simulink model "SimulinkAnalysisofCheetahTail"  (R2022a)
(part 5 of 21)

C = ft_9({B_cg_H,ITail,Mb,Mm,Mt,T_cg_H,dphi1,dphi2,dpsi1,dth1,dth2,dx,dy,dz,t10,t1003,t1005,t1006,t1007,t1008,t1009,t1013,t1014,t1015,t1016,t1017,t1018,t1019,t1020,t1023,t1029,t103,t1031,t1037,t1042,t1044,t1047,t105,t1050,t1051,t1052,t1053,t1054,t1059,t1060,t1064,t1065,t1067,t1068,t1071,t1072,t1073,t1074,t1075,t1076,t1077,t1078,t1079,t1082,t1084,t1086,t1088,t1097,t1099,t11,t1102,t1108,t1113,t1115,t1116,t1117,t1118,t1119,t1120,t1121,t1122,t1123,t1124,t1129,t1132,t1133,t1134,t1135,t1136,t1137,t1138,t1139,t1140,t1141,t1142,t1143,t1144,t1146,t1147,t1149,t1153,t1155,t1156,t1157,t1159,t1160,t1161,t1162,t1163,t1164,t1166,t1167,t1168,t1169,t1170,t1171,t1173,t1174,t1176,t1178,t1179,t1181,t1182,t1183,t1184,t1185,t1186,t1187,t1188,t1189,t1190,t1191,t1192,t1193,t1194,t1195,t1196,t1197,t120,t1200,t1201,t1202,t1203,t1205,t1206,t1211,t1212,t1213,t1214,t1215,t1220,t1221,t1223,t1224,t1225,t1228,t1229,t1230,t1234,t1236,t1237,t1240,t1242,t1243,t1244,t1245,t1246,t1247,t1248,t1250,t1251,t1252,t1253,t1255,t1256,t1260,t1261,t1262,t1263,t1264,t1265,t1268,t1271,t1275,t1280,t1283,t1285,t1291,t1296,t1299,t130,t1301,t1302,t1303,t1304,t1305,t1306,t1307,t1309,t1311,t1312,t1313,t1319,t1322,t1328,t1329,t1331,t1332,t1334,t1337,t1338,t1339,t134,t1341,t1343,t1344,t1345,t1348,t1349,t1352,t1354,t1355,t1356,t1357,t1358,t1360,t1361,t1362,t1365,t1366,t1368,t1370,t1371,t1373,t1374,t1378,t1379,t1380,t1381,t1382,t1383,t1384,t1386,t1388,t1389,t1391,t1393,t1394,t1395,t1396,t1397,t1399,t1402,t1403,t1405,t1406,t1407,t1410,t1412,t1413,t1414,t1415,t1416,t1418,t1421,t1422,t1423,t1426,t1427,t1430,t1431,t1433,t1435,t1438,t144,t1440,t1441,t1443,t1444,t1446,t1448,t1450,t1453,t1455,t1456,t1457,t1458,t1459,t1460,t1463,t1465,t1466,t1467,t1468,t1469,t1470,t1473,t1476,t1477,t1478,t1479,t1480,t1481,t1483,t1484,t1486,t1487,t1488,t1489,t1491,t1495,t1496,t1497,t1498,t15,t1500,t1505,t1506,t1508,t1509,t1510,t1512,t1513,t1516,t1517,t1518,t1521,t1523,t1525,t1526,t1528,t1529,t1531,t1535,t1540,t1543,t1544,t1546,t1548,t1549,t1550,t1551,t1552,t1553,t1555,t1558,t1562,t1563,t1565,t1566,t1567,t1568,t1574,t1575,t1578,t1579,t1581,t1582,t1585,t1586,t1587,t1589,t1590,t1591,t1593,t1594,t1595,t1596,t1597,t1598,t1599,t1601,t1602,t1605,t1606,t1609,t161,t1610,t1611,t1612,t1614,t1615,t1617,t1618,t1619,t162,t1620,t1621,t1622,t1623,t1624,t1627,t1628,t1630,t1631,t1632,t1633,t1634,t1635,t1636,t1637,t1639,t1640,t1641,t1642,t1643,t1644,t1645,t1646,t1649,t1651,t1652,t1653,t1654,t1655,t1656,t1657,t1658,t1659,t1660,t1661,t1663,t1664,t1665,t1667,t1668,t1669,t1671,t1672,t1674,t1675,t1676,t1677,t1678,t1679,t1680,t1681,t1682,t1683,t1684,t1685,t1686,t1687,t1688,t1689,t1690,t1691,t1692,t1693,t1694,t1695,t1696,t1698,t1699,t1700,t1701,t1702,t1703,t1705,t1706,t1711,t1716,t1718,t1719,t1720,t1721,t1722,t1723,t1725,t1726,t1727,t1729,t1730,t1731,t1734,t1735,t1736,t1737,t1739,t1740,t1741,t1742,t1743,t1744,t1745,t1746,t1747,t1748,t1749,t1750,t1751,t1752,t1753,t1755,t1756,t1758,t1759,t1761,t1762,t1763,t1764,t1765,t1770,t1771,t1774,t1777,t1778,t1779,t1780,t1781,t1782,t1783,t1784,t1785,t1786,t1787,t1788,t1789,t1790,t1791,t1792,t1798,t1799,t1800,t1801,t1802,t1806,t1809,t1810,t1813,t1814,t1815,t1817,t1820,t1821,t1822,t1823,t1824,t1826,t1828,t1829,t1830,t1831,t1832,t1836,t1839,t1840,t1841,t1843,t1844,t1845,t1846,t1847,t1849,t1851,t1852,t1853,t1855,t1857,t1858,t1859,t1860,t1862,t1863,t1864,t1865,t1866,t1867,t1869,t1870,t1871,t1872,t1874,t1875,t1878,t1880,t1881,t1882,t1883,t1884,t1885,t1887,t1888,t1890,t1891,t1893,t1894,t1895,t1896,t1898,t1899,t1900,t1902,t1904,t1905,t1906,t1907,t1908,t1909,t1910,t1911,t1912,t1914,t1915,t1916,t1917,t1918,t1921,t1922,t1924,t1928,t1929,t1930,t1931,t1932,t1937,t1938,t1939,t1940,t1941,t1942,t1943,t1945,t1946,t1947,t1948,t1949,t195,t1950,t1951,t1952,t1955,t1956,t1957,t1959,t1960,t1961,t1962,t1963,t1964,t1965,t1966,t1967,t1968,t1969,t197,t1970,t1971,t1973,t1974,t1975,t1976,t1977,t1978,t1979,t1980,t1981,t1982,t1983,t1985,t1986,t1989,t1990,t1991,t1993,t1995,t1997,t1998,t1999,t2,t2000,t2001,t2002,t2003,t2004,t2005,t2006,t2007,t2008,t2009,t2010,t2011,t2012,t2013,t2015,t2016,t2017,t2018,t2019,t2020,t2023,t2024,t2025,t2026,t2032,t2033,t2035,t2037,t2038,t2039,t2040,t2041,t2042,t2043,t2045,t2046,t2047,t2048,t2049,t2050,t2053,t2057,t2058,t2059,t2061,t2062,t2064,t2065,t2066,t2067,t2068,t2069,t2070,t2072,t2073,t2074,t2075,t2076,t2078,t2079,t2080,t2081,t2082,t2083,t2084,t2085,t2087,t2088,t2090,t2091,t2093,t2094,t2095,t2096,t2097,t2101,t2102,t2103,t2104,t2106,t2107,t2108,t2109,t2110,t2111,t2112,t2113,t2115,t2117,t2118,t2119,t2120,t2122,t2123,t2124,t2125,t2127,t2128,t2129,t2130,t2131,t2132,t2134,t2135,t2137,t2138,t2139,t214,t2141,t2143,t2144,t2147,t2148,t2150,t2151,t2152,t2153,t2154,t2155,t2156,t2157,t2158,t2160,t2161,t2162,t2165,t2169,t2170,t2171,t2172,t2173,t2174,t2175,t2176,t2177,t2178,t2179,t2181,t2182,t2183,t2186,t2188,t2189,t2190,t2191,t2192,t2193,t2194,t2195,t2196,t2197,t2198,t2199,t2200,t2201,t2202,t2203,t2205,t2206,t2208,t2209,t2210,t2211,t2212,t2213,t2214,t2215,t2216,t2217,t2218,t2219,t2220,t2221,t2222,t2223,t2224,t2225,t2227,t2229,t2230,t2232,t2233,t2234,t2235,t2236,t2237,t2238,t2240,t2241,t2242,t2243,t2244,t2245,t2246,t2247,t2248,t2249,t2250,t2251,t2252,t2253,t2254,t2255,t2257,t2258,t2259,t2260,t2262,t2263,t2268,t2269,t2270,t2271,t2274,t2276,t2277,t2279,t2281,t2282,t2284,t2285,t2286,t2287,t2288,t2289,t2290,t2293,t2294,t2296,t2298,t2299,t2303,t2304,t2305,t2307,t2308,t2312,t2313,t2316,t2317,t2318,t2319,t2320,t2321,t2322,t2323,t2324,t2325,t2329,t2330,t2332,t2333,t2334,t2335,t2336,t2338,t2339,t2340,t2341,t2342,t2343,t2345,t2346,t2347,t2348,t2349,t2350,t2351,t2352,t2354,t2355,t2356,t2358,t2360,t2361,t2362,t2363,t2364,t2368,t2369,t2370,t2371,t2376,t2380,t2381,t2382,t2385,t2386,t2387,t2388,t2389,t2390,t2391,t2392,t2397,t2399,t24,t2400,t2401,t2403,t2404,t2406,t2407,t2408,t2409,t2410,t2411,t2412,t2413,t2416,t2417,t2419,t2420,t2422,t2423,t2425,t2426,t2427,t2428,t2429,t2430,t2431,t2433,t2434,t2435,t2436,t2437,t2438,t2439,t2445,t2447,t2448,t2449,t2450,t2451,t2453,t2454,t2455,t2457,t2458,t2459,t2460,t2461,t2462,t2463,t2464,t2465,t2467,t2468,t2469,t2470,t2471,t2472,t2474,t2476,t2479,t2480,t2483,t2484,t2485,t2486,t2487,t2488,t2489,t2492,t2495,t2496,t2498,t25,t2501,t2502,t2503,t2504,t2505,t2506,t2511,t2512,t2513,t2514,t2515,t2516,t2518,t2519,t2521,t2522,t2523,t2524,t2525,t2526,t2527,t2528,t2529,t2530,t2531,t2532,t2533,t2534,t2535,t2536,t2537,t2538,t2539,t2541,t2542,t2543,t2544,t2545,t2546,t2547,t2548,t2549,t2550,t2551,t2552,t2554,t2555,t2558,t2559,t2560,t2561,t2562,t2563,t2564,t2565,t2566,t2567,t2568,t2569,t2570,t2571,t2573,t2574,t2575,t2576,t2577,t2578,t2579,t2581,t2582,t2583,t2584,t2585,t2587,t2588,t2589,t259,t2590,t2591,t2595,t2597,t2598,t2599,t26,t260,t2600,t2601,t2602,t2605,t2606,t2607,t2609,t2610,t2611,t2613,t2615,t2616,t2617,t2619,t2620,t2621,t2623,t2624,t2627,t2629,t2630,t2632,t2634,t2635,t2636,t2637,t2638,t2639,t2640,t2641,t2644,t2645,t2646,t2647,t2648,t2649,t2650,t2651,t2652,t2654,t2656,t2657,t2658,t2660,t2661,t2662,t2663,t2665,t2666,t2667,t2668,t2669,t2671,t2672,t2673,t2674,t2675,t2676,t2677,t2678,t2679,t2682,t2684,t2685,t2688,t2689,t2691,t2692,t2696,t2698,t2699,t27,t2700,t2705,t2706,t2707,t2708,t2710,t2712,t2714,t2715,t2717,t2718,t2722,t2723,t2725,t2726,t2727,t2728,t2730,t2731,t2732,t2733,t2734,t2735,t2736,t2737,t2738,t2740,t2741,t2742,t2743,t2744,t2746,t2748,t2749,t2750,t2751,t2752,t2754,t2755,t2756,t2758,t2759,t276,t2760,t2761,t2763,t2764,t2765,t2766,t2767,t2768,t2769,t277,t2771,t2772,t2774,t2775,t2776,t2778,t2779,t2780,t2781,t2782,t2783,t2785,t2786,t2787,t2788,t2790,t2791,t2792,t2793,t2794,t2796,t2797,t2798,t2799,t2800,t2802,t2803,t2804,t2805,t2806,t2807,t2811,t2813,t2814,t2816,t2817,t2818,t2819,t2821,t2823,t2824,t2825,t2828,t2829,t283,t2830,t2831,t2832,t2833,t2834,t2835,t2836,t2837,t2838,t2839,t284,t2841,t2842,t2843,t2844,t2845,t2846,t2847,t2848,t2849,t285,t2852,t2853,t2857,t2858,t2859,t286,t2860,t2861,t2864,t2865,t2866,t2867,t2868,t287,t2870,t2871,t2872,t2874,t2875,t2876,t2877,t2878,t2879,t288,t2880,t2882,t2883,t2884,t2886,t2887,t2889,t289,t2890,t2892,t2893,t2895,t2896,t2897,t2898,t2899,t290,t2901,t2902,t2903,t2904,t2905,t2906,t2907,t2909,t291,t2912,t2913,t2914,t2915,t2916,t2917,t2918,t2919,t292,t2920,t2921,t2922,t2924,t2926,t2927,t2928,t2929,t293,t2930,t2932,t2934,t2935,t2936,t2937,t2938,t2939,t294,t2940,t2941,t2942,t2943,t2944,t2945,t2946,t2949,t2950,t2952,t2954,t2955,t2956,t2957,t2959,t2960,t2961,t2962,t2963,t2964,t2965,t2966,t2967,t2969,t2970,t2971,t2972,t2975,t2976,t2977,t2978,t2979,t2981,t2982,t2985,t2986,t2987,t2988,t2989,t2992,t2994,t2995,t2996,t2997,t2998,t2999,t3,t30,t3000,t3003,t3004,t3006,t3007,t3008,t3009,t3010,t3011,t3012,t3016,t3017,t3019,t3022,t3027,t3030,t3031,t3032,t3033,t3034,t3035,t3037,t3038,t3039,t304,t3041,t3042,t3043,t3047,t3049,t3050,t3051,t3054,t3059,t3060,t3061,t3062,t3063,t3064,t3065,t3066,t3069,t3070,t3072,t3074,t3075,t3076,t3077,t3078,t3080,t3082,t3083,t3084,t3085,t3086,t3087,t3089,t3090,t3091,t3092,t3093,t3094,t3096,t3097,t3098,t3099,t3100,t3102,t3103,t3104,t3105,t3106,t3107,t3108,t3109,t3110,t3112,t3113,t3114,t3115,t3117,t3119,t3121,t3122,t3123,t3124,t3127,t3128,t3130,t3131,t3132,t3133,t3134,t3135,t3136,t3138,t3139,t3145,t3146,t3147,t3149,t3151,t3153,t3155,t3156,t3157,t3158,t3160,t3161,t3162,t3163,t3164,t3165,t3166,t3167,t3168,t3169,t3170,t3171,t3173,t3174,t3175,t3176,t3177,t3178,t3179,t3180,t3181,t3183,t3184,t3185,t3186,t3187,t3189,t3192,t3195,t3196,t3197,t3198,t3199,t3200,t3203,t3204,t3206,t3207,t3210,t3212,t3213,t3214,t3215,t3216,t3217,t3218,t3219,t3220,t3221,t3222,t3223,t3224,t3226,t3227,t3230,t3231,t3232,t3233,t3234,t3235,t3236,t3238,t3239,t3240,t3241,t3243,t3244,t3245,t3247,t3248,t3250,t3251,t3252,t3254,t3256,t3258,t3260,t3261,t3262,t3263,t3265,t3266,t3267,t3270,t3271,t3272,t3273,t3276,t3277,t3278,t3279,t3280,t3281,t3282,t3284,t3285,t3286,t3287,t3288,t3289,t3290,t3291,t3292,t3293,t3296,t3299,t33,t3300,t3301,t3302,t3303,t3304,t3305,t3306,t3307,t3308,t3311,t3312,t3313,t3314,t3315,t3316,t3317,t3319,t3320,t3321,t3322,t3323,t3324,t3325,t3326,t3327,t3330,t3331,t3332,t3333,t3334,t3337,t3338,t3339,t3340,t3341,t3342,t3343,t3347,t3348,t3349,t3351,t3352,t3353,t3354,t3355,t3356,t3357,t3359,t3360,t3361,t3365,t3366,t3367,t3368,t3370,t3372,t3373,t3375,t3376,t3377,t3378,t3379,t3380,t3381,t3382,t3384,t3385,t3386,t3387,t3388,t3390,t3391,t3392,t3393,t3396,t3397,t3398,t3399,t34,t3400,t3401,t3403,t3404,t3405,t3406,t3407,t3408,t3409,t3410,t3412,t3413,t3414,t3415,t3416,t3419,t3420,t3421,t3423,t3424,t3425,t3426,t3427,t3429,t3430,t3431,t3432,t3433,t3434,t3437,t3438,t3439,t3440,t3441,t3442,t3443,t3444,t3445,t3446,t3447,t3448,t3449,t3450,t3452,t3453,t3454,t3455,t3456,t3457,t3458,t3459,t3460,t3462,t3463,t3464,t3465,t3466,t3467,t3468,t3469,t3470,t3471,t3472,t3474,t3475,t3476,t3477,t3478,t3479,t3480,t3481,t3483,t3484,t3485,t3486,t3487,t3488,t3489,t3490,t3491,t3492,t3494,t3495,t3496,t3497,t3499,t3500,t3501,t3502,t3504,t3506,t3508,t3509,t3510,t3511,t3512,t3513,t3515,t3516,t3517,t3518,t3521,t3522,t3523,t3524,t3526,t3528,t3529,t3530,t3531,t3532,t3533,t3534,t3535,t3536,t3537,t3538,t3539,t3541,t3542,t3543,t3544,t3545,t3547,t3548,t3550,t3551,t3552,t3553,t3554,t3556,t3557,t3558,t3559,t3562,t3563,t3564,t3565,t3569,t3570,t3571,t3575,t3576,t3578,t3579,t3581,t3582,t3583,t3584,t3587,t3588,t3591,t3593,t3594,t3595,t3596,t3597,t3598,t3599,t3600,t3601,t3602,t3603,t3604,t3605,t3606,t3607,t3608,t3609,t3610,t3611,t3613,t3614,t3615,t3616,t3617,t3618,t3619,t3620,t3621,t3622,t3623,t3624,t3625,t3626,t3627,t3629,t3630,t3631,t3632,t3634,t3635,t3636,t3637,t3638,t3639,t3640,t3641,t3643,t3644,t3645,t3646,t3647,t3648,t3649,t3651,t3652,t3653,t3654,t3655,t3656,t3657,t3658,t3659,t3660,t3661,t3664,t3665,t3666,t3667,t3668,t3669,t3671,t3672,t3673,t3674,t3675,t3676,t3677,t3678,t3679,t3680,t3681,t3682,t3683,t3684,t3685,t3686,t3687,t3688,t3689,t3691,t3692,t3693,t3695,t3697,t3698,t3699,t3700,t3701,t3702,t3704,t3708,t3709,t3710,t3711,t3712,t3713,t3716,t3717,t3719,t3720,t3721,t3722,t3723,t3724,t3725,t3726,t3729,t3730,t3732,t3733,t3735,t3736,t3737,t3739,t3741,t3742,t3744,t3745,t3746,t3747,t3749,t3750,t3751,t3752,t3753,t3754,t3756,t3757,t3759,t376,t3760,t3761,t3762,t3763,t3764,t3765,t3767,t3768,t3769,t377,t3770,t3771,t3772,t3773,t3774,t3775,t3776,t3777,t3778,t3779,t3780,t3783,t3784,t3785,t3786,t3787,t3789,t3790,t3791,t3792,t3793,t3794,t3795,t3796,t3799,t38,t3802,t3803,t3804,t3805,t3806,t3807,t3808,t3809,t381,t3810,t3811,t3812,t3813,t3814,t3815,t3817,t3818,t3819,t382,t3820,t3823,t3826,t3828,t3829,t383,t3831,t3832,t3833,t3834,t3836,t3837,t3838,t3840,t3841,t3842,t3843,t3844,t3845,t3846,t3847,t3848,t3849,t3850,t3851,t3854,t3855,t3856,t3857,t3858,t3859,t3862,t3864,t3865,t3866,t3867,t3868,t3870,t3871,t3872,t3873,t3879,t3880,t3882,t3883,t3884,t3886,t3887,t3888,t3889,t3890,t3894,t3896,t3897,t3898,t3899,t390,t3900,t3901,t3902,t3903,t3906,t3907,t3908,t3909,t3910,t3911,t3913,t3914,t3915,t3916,t3918,t3919,t3921,t3922,t3923,t3926,t3928,t3929,t3930,t3931,t3932,t3933,t3934,t3935,t3936,t3937,t3938,t3939,t394,t3940,t3941,t3942,t3944,t3946,t3947,t3948,t3949,t3950,t3951,t3952,t3953,t3954,t3955,t3956,t3957,t3958,t3959,t3960,t3961,t3962,t3964,t3965,t3966,t3967,t3969,t3970,t3971,t3974,t3975,t3976,t3978,t3979,t3980,t3981,t3982,t3983,t3984,t3985,t3986,t3987,t3991,t3992,t3993,t3994,t3995,t3996,t3997,t3998,t4,t4000,t4001,t4003,t4005,t4007,t4008,t4009,t4010,t4011,t4012,t4013,t4014,t4015,t4019,t4020,t4021,t4022,t4023,t4024,t4025,t4026,t4027,t4028,t4029,t4030,t4031,t4032,t4033,t4034,t4035,t4036,t4038,t4040,t4041,t4042,t4043,t4046,t4047,t4048,t4050,t4051,t4052,t4053,t4054,t4056,t4058,t4059,t4061,t4063,t4064,t4065,t4066,t4068,t4070,t4071,t4072,t4073,t4074,t4077,t4078,t4081,t4083,t4084,t4085,t4086,t4087,t4089,t4090,t4092,t4093,t4094,t4095,t4096,t4097,t4098,t4099,t41,t410,t4100,t4101,t4104,t4105,t4108,t4109,t411,t4111,t4112,t4115,t4116,t4117,t4119,t412,t4120,t4121,t4122,t4123,t4126,t4128,t4129,t413,t4130,t4131,t4132,t4133,t4135,t4137,t4138,t4139,t414,t4140,t4141,t4143,t4144,t4145,t4146,t4147,t415,t4151,t4152,t4153,t4155,t4156,t4157,t4158,t4159,t4160,t4162,t4164,t4165,t4166,t4168,t4169,t4171,t4173,t4174,t4176,t4177,t4178,t4179,t4182,t4184,t4187,t4188,t4189,t4190,t4191,t4192,t4193,t4194,t4196,t4197,t4199,t420,t4201,t4203,t4204,t4206,t421,t4210,t4211,t4212,t4213,t4214,t4215,t4216,t4217,t4218,t4220,t4221,t4222,t4223,t4224,t4225,t4226,t4227,t4228,t4229,t4230,t4231,t4232,t4233,t4234,t4236,t4237,t4239,t4240,t4241,t4244,t4245,t4246,t4247,t4248,t4249,t425,t4250,t4252,t4253,t4255,t4256,t4258,t4259,t4261,t4262,t4263,t4264,t4267,t4268,t4269,t4272,t4273,t4274,t4276,t4277,t4278,t4280,t4281,t4282,t4286,t4290,t4295,t4298,t4299,t430,t4300,t4301,t4304,t4305,t4306,t4307,t4308,t431,t4311,t4312,t4316,t4320,t4323,t4324,t4326,t433,t4330,t4332,t4333,t4334,t4339,t4342,t4344,t4345,t4346,t4348,t4349,t4351,t4354,t4355,t4356,t4358,t436,t4360,t4361,t4364,t4365,t4367,t4368,t4371,t4372,t4375,t4382,t4393,t4395,t4399,t44,t4402,t4406,t4408,t4414,t4416,t4418,t4420,t4421,t4422,t4423,t4424,t4425,t4427,t4428,t4432,t4436,t4437,t4438,t4440,t4441,t4449,t445,t4453,t4454,t4457,t4458,t4461,t4467,t4468,t4469,t4472,t4475,t4476,t4477,t4478,t4479,t4481,t4486,t4487,t4488,t4490,t4492,t4494,t4495,t4496,t4497,t4506,t451,t4512,t4514,t4516,t4525,t4529,t4538,t4545,t4549,t4551,t4552,t4558,t4561,t4569,t4571,t4575,t4581,t4583,t459,t4597,t4598,t4602,t4603,t4611,t4616,t4628,t4641,t4646,t4649,t465,t4655,t4659,t4665,t4686,t4695,t4707,t4709,t4711,t4713,t4722,t4723,t4724,t4732,t4733,t4735,t4736,t4740,t4745,t4746,t4752,t4762,t4772,t4776,t4784,t4789,t4796,t48,t4802,t4809,t4821,t4823,t483,t4848,t4849,t485,t4866,t487,t4873,t4878,t488,t4889,t4895,t49,t4909,t491,t4913,t4922,t4923,t4925,t4931,t4932,t4933,t4936,t4938,t4942,t4944,t4945,t4946,t4953,t4954,t496,t4964,t4966,t4967,t4975,t4976,t4986,t4987,t4988,t4993,t4995,t5,t50,t501,t502,t5021,t5032,t5036,t504,t5042,t5046,t5051,t5053,t5054,t5058,t5059,t5066,t5067,t5072,t5078,t5080,t5083,t5092,t51,t5103,t5109,t5153,t5179,t519,t5198,t5202,t5206,t5208,t5227,t523,t524,t5265,t527,t5275,t530,t5300,t5317,t534,t5351,t5358,t5363,t537,t539,t5399,t54,t541,t542,t5420,t5424,t5427,t5431,t5433,t5438,t544,t5448,t5453,t546,t5476,t5488,t5498,t55,t550,t553,t5530,t5539,t5547,t5565,t557,t5576,t558,t5582,t5598,t56,t5674,t5690,t5705,t5706,t5716,t573,t574,t575,t5788,t5791,t5800,t5869,t587,t59,t595,t603,t61,t614,t628,t629,t634,t641,t65,t650,t651,t655,t6554,t6556,t657,t6599,t6627,t6629,t664,t665,t666,t667,t668,t669,t675,t68,t693,t7,t71,t721,t724,t73,t731,t732,t736,t741,t744,t753,t754,t755,t756,t757,t759,t760,t761,t762,t764,t765,t769,t772,t774,t776,t778,t792,t795,t797,t799,t8,t802,t803,t806,t817,t818,t820,t824,t828,t831,t834,t837,t838,t841,t842,t843,t844,t846,t847,t848,t850,t851,t852,t853,t855,t865,t867,t868,t870,t871,t872,t874,t875,t876,t877,t885,t886,t888,t890,t891,t892,t896,t898,t9,t901,t902,t903,t904,t906,t907,t909,t914,t915,t916,t924,t925,t926,t928,t947,t949,t950,t952,t954,t955,t957,t964,t965,t972,t977,t979,t983,t987,t991,t992,t993,t994,t995});
end
function C = ft_9(ct)
B_cg_H = ct{1};
ITail = ct{2};
Mb = ct{3};
Mm = ct{4};
Mt = ct{5};
T_cg_H = ct{6};
dphi1 = ct{7};
dphi2 = ct{8};
dpsi1 = ct{9};
dth1 = ct{10};
dth2 = ct{11};
dx = ct{12};
dy = ct{13};
dz = ct{14};
t10 = ct{15};
t1003 = ct{16};
t1005 = ct{17};
t1006 = ct{18};
t1007 = ct{19};
t1008 = ct{20};
t1009 = ct{21};
t1013 = ct{22};
t1014 = ct{23};
t1015 = ct{24};
t1016 = ct{25};
t1017 = ct{26};
t1018 = ct{27};
t1019 = ct{28};
t1020 = ct{29};
t1023 = ct{30};
t1029 = ct{31};
t103 = ct{32};
t1031 = ct{33};
t1037 = ct{34};
t1042 = ct{35};
t1044 = ct{36};
t1047 = ct{37};
t105 = ct{38};
t1050 = ct{39};
t1051 = ct{40};
t1052 = ct{41};
t1053 = ct{42};
t1054 = ct{43};
t1059 = ct{44};
t1060 = ct{45};
t1064 = ct{46};
t1065 = ct{47};
t1067 = ct{48};
t1068 = ct{49};
t1071 = ct{50};
t1072 = ct{51};
t1073 = ct{52};
t1074 = ct{53};
t1075 = ct{54};
t1076 = ct{55};
t1077 = ct{56};
t1078 = ct{57};
t1079 = ct{58};
t1082 = ct{59};
t1084 = ct{60};
t1086 = ct{61};
t1088 = ct{62};
t1097 = ct{63};
t1099 = ct{64};
t11 = ct{65};
t1102 = ct{66};
t1108 = ct{67};
t1113 = ct{68};
t1115 = ct{69};
t1116 = ct{70};
t1117 = ct{71};
t1118 = ct{72};
t1119 = ct{73};
t1120 = ct{74};
t1121 = ct{75};
t1122 = ct{76};
t1123 = ct{77};
t1124 = ct{78};
t1129 = ct{79};
t1132 = ct{80};
t1133 = ct{81};
t1134 = ct{82};
t1135 = ct{83};
t1136 = ct{84};
t1137 = ct{85};
t1138 = ct{86};
t1139 = ct{87};
t1140 = ct{88};
t1141 = ct{89};
t1142 = ct{90};
t1143 = ct{91};
t1144 = ct{92};
t1146 = ct{93};
t1147 = ct{94};
t1149 = ct{95};
t1153 = ct{96};
t1155 = ct{97};
t1156 = ct{98};
t1157 = ct{99};
t1159 = ct{100};
t1160 = ct{101};
t1161 = ct{102};
t1162 = ct{103};
t1163 = ct{104};
t1164 = ct{105};
t1166 = ct{106};
t1167 = ct{107};
t1168 = ct{108};
t1169 = ct{109};
t1170 = ct{110};
t1171 = ct{111};
t1173 = ct{112};
t1174 = ct{113};
t1176 = ct{114};
t1178 = ct{115};
t1179 = ct{116};
t1181 = ct{117};
t1182 = ct{118};
t1183 = ct{119};
t1184 = ct{120};
t1185 = ct{121};
t1186 = ct{122};
t1187 = ct{123};
t1188 = ct{124};
t1189 = ct{125};
t1190 = ct{126};
t1191 = ct{127};
t1192 = ct{128};
t1193 = ct{129};
t1194 = ct{130};
t1195 = ct{131};
t1196 = ct{132};
t1197 = ct{133};
t120 = ct{134};
t1200 = ct{135};
t1201 = ct{136};
t1202 = ct{137};
t1203 = ct{138};
t1205 = ct{139};
t1206 = ct{140};
t1211 = ct{141};
t1212 = ct{142};
t1213 = ct{143};
t1214 = ct{144};
t1215 = ct{145};
t1220 = ct{146};
t1221 = ct{147};
t1223 = ct{148};
t1224 = ct{149};
t1225 = ct{150};
t1228 = ct{151};
t1229 = ct{152};
t1230 = ct{153};
t1234 = ct{154};
t1236 = ct{155};
t1237 = ct{156};
t1240 = ct{157};
t1242 = ct{158};
t1243 = ct{159};
t1244 = ct{160};
t1245 = ct{161};
t1246 = ct{162};
t1247 = ct{163};
t1248 = ct{164};
t1250 = ct{165};
t1251 = ct{166};
t1252 = ct{167};
t1253 = ct{168};
t1255 = ct{169};
t1256 = ct{170};
t1260 = ct{171};
t1261 = ct{172};
t1262 = ct{173};
t1263 = ct{174};
t1264 = ct{175};
t1265 = ct{176};
t1268 = ct{177};
t1271 = ct{178};
t1275 = ct{179};
t1280 = ct{180};
t1283 = ct{181};
t1285 = ct{182};
t1291 = ct{183};
t1296 = ct{184};
t1299 = ct{185};
t130 = ct{186};
t1301 = ct{187};
t1302 = ct{188};
t1303 = ct{189};
t1304 = ct{190};
t1305 = ct{191};
t1306 = ct{192};
t1307 = ct{193};
t1309 = ct{194};
t1311 = ct{195};
t1312 = ct{196};
t1313 = ct{197};
t1319 = ct{198};
t1322 = ct{199};
t1328 = ct{200};
t1329 = ct{201};
t1331 = ct{202};
t1332 = ct{203};
t1334 = ct{204};
t1337 = ct{205};
t1338 = ct{206};
t1339 = ct{207};
t134 = ct{208};
t1341 = ct{209};
t1343 = ct{210};
t1344 = ct{211};
t1345 = ct{212};
t1348 = ct{213};
t1349 = ct{214};
t1352 = ct{215};
t1354 = ct{216};
t1355 = ct{217};
t1356 = ct{218};
t1357 = ct{219};
t1358 = ct{220};
t1360 = ct{221};
t1361 = ct{222};
t1362 = ct{223};
t1365 = ct{224};
t1366 = ct{225};
t1368 = ct{226};
t1370 = ct{227};
t1371 = ct{228};
t1373 = ct{229};
t1374 = ct{230};
t1378 = ct{231};
t1379 = ct{232};
t1380 = ct{233};
t1381 = ct{234};
t1382 = ct{235};
t1383 = ct{236};
t1384 = ct{237};
t1386 = ct{238};
t1388 = ct{239};
t1389 = ct{240};
t1391 = ct{241};
t1393 = ct{242};
t1394 = ct{243};
t1395 = ct{244};
t1396 = ct{245};
t1397 = ct{246};
t1399 = ct{247};
t1402 = ct{248};
t1403 = ct{249};
t1405 = ct{250};
t1406 = ct{251};
t1407 = ct{252};
t1410 = ct{253};
t1412 = ct{254};
t1413 = ct{255};
t1414 = ct{256};
t1415 = ct{257};
t1416 = ct{258};
t1418 = ct{259};
t1421 = ct{260};
t1422 = ct{261};
t1423 = ct{262};
t1426 = ct{263};
t1427 = ct{264};
t1430 = ct{265};
t1431 = ct{266};
t1433 = ct{267};
t1435 = ct{268};
t1438 = ct{269};
t144 = ct{270};
t1440 = ct{271};
t1441 = ct{272};
t1443 = ct{273};
t1444 = ct{274};
t1446 = ct{275};
t1448 = ct{276};
t1450 = ct{277};
t1453 = ct{278};
t1455 = ct{279};
t1456 = ct{280};
t1457 = ct{281};
t1458 = ct{282};
t1459 = ct{283};
t1460 = ct{284};
t1463 = ct{285};
t1465 = ct{286};
t1466 = ct{287};
t1467 = ct{288};
t1468 = ct{289};
t1469 = ct{290};
t1470 = ct{291};
t1473 = ct{292};
t1476 = ct{293};
t1477 = ct{294};
t1478 = ct{295};
t1479 = ct{296};
t1480 = ct{297};
t1481 = ct{298};
t1483 = ct{299};
t1484 = ct{300};
t1486 = ct{301};
t1487 = ct{302};
t1488 = ct{303};
t1489 = ct{304};
t1491 = ct{305};
t1495 = ct{306};
t1496 = ct{307};
t1497 = ct{308};
t1498 = ct{309};
t15 = ct{310};
t1500 = ct{311};
t1505 = ct{312};
t1506 = ct{313};
t1508 = ct{314};
t1509 = ct{315};
t1510 = ct{316};
t1512 = ct{317};
t1513 = ct{318};
t1516 = ct{319};
t1517 = ct{320};
t1518 = ct{321};
t1521 = ct{322};
t1523 = ct{323};
t1525 = ct{324};
t1526 = ct{325};
t1528 = ct{326};
t1529 = ct{327};
t1531 = ct{328};
t1535 = ct{329};
t1540 = ct{330};
t1543 = ct{331};
t1544 = ct{332};
t1546 = ct{333};
t1548 = ct{334};
t1549 = ct{335};
t1550 = ct{336};
t1551 = ct{337};
t1552 = ct{338};
t1553 = ct{339};
t1555 = ct{340};
t1558 = ct{341};
t1562 = ct{342};
t1563 = ct{343};
t1565 = ct{344};
t1566 = ct{345};
t1567 = ct{346};
t1568 = ct{347};
t1574 = ct{348};
t1575 = ct{349};
t1578 = ct{350};
t1579 = ct{351};
t1581 = ct{352};
t1582 = ct{353};
t1585 = ct{354};
t1586 = ct{355};
t1587 = ct{356};
t1589 = ct{357};
t1590 = ct{358};
t1591 = ct{359};
t1593 = ct{360};
t1594 = ct{361};
t1595 = ct{362};
t1596 = ct{363};
t1597 = ct{364};
t1598 = ct{365};
t1599 = ct{366};
t1601 = ct{367};
t1602 = ct{368};
t1605 = ct{369};
t1606 = ct{370};
t1609 = ct{371};
t161 = ct{372};
t1610 = ct{373};
t1611 = ct{374};
t1612 = ct{375};
t1614 = ct{376};
t1615 = ct{377};
t1617 = ct{378};
t1618 = ct{379};
t1619 = ct{380};
t162 = ct{381};
t1620 = ct{382};
t1621 = ct{383};
t1622 = ct{384};
t1623 = ct{385};
t1624 = ct{386};
t1627 = ct{387};
t1628 = ct{388};
t1630 = ct{389};
t1631 = ct{390};
t1632 = ct{391};
t1633 = ct{392};
t1634 = ct{393};
t1635 = ct{394};
t1636 = ct{395};
t1637 = ct{396};
t1639 = ct{397};
t1640 = ct{398};
t1641 = ct{399};
t1642 = ct{400};
t1643 = ct{401};
t1644 = ct{402};
t1645 = ct{403};
t1646 = ct{404};
t1649 = ct{405};
t1651 = ct{406};
t1652 = ct{407};
t1653 = ct{408};
t1654 = ct{409};
t1655 = ct{410};
t1656 = ct{411};
t1657 = ct{412};
t1658 = ct{413};
t1659 = ct{414};
t1660 = ct{415};
t1661 = ct{416};
t1663 = ct{417};
t1664 = ct{418};
t1665 = ct{419};
t1667 = ct{420};
t1668 = ct{421};
t1669 = ct{422};
t1671 = ct{423};
t1672 = ct{424};
t1674 = ct{425};
t1675 = ct{426};
t1676 = ct{427};
t1677 = ct{428};
t1678 = ct{429};
t1679 = ct{430};
t1680 = ct{431};
t1681 = ct{432};
t1682 = ct{433};
t1683 = ct{434};
t1684 = ct{435};
t1685 = ct{436};
t1686 = ct{437};
t1687 = ct{438};
t1688 = ct{439};
t1689 = ct{440};
t1690 = ct{441};
t1691 = ct{442};
t1692 = ct{443};
t1693 = ct{444};
t1694 = ct{445};
t1695 = ct{446};
t1696 = ct{447};
t1698 = ct{448};
t1699 = ct{449};
t1700 = ct{450};
t1701 = ct{451};
t1702 = ct{452};
t1703 = ct{453};
t1705 = ct{454};
t1706 = ct{455};
t1711 = ct{456};
t1716 = ct{457};
t1718 = ct{458};
t1719 = ct{459};
t1720 = ct{460};
t1721 = ct{461};
t1722 = ct{462};
t1723 = ct{463};
t1725 = ct{464};
t1726 = ct{465};
t1727 = ct{466};
t1729 = ct{467};
t1730 = ct{468};
t1731 = ct{469};
t1734 = ct{470};
t1735 = ct{471};
t1736 = ct{472};
t1737 = ct{473};
t1739 = ct{474};
t1740 = ct{475};
t1741 = ct{476};
t1742 = ct{477};
t1743 = ct{478};
t1744 = ct{479};
t1745 = ct{480};
t1746 = ct{481};
t1747 = ct{482};
t1748 = ct{483};
t1749 = ct{484};
t1750 = ct{485};
t1751 = ct{486};
t1752 = ct{487};
t1753 = ct{488};
t1755 = ct{489};
t1756 = ct{490};
t1758 = ct{491};
t1759 = ct{492};
t1761 = ct{493};
t1762 = ct{494};
t1763 = ct{495};
t1764 = ct{496};
t1765 = ct{497};
t1770 = ct{498};
t1771 = ct{499};
t1774 = ct{500};
t1777 = ct{501};
t1778 = ct{502};
t1779 = ct{503};
t1780 = ct{504};
t1781 = ct{505};
t1782 = ct{506};
t1783 = ct{507};
t1784 = ct{508};
t1785 = ct{509};
t1786 = ct{510};
t1787 = ct{511};
t1788 = ct{512};
t1789 = ct{513};
t1790 = ct{514};
t1791 = ct{515};
t1792 = ct{516};
t1798 = ct{517};
t1799 = ct{518};
t1800 = ct{519};
t1801 = ct{520};
t1802 = ct{521};
t1806 = ct{522};
t1809 = ct{523};
t1810 = ct{524};
t1813 = ct{525};
t1814 = ct{526};
t1815 = ct{527};
t1817 = ct{528};
t1820 = ct{529};
t1821 = ct{530};
t1822 = ct{531};
t1823 = ct{532};
t1824 = ct{533};
t1826 = ct{534};
t1828 = ct{535};
t1829 = ct{536};
t1830 = ct{537};
t1831 = ct{538};
t1832 = ct{539};
t1836 = ct{540};
t1839 = ct{541};
t1840 = ct{542};
t1841 = ct{543};
t1843 = ct{544};
t1844 = ct{545};
t1845 = ct{546};
t1846 = ct{547};
t1847 = ct{548};
t1849 = ct{549};
t1851 = ct{550};
t1852 = ct{551};
t1853 = ct{552};
t1855 = ct{553};
t1857 = ct{554};
t1858 = ct{555};
t1859 = ct{556};
t1860 = ct{557};
t1862 = ct{558};
t1863 = ct{559};
t1864 = ct{560};
t1865 = ct{561};
t1866 = ct{562};
t1867 = ct{563};
t1869 = ct{564};
t1870 = ct{565};
t1871 = ct{566};
t1872 = ct{567};
t1874 = ct{568};
t1875 = ct{569};
t1878 = ct{570};
t1880 = ct{571};
t1881 = ct{572};
t1882 = ct{573};
t1883 = ct{574};
t1884 = ct{575};
t1885 = ct{576};
t1887 = ct{577};
t1888 = ct{578};
t1890 = ct{579};
t1891 = ct{580};
t1893 = ct{581};
t1894 = ct{582};
t1895 = ct{583};
t1896 = ct{584};
t1898 = ct{585};
t1899 = ct{586};
t1900 = ct{587};
t1902 = ct{588};
t1904 = ct{589};
t1905 = ct{590};
t1906 = ct{591};
t1907 = ct{592};
t1908 = ct{593};
t1909 = ct{594};
t1910 = ct{595};
t1911 = ct{596};
t1912 = ct{597};
t1914 = ct{598};
t1915 = ct{599};
t1916 = ct{600};
t1917 = ct{601};
t1918 = ct{602};
t1921 = ct{603};
t1922 = ct{604};
t1924 = ct{605};
t1928 = ct{606};
t1929 = ct{607};
t1930 = ct{608};
t1931 = ct{609};
t1932 = ct{610};
t1937 = ct{611};
t1938 = ct{612};
t1939 = ct{613};
t1940 = ct{614};
t1941 = ct{615};
t1942 = ct{616};
t1943 = ct{617};
t1945 = ct{618};
t1946 = ct{619};
t1947 = ct{620};
t1948 = ct{621};
t1949 = ct{622};
t195 = ct{623};
t1950 = ct{624};
t1951 = ct{625};
t1952 = ct{626};
t1955 = ct{627};
t1956 = ct{628};
t1957 = ct{629};
t1959 = ct{630};
t1960 = ct{631};
t1961 = ct{632};
t1962 = ct{633};
t1963 = ct{634};
t1964 = ct{635};
t1965 = ct{636};
t1966 = ct{637};
t1967 = ct{638};
t1968 = ct{639};
t1969 = ct{640};
t197 = ct{641};
t1970 = ct{642};
t1971 = ct{643};
t1973 = ct{644};
t1974 = ct{645};
t1975 = ct{646};
t1976 = ct{647};
t1977 = ct{648};
t1978 = ct{649};
t1979 = ct{650};
t1980 = ct{651};
t1981 = ct{652};
t1982 = ct{653};
t1983 = ct{654};
t1985 = ct{655};
t1986 = ct{656};
t1989 = ct{657};
t1990 = ct{658};
t1991 = ct{659};
t1993 = ct{660};
t1995 = ct{661};
t1997 = ct{662};
t1998 = ct{663};
t1999 = ct{664};
t2 = ct{665};
t2000 = ct{666};
t2001 = ct{667};
t2002 = ct{668};
t2003 = ct{669};
t2004 = ct{670};
t2005 = ct{671};
t2006 = ct{672};
t2007 = ct{673};
t2008 = ct{674};
t2009 = ct{675};
t2010 = ct{676};
t2011 = ct{677};
t2012 = ct{678};
t2013 = ct{679};
t2015 = ct{680};
t2016 = ct{681};
t2017 = ct{682};
t2018 = ct{683};
t2019 = ct{684};
t2020 = ct{685};
t2023 = ct{686};
t2024 = ct{687};
t2025 = ct{688};
t2026 = ct{689};
t2032 = ct{690};
t2033 = ct{691};
t2035 = ct{692};
t2037 = ct{693};
t2038 = ct{694};
t2039 = ct{695};
t2040 = ct{696};
t2041 = ct{697};
t2042 = ct{698};
t2043 = ct{699};
t2045 = ct{700};
t2046 = ct{701};
t2047 = ct{702};
t2048 = ct{703};
t2049 = ct{704};
t2050 = ct{705};
t2053 = ct{706};
t2057 = ct{707};
t2058 = ct{708};
t2059 = ct{709};
t2061 = ct{710};
t2062 = ct{711};
t2064 = ct{712};
t2065 = ct{713};
t2066 = ct{714};
t2067 = ct{715};
t2068 = ct{716};
t2069 = ct{717};
t2070 = ct{718};
t2072 = ct{719};
t2073 = ct{720};
t2074 = ct{721};
t2075 = ct{722};
t2076 = ct{723};
t2078 = ct{724};
t2079 = ct{725};
t2080 = ct{726};
t2081 = ct{727};
t2082 = ct{728};
t2083 = ct{729};
t2084 = ct{730};
t2085 = ct{731};
t2087 = ct{732};
t2088 = ct{733};
t2090 = ct{734};
t2091 = ct{735};
t2093 = ct{736};
t2094 = ct{737};
t2095 = ct{738};
t2096 = ct{739};
t2097 = ct{740};
t2101 = ct{741};
t2102 = ct{742};
t2103 = ct{743};
t2104 = ct{744};
t2106 = ct{745};
t2107 = ct{746};
t2108 = ct{747};
t2109 = ct{748};
t2110 = ct{749};
t2111 = ct{750};
t2112 = ct{751};
t2113 = ct{752};
t2115 = ct{753};
t2117 = ct{754};
t2118 = ct{755};
t2119 = ct{756};
t2120 = ct{757};
t2122 = ct{758};
t2123 = ct{759};
t2124 = ct{760};
t2125 = ct{761};
t2127 = ct{762};
t2128 = ct{763};
t2129 = ct{764};
t2130 = ct{765};
t2131 = ct{766};
t2132 = ct{767};
t2134 = ct{768};
t2135 = ct{769};
t2137 = ct{770};
t2138 = ct{771};
t2139 = ct{772};
t214 = ct{773};
t2141 = ct{774};
t2143 = ct{775};
t2144 = ct{776};
t2147 = ct{777};
t2148 = ct{778};
t2150 = ct{779};
t2151 = ct{780};
t2152 = ct{781};
t2153 = ct{782};
t2154 = ct{783};
t2155 = ct{784};
t2156 = ct{785};
t2157 = ct{786};
t2158 = ct{787};
t2160 = ct{788};
t2161 = ct{789};
t2162 = ct{790};
t2165 = ct{791};
t2169 = ct{792};
t2170 = ct{793};
t2171 = ct{794};
t2172 = ct{795};
t2173 = ct{796};
t2174 = ct{797};
t2175 = ct{798};
t2176 = ct{799};
t2177 = ct{800};
t2178 = ct{801};
t2179 = ct{802};
t2181 = ct{803};
t2182 = ct{804};
t2183 = ct{805};
t2186 = ct{806};
t2188 = ct{807};
t2189 = ct{808};
t2190 = ct{809};
t2191 = ct{810};
t2192 = ct{811};
t2193 = ct{812};
t2194 = ct{813};
t2195 = ct{814};
t2196 = ct{815};
t2197 = ct{816};
t2198 = ct{817};
t2199 = ct{818};
t2200 = ct{819};
t2201 = ct{820};
t2202 = ct{821};
t2203 = ct{822};
t2205 = ct{823};
t2206 = ct{824};
t2208 = ct{825};
t2209 = ct{826};
t2210 = ct{827};
t2211 = ct{828};
t2212 = ct{829};
t2213 = ct{830};
t2214 = ct{831};
t2215 = ct{832};
t2216 = ct{833};
t2217 = ct{834};
t2218 = ct{835};
t2219 = ct{836};
t2220 = ct{837};
t2221 = ct{838};
t2222 = ct{839};
t2223 = ct{840};
t2224 = ct{841};
t2225 = ct{842};
t2227 = ct{843};
t2229 = ct{844};
t2230 = ct{845};
t2232 = ct{846};
t2233 = ct{847};
t2234 = ct{848};
t2235 = ct{849};
t2236 = ct{850};
t2237 = ct{851};
t2238 = ct{852};
t2240 = ct{853};
t2241 = ct{854};
t2242 = ct{855};
t2243 = ct{856};
t2244 = ct{857};
t2245 = ct{858};
t2246 = ct{859};
t2247 = ct{860};
t2248 = ct{861};
t2249 = ct{862};
t2250 = ct{863};
t2251 = ct{864};
t2252 = ct{865};
t2253 = ct{866};
t2254 = ct{867};
t2255 = ct{868};
t2257 = ct{869};
t2258 = ct{870};
t2259 = ct{871};
t2260 = ct{872};
t2262 = ct{873};
t2263 = ct{874};
t2268 = ct{875};
t2269 = ct{876};
t2270 = ct{877};
t2271 = ct{878};
t2274 = ct{879};
t2276 = ct{880};
t2277 = ct{881};
t2279 = ct{882};
t2281 = ct{883};
t2282 = ct{884};
t2284 = ct{885};
t2285 = ct{886};
t2286 = ct{887};
t2287 = ct{888};
t2288 = ct{889};
t2289 = ct{890};
t2290 = ct{891};
t2293 = ct{892};
t2294 = ct{893};
t2296 = ct{894};
t2298 = ct{895};
t2299 = ct{896};
t2303 = ct{897};
t2304 = ct{898};
t2305 = ct{899};
t2307 = ct{900};
t2308 = ct{901};
t2312 = ct{902};
t2313 = ct{903};
t2316 = ct{904};
t2317 = ct{905};
t2318 = ct{906};
t2319 = ct{907};
t2320 = ct{908};
t2321 = ct{909};
t2322 = ct{910};
t2323 = ct{911};
t2324 = ct{912};
t2325 = ct{913};
t2329 = ct{914};
t2330 = ct{915};
t2332 = ct{916};
t2333 = ct{917};
t2334 = ct{918};
t2335 = ct{919};
t2336 = ct{920};
t2338 = ct{921};
t2339 = ct{922};
t2340 = ct{923};
t2341 = ct{924};
t2342 = ct{925};
t2343 = ct{926};
t2345 = ct{927};
t2346 = ct{928};
t2347 = ct{929};
t2348 = ct{930};
t2349 = ct{931};
t2350 = ct{932};
t2351 = ct{933};
t2352 = ct{934};
t2354 = ct{935};
t2355 = ct{936};
t2356 = ct{937};
t2358 = ct{938};
t2360 = ct{939};
t2361 = ct{940};
t2362 = ct{941};
t2363 = ct{942};
t2364 = ct{943};
t2368 = ct{944};
t2369 = ct{945};
t2370 = ct{946};
t2371 = ct{947};
t2376 = ct{948};
t2380 = ct{949};
t2381 = ct{950};
t2382 = ct{951};
t2385 = ct{952};
t2386 = ct{953};
t2387 = ct{954};
t2388 = ct{955};
t2389 = ct{956};
t2390 = ct{957};
t2391 = ct{958};
t2392 = ct{959};
t2397 = ct{960};
t2399 = ct{961};
t24 = ct{962};
t2400 = ct{963};
t2401 = ct{964};
t2403 = ct{965};
t2404 = ct{966};
t2406 = ct{967};
t2407 = ct{968};
t2408 = ct{969};
t2409 = ct{970};
t2410 = ct{971};
t2411 = ct{972};
t2412 = ct{973};
t2413 = ct{974};
t2416 = ct{975};
t2417 = ct{976};
t2419 = ct{977};
t2420 = ct{978};
t2422 = ct{979};
t2423 = ct{980};
t2425 = ct{981};
t2426 = ct{982};
t2427 = ct{983};
t2428 = ct{984};
t2429 = ct{985};
t2430 = ct{986};
t2431 = ct{987};
t2433 = ct{988};
t2434 = ct{989};
t2435 = ct{990};
t2436 = ct{991};
t2437 = ct{992};
t2438 = ct{993};
t2439 = ct{994};
t2445 = ct{995};
t2447 = ct{996};
t2448 = ct{997};
t2449 = ct{998};
t2450 = ct{999};
t2451 = ct{1000};
t2453 = ct{1001};
t2454 = ct{1002};
t2455 = ct{1003};
t2457 = ct{1004};
t2458 = ct{1005};
t2459 = ct{1006};
t2460 = ct{1007};
t2461 = ct{1008};
t2462 = ct{1009};
t2463 = ct{1010};
t2464 = ct{1011};
t2465 = ct{1012};
t2467 = ct{1013};
t2468 = ct{1014};
t2469 = ct{1015};
t2470 = ct{1016};
t2471 = ct{1017};
t2472 = ct{1018};
t2474 = ct{1019};
t2476 = ct{1020};
t2479 = ct{1021};
t2480 = ct{1022};
t2483 = ct{1023};
t2484 = ct{1024};
t2485 = ct{1025};
t2486 = ct{1026};
t2487 = ct{1027};
t2488 = ct{1028};
t2489 = ct{1029};
t2492 = ct{1030};
t2495 = ct{1031};
t2496 = ct{1032};
t2498 = ct{1033};
t25 = ct{1034};
t2501 = ct{1035};
t2502 = ct{1036};
t2503 = ct{1037};
t2504 = ct{1038};
t2505 = ct{1039};
t2506 = ct{1040};
t2511 = ct{1041};
t2512 = ct{1042};
t2513 = ct{1043};
t2514 = ct{1044};
t2515 = ct{1045};
t2516 = ct{1046};
t2518 = ct{1047};
t2519 = ct{1048};
t2521 = ct{1049};
t2522 = ct{1050};
t2523 = ct{1051};
t2524 = ct{1052};
t2525 = ct{1053};
t2526 = ct{1054};
t2527 = ct{1055};
t2528 = ct{1056};
t2529 = ct{1057};
t2530 = ct{1058};
t2531 = ct{1059};
t2532 = ct{1060};
t2533 = ct{1061};
t2534 = ct{1062};
t2535 = ct{1063};
t2536 = ct{1064};
t2537 = ct{1065};
t2538 = ct{1066};
t2539 = ct{1067};
t2541 = ct{1068};
t2542 = ct{1069};
t2543 = ct{1070};
t2544 = ct{1071};
t2545 = ct{1072};
t2546 = ct{1073};
t2547 = ct{1074};
t2548 = ct{1075};
t2549 = ct{1076};
t2550 = ct{1077};
t2551 = ct{1078};
t2552 = ct{1079};
t2554 = ct{1080};
t2555 = ct{1081};
t2558 = ct{1082};
t2559 = ct{1083};
t2560 = ct{1084};
t2561 = ct{1085};
t2562 = ct{1086};
t2563 = ct{1087};
t2564 = ct{1088};
t2565 = ct{1089};
t2566 = ct{1090};
t2567 = ct{1091};
t2568 = ct{1092};
t2569 = ct{1093};
t2570 = ct{1094};
t2571 = ct{1095};
t2573 = ct{1096};
t2574 = ct{1097};
t2575 = ct{1098};
t2576 = ct{1099};
t2577 = ct{1100};
t2578 = ct{1101};
t2579 = ct{1102};
t2581 = ct{1103};
t2582 = ct{1104};
t2583 = ct{1105};
t2584 = ct{1106};
t2585 = ct{1107};
t2587 = ct{1108};
t2588 = ct{1109};
t2589 = ct{1110};
t259 = ct{1111};
t2590 = ct{1112};
t2591 = ct{1113};
t2595 = ct{1114};
t2597 = ct{1115};
t2598 = ct{1116};
t2599 = ct{1117};
t26 = ct{1118};
t260 = ct{1119};
t2600 = ct{1120};
t2601 = ct{1121};
t2602 = ct{1122};
t2605 = ct{1123};
t2606 = ct{1124};
t2607 = ct{1125};
t2609 = ct{1126};
t2610 = ct{1127};
t2611 = ct{1128};
t2613 = ct{1129};
t2615 = ct{1130};
t2616 = ct{1131};
t2617 = ct{1132};
t2619 = ct{1133};
t2620 = ct{1134};
t2621 = ct{1135};
t2623 = ct{1136};
t2624 = ct{1137};
t2627 = ct{1138};
t2629 = ct{1139};
t2630 = ct{1140};
t2632 = ct{1141};
t2634 = ct{1142};
t2635 = ct{1143};
t2636 = ct{1144};
t2637 = ct{1145};
t2638 = ct{1146};
t2639 = ct{1147};
t2640 = ct{1148};
t2641 = ct{1149};
t2644 = ct{1150};
t2645 = ct{1151};
t2646 = ct{1152};
t2647 = ct{1153};
t2648 = ct{1154};
t2649 = ct{1155};
t2650 = ct{1156};
t2651 = ct{1157};
t2652 = ct{1158};
t2654 = ct{1159};
t2656 = ct{1160};
t2657 = ct{1161};
t2658 = ct{1162};
t2660 = ct{1163};
t2661 = ct{1164};
t2662 = ct{1165};
t2663 = ct{1166};
t2665 = ct{1167};
t2666 = ct{1168};
t2667 = ct{1169};
t2668 = ct{1170};
t2669 = ct{1171};
t2671 = ct{1172};
t2672 = ct{1173};
t2673 = ct{1174};
t2674 = ct{1175};
t2675 = ct{1176};
t2676 = ct{1177};
t2677 = ct{1178};
t2678 = ct{1179};
t2679 = ct{1180};
t2682 = ct{1181};
t2684 = ct{1182};
t2685 = ct{1183};
t2688 = ct{1184};
t2689 = ct{1185};
t2691 = ct{1186};
t2692 = ct{1187};
t2696 = ct{1188};
t2698 = ct{1189};
t2699 = ct{1190};
t27 = ct{1191};
t2700 = ct{1192};
t2705 = ct{1193};
t2706 = ct{1194};
t2707 = ct{1195};
t2708 = ct{1196};
t2710 = ct{1197};
t2712 = ct{1198};
t2714 = ct{1199};
t2715 = ct{1200};
t2717 = ct{1201};
t2718 = ct{1202};
t2722 = ct{1203};
t2723 = ct{1204};
t2725 = ct{1205};
t2726 = ct{1206};
t2727 = ct{1207};
t2728 = ct{1208};
t2730 = ct{1209};
t2731 = ct{1210};
t2732 = ct{1211};
t2733 = ct{1212};
t2734 = ct{1213};
t2735 = ct{1214};
t2736 = ct{1215};
t2737 = ct{1216};
t2738 = ct{1217};
t2740 = ct{1218};
t2741 = ct{1219};
t2742 = ct{1220};
t2743 = ct{1221};
t2744 = ct{1222};
t2746 = ct{1223};
t2748 = ct{1224};
t2749 = ct{1225};
t2750 = ct{1226};
t2751 = ct{1227};
t2752 = ct{1228};
t2754 = ct{1229};
t2755 = ct{1230};
t2756 = ct{1231};
t2758 = ct{1232};
t2759 = ct{1233};
t276 = ct{1234};
t2760 = ct{1235};
t2761 = ct{1236};
t2763 = ct{1237};
t2764 = ct{1238};
t2765 = ct{1239};
t2766 = ct{1240};
t2767 = ct{1241};
t2768 = ct{1242};
t2769 = ct{1243};
t277 = ct{1244};
t2771 = ct{1245};
t2772 = ct{1246};
t2774 = ct{1247};
t2775 = ct{1248};
t2776 = ct{1249};
t2778 = ct{1250};
t2779 = ct{1251};
t2780 = ct{1252};
t2781 = ct{1253};
t2782 = ct{1254};
t2783 = ct{1255};
t2785 = ct{1256};
t2786 = ct{1257};
t2787 = ct{1258};
t2788 = ct{1259};
t2790 = ct{1260};
t2791 = ct{1261};
t2792 = ct{1262};
t2793 = ct{1263};
t2794 = ct{1264};
t2796 = ct{1265};
t2797 = ct{1266};
t2798 = ct{1267};
t2799 = ct{1268};
t2800 = ct{1269};
t2802 = ct{1270};
t2803 = ct{1271};
t2804 = ct{1272};
t2805 = ct{1273};
t2806 = ct{1274};
t2807 = ct{1275};
t2811 = ct{1276};
t2813 = ct{1277};
t2814 = ct{1278};
t2816 = ct{1279};
t2817 = ct{1280};
t2818 = ct{1281};
t2819 = ct{1282};
t2821 = ct{1283};
t2823 = ct{1284};
t2824 = ct{1285};
t2825 = ct{1286};
t2828 = ct{1287};
t2829 = ct{1288};
t283 = ct{1289};
t2830 = ct{1290};
t2831 = ct{1291};
t2832 = ct{1292};
t2833 = ct{1293};
t2834 = ct{1294};
t2835 = ct{1295};
t2836 = ct{1296};
t2837 = ct{1297};
t2838 = ct{1298};
t2839 = ct{1299};
t284 = ct{1300};
t2841 = ct{1301};
t2842 = ct{1302};
t2843 = ct{1303};
t2844 = ct{1304};
t2845 = ct{1305};
t2846 = ct{1306};
t2847 = ct{1307};
t2848 = ct{1308};
t2849 = ct{1309};
t285 = ct{1310};
t2852 = ct{1311};
t2853 = ct{1312};
t2857 = ct{1313};
t2858 = ct{1314};
t2859 = ct{1315};
t286 = ct{1316};
t2860 = ct{1317};
t2861 = ct{1318};
t2864 = ct{1319};
t2865 = ct{1320};
t2866 = ct{1321};
t2867 = ct{1322};
t2868 = ct{1323};
t287 = ct{1324};
t2870 = ct{1325};
t2871 = ct{1326};
t2872 = ct{1327};
t2874 = ct{1328};
t2875 = ct{1329};
t2876 = ct{1330};
t2877 = ct{1331};
t2878 = ct{1332};
t2879 = ct{1333};
t288 = ct{1334};
t2880 = ct{1335};
t2882 = ct{1336};
t2883 = ct{1337};
t2884 = ct{1338};
t2886 = ct{1339};
t2887 = ct{1340};
t2889 = ct{1341};
t289 = ct{1342};
t2890 = ct{1343};
t2892 = ct{1344};
t2893 = ct{1345};
t2895 = ct{1346};
t2896 = ct{1347};
t2897 = ct{1348};
t2898 = ct{1349};
t2899 = ct{1350};
t290 = ct{1351};
t2901 = ct{1352};
t2902 = ct{1353};
t2903 = ct{1354};
t2904 = ct{1355};
t2905 = ct{1356};
t2906 = ct{1357};
t2907 = ct{1358};
t2909 = ct{1359};
t291 = ct{1360};
t2912 = ct{1361};
t2913 = ct{1362};
t2914 = ct{1363};
t2915 = ct{1364};
t2916 = ct{1365};
t2917 = ct{1366};
t2918 = ct{1367};
t2919 = ct{1368};
t292 = ct{1369};
t2920 = ct{1370};
t2921 = ct{1371};
t2922 = ct{1372};
t2924 = ct{1373};
t2926 = ct{1374};
t2927 = ct{1375};
t2928 = ct{1376};
t2929 = ct{1377};
t293 = ct{1378};
t2930 = ct{1379};
t2932 = ct{1380};
t2934 = ct{1381};
t2935 = ct{1382};
t2936 = ct{1383};
t2937 = ct{1384};
t2938 = ct{1385};
t2939 = ct{1386};
t294 = ct{1387};
t2940 = ct{1388};
t2941 = ct{1389};
t2942 = ct{1390};
t2943 = ct{1391};
t2944 = ct{1392};
t2945 = ct{1393};
t2946 = ct{1394};
t2949 = ct{1395};
t2950 = ct{1396};
t2952 = ct{1397};
t2954 = ct{1398};
t2955 = ct{1399};
t2956 = ct{1400};
t2957 = ct{1401};
t2959 = ct{1402};
t2960 = ct{1403};
t2961 = ct{1404};
t2962 = ct{1405};
t2963 = ct{1406};
t2964 = ct{1407};
t2965 = ct{1408};
t2966 = ct{1409};
t2967 = ct{1410};
t2969 = ct{1411};
t2970 = ct{1412};
t2971 = ct{1413};
t2972 = ct{1414};
t2975 = ct{1415};
t2976 = ct{1416};
t2977 = ct{1417};
t2978 = ct{1418};
t2979 = ct{1419};
t2981 = ct{1420};
t2982 = ct{1421};
t2985 = ct{1422};
t2986 = ct{1423};
t2987 = ct{1424};
t2988 = ct{1425};
t2989 = ct{1426};
t2992 = ct{1427};
t2994 = ct{1428};
t2995 = ct{1429};
t2996 = ct{1430};
t2997 = ct{1431};
t2998 = ct{1432};
t2999 = ct{1433};
t3 = ct{1434};
t30 = ct{1435};
t3000 = ct{1436};
t3003 = ct{1437};
t3004 = ct{1438};
t3006 = ct{1439};
t3007 = ct{1440};
t3008 = ct{1441};
t3009 = ct{1442};
t3010 = ct{1443};
t3011 = ct{1444};
t3012 = ct{1445};
t3016 = ct{1446};
t3017 = ct{1447};
t3019 = ct{1448};
t3022 = ct{1449};
t3027 = ct{1450};
t3030 = ct{1451};
t3031 = ct{1452};
t3032 = ct{1453};
t3033 = ct{1454};
t3034 = ct{1455};
t3035 = ct{1456};
t3037 = ct{1457};
t3038 = ct{1458};
t3039 = ct{1459};
t304 = ct{1460};
t3041 = ct{1461};
t3042 = ct{1462};
t3043 = ct{1463};
t3047 = ct{1464};
t3049 = ct{1465};
t3050 = ct{1466};
t3051 = ct{1467};
t3054 = ct{1468};
t3059 = ct{1469};
t3060 = ct{1470};
t3061 = ct{1471};
t3062 = ct{1472};
t3063 = ct{1473};
t3064 = ct{1474};
t3065 = ct{1475};
t3066 = ct{1476};
t3069 = ct{1477};
t3070 = ct{1478};
t3072 = ct{1479};
t3074 = ct{1480};
t3075 = ct{1481};
t3076 = ct{1482};
t3077 = ct{1483};
t3078 = ct{1484};
t3080 = ct{1485};
t3082 = ct{1486};
t3083 = ct{1487};
t3084 = ct{1488};
t3085 = ct{1489};
t3086 = ct{1490};
t3087 = ct{1491};
t3089 = ct{1492};
t3090 = ct{1493};
t3091 = ct{1494};
t3092 = ct{1495};
t3093 = ct{1496};
t3094 = ct{1497};
t3096 = ct{1498};
t3097 = ct{1499};
t3098 = ct{1500};
t3099 = ct{1501};
t3100 = ct{1502};
t3102 = ct{1503};
t3103 = ct{1504};
t3104 = ct{1505};
t3105 = ct{1506};
t3106 = ct{1507};
t3107 = ct{1508};
t3108 = ct{1509};
t3109 = ct{1510};
t3110 = ct{1511};
t3112 = ct{1512};
t3113 = ct{1513};
t3114 = ct{1514};
t3115 = ct{1515};
t3117 = ct{1516};
t3119 = ct{1517};
t3121 = ct{1518};
t3122 = ct{1519};
t3123 = ct{1520};
t3124 = ct{1521};
t3127 = ct{1522};
t3128 = ct{1523};
t3130 = ct{1524};
t3131 = ct{1525};
t3132 = ct{1526};
t3133 = ct{1527};
t3134 = ct{1528};
t3135 = ct{1529};
t3136 = ct{1530};
t3138 = ct{1531};
t3139 = ct{1532};
t3145 = ct{1533};
t3146 = ct{1534};
t3147 = ct{1535};
t3149 = ct{1536};
t3151 = ct{1537};
t3153 = ct{1538};
t3155 = ct{1539};
t3156 = ct{1540};
t3157 = ct{1541};
t3158 = ct{1542};
t3160 = ct{1543};
t3161 = ct{1544};
t3162 = ct{1545};
t3163 = ct{1546};
t3164 = ct{1547};
t3165 = ct{1548};
t3166 = ct{1549};
t3167 = ct{1550};
t3168 = ct{1551};
t3169 = ct{1552};
t3170 = ct{1553};
t3171 = ct{1554};
t3173 = ct{1555};
t3174 = ct{1556};
t3175 = ct{1557};
t3176 = ct{1558};
t3177 = ct{1559};
t3178 = ct{1560};
t3179 = ct{1561};
t3180 = ct{1562};
t3181 = ct{1563};
t3183 = ct{1564};
t3184 = ct{1565};
t3185 = ct{1566};
t3186 = ct{1567};
t3187 = ct{1568};
t3189 = ct{1569};
t3192 = ct{1570};
t3195 = ct{1571};
t3196 = ct{1572};
t3197 = ct{1573};
t3198 = ct{1574};
t3199 = ct{1575};
t3200 = ct{1576};
t3203 = ct{1577};
t3204 = ct{1578};
t3206 = ct{1579};
t3207 = ct{1580};
t3210 = ct{1581};
t3212 = ct{1582};
t3213 = ct{1583};
t3214 = ct{1584};
t3215 = ct{1585};
t3216 = ct{1586};
t3217 = ct{1587};
t3218 = ct{1588};
t3219 = ct{1589};
t3220 = ct{1590};
t3221 = ct{1591};
t3222 = ct{1592};
t3223 = ct{1593};
t3224 = ct{1594};
t3226 = ct{1595};
t3227 = ct{1596};
t3230 = ct{1597};
t3231 = ct{1598};
t3232 = ct{1599};
t3233 = ct{1600};
t3234 = ct{1601};
t3235 = ct{1602};
t3236 = ct{1603};
t3238 = ct{1604};
t3239 = ct{1605};
t3240 = ct{1606};
t3241 = ct{1607};
t3243 = ct{1608};
t3244 = ct{1609};
t3245 = ct{1610};
t3247 = ct{1611};
t3248 = ct{1612};
t3250 = ct{1613};
t3251 = ct{1614};
t3252 = ct{1615};
t3254 = ct{1616};
t3256 = ct{1617};
t3258 = ct{1618};
t3260 = ct{1619};
t3261 = ct{1620};
t3262 = ct{1621};
t3263 = ct{1622};
t3265 = ct{1623};
t3266 = ct{1624};
t3267 = ct{1625};
t3270 = ct{1626};
t3271 = ct{1627};
t3272 = ct{1628};
t3273 = ct{1629};
t3276 = ct{1630};
t3277 = ct{1631};
t3278 = ct{1632};
t3279 = ct{1633};
t3280 = ct{1634};
t3281 = ct{1635};
t3282 = ct{1636};
t3284 = ct{1637};
t3285 = ct{1638};
t3286 = ct{1639};
t3287 = ct{1640};
t3288 = ct{1641};
t3289 = ct{1642};
t3290 = ct{1643};
t3291 = ct{1644};
t3292 = ct{1645};
t3293 = ct{1646};
t3296 = ct{1647};
t3299 = ct{1648};
t33 = ct{1649};
t3300 = ct{1650};
t3301 = ct{1651};
t3302 = ct{1652};
t3303 = ct{1653};
t3304 = ct{1654};
t3305 = ct{1655};
t3306 = ct{1656};
t3307 = ct{1657};
t3308 = ct{1658};
t3311 = ct{1659};
t3312 = ct{1660};
t3313 = ct{1661};
t3314 = ct{1662};
t3315 = ct{1663};
t3316 = ct{1664};
t3317 = ct{1665};
t3319 = ct{1666};
t3320 = ct{1667};
t3321 = ct{1668};
t3322 = ct{1669};
t3323 = ct{1670};
t3324 = ct{1671};
t3325 = ct{1672};
t3326 = ct{1673};
t3327 = ct{1674};
t3330 = ct{1675};
t3331 = ct{1676};
t3332 = ct{1677};
t3333 = ct{1678};
t3334 = ct{1679};
t3337 = ct{1680};
t3338 = ct{1681};
t3339 = ct{1682};
t3340 = ct{1683};
t3341 = ct{1684};
t3342 = ct{1685};
t3343 = ct{1686};
t3347 = ct{1687};
t3348 = ct{1688};
t3349 = ct{1689};
t3351 = ct{1690};
t3352 = ct{1691};
t3353 = ct{1692};
t3354 = ct{1693};
t3355 = ct{1694};
t3356 = ct{1695};
t3357 = ct{1696};
t3359 = ct{1697};
t3360 = ct{1698};
t3361 = ct{1699};
t3365 = ct{1700};
t3366 = ct{1701};
t3367 = ct{1702};
t3368 = ct{1703};
t3370 = ct{1704};
t3372 = ct{1705};
t3373 = ct{1706};
t3375 = ct{1707};
t3376 = ct{1708};
t3377 = ct{1709};
t3378 = ct{1710};
t3379 = ct{1711};
t3380 = ct{1712};
t3381 = ct{1713};
t3382 = ct{1714};
t3384 = ct{1715};
t3385 = ct{1716};
t3386 = ct{1717};
t3387 = ct{1718};
t3388 = ct{1719};
t3390 = ct{1720};
t3391 = ct{1721};
t3392 = ct{1722};
t3393 = ct{1723};
t3396 = ct{1724};
t3397 = ct{1725};
t3398 = ct{1726};
t3399 = ct{1727};
t34 = ct{1728};
t3400 = ct{1729};
t3401 = ct{1730};
t3403 = ct{1731};
t3404 = ct{1732};
t3405 = ct{1733};
t3406 = ct{1734};
t3407 = ct{1735};
t3408 = ct{1736};
t3409 = ct{1737};
t3410 = ct{1738};
t3412 = ct{1739};
t3413 = ct{1740};
t3414 = ct{1741};
t3415 = ct{1742};
t3416 = ct{1743};
t3419 = ct{1744};
t3420 = ct{1745};
t3421 = ct{1746};
t3423 = ct{1747};
t3424 = ct{1748};
t3425 = ct{1749};
t3426 = ct{1750};
t3427 = ct{1751};
t3429 = ct{1752};
t3430 = ct{1753};
t3431 = ct{1754};
t3432 = ct{1755};
t3433 = ct{1756};
t3434 = ct{1757};
t3437 = ct{1758};
t3438 = ct{1759};
t3439 = ct{1760};
t3440 = ct{1761};
t3441 = ct{1762};
t3442 = ct{1763};
t3443 = ct{1764};
t3444 = ct{1765};
t3445 = ct{1766};
t3446 = ct{1767};
t3447 = ct{1768};
t3448 = ct{1769};
t3449 = ct{1770};
t3450 = ct{1771};
t3452 = ct{1772};
t3453 = ct{1773};
t3454 = ct{1774};
t3455 = ct{1775};
t3456 = ct{1776};
t3457 = ct{1777};
t3458 = ct{1778};
t3459 = ct{1779};
t3460 = ct{1780};
t3462 = ct{1781};
t3463 = ct{1782};
t3464 = ct{1783};
t3465 = ct{1784};
t3466 = ct{1785};
t3467 = ct{1786};
t3468 = ct{1787};
t3469 = ct{1788};
t3470 = ct{1789};
t3471 = ct{1790};
t3472 = ct{1791};
t3474 = ct{1792};
t3475 = ct{1793};
t3476 = ct{1794};
t3477 = ct{1795};
t3478 = ct{1796};
t3479 = ct{1797};
t3480 = ct{1798};
t3481 = ct{1799};
t3483 = ct{1800};
t3484 = ct{1801};
t3485 = ct{1802};
t3486 = ct{1803};
t3487 = ct{1804};
t3488 = ct{1805};
t3489 = ct{1806};
t3490 = ct{1807};
t3491 = ct{1808};
t3492 = ct{1809};
t3494 = ct{1810};
t3495 = ct{1811};
t3496 = ct{1812};
t3497 = ct{1813};
t3499 = ct{1814};
t3500 = ct{1815};
t3501 = ct{1816};
t3502 = ct{1817};
t3504 = ct{1818};
t3506 = ct{1819};
t3508 = ct{1820};
t3509 = ct{1821};
t3510 = ct{1822};
t3511 = ct{1823};
t3512 = ct{1824};
t3513 = ct{1825};
t3515 = ct{1826};
t3516 = ct{1827};
t3517 = ct{1828};
t3518 = ct{1829};
t3521 = ct{1830};
t3522 = ct{1831};
t3523 = ct{1832};
t3524 = ct{1833};
t3526 = ct{1834};
t3528 = ct{1835};
t3529 = ct{1836};
t3530 = ct{1837};
t3531 = ct{1838};
t3532 = ct{1839};
t3533 = ct{1840};
t3534 = ct{1841};
t3535 = ct{1842};
t3536 = ct{1843};
t3537 = ct{1844};
t3538 = ct{1845};
t3539 = ct{1846};
t3541 = ct{1847};
t3542 = ct{1848};
t3543 = ct{1849};
t3544 = ct{1850};
t3545 = ct{1851};
t3547 = ct{1852};
t3548 = ct{1853};
t3550 = ct{1854};
t3551 = ct{1855};
t3552 = ct{1856};
t3553 = ct{1857};
t3554 = ct{1858};
t3556 = ct{1859};
t3557 = ct{1860};
t3558 = ct{1861};
t3559 = ct{1862};
t3562 = ct{1863};
t3563 = ct{1864};
t3564 = ct{1865};
t3565 = ct{1866};
t3569 = ct{1867};
t3570 = ct{1868};
t3571 = ct{1869};
t3575 = ct{1870};
t3576 = ct{1871};
t3578 = ct{1872};
t3579 = ct{1873};
t3581 = ct{1874};
t3582 = ct{1875};
t3583 = ct{1876};
t3584 = ct{1877};
t3587 = ct{1878};
t3588 = ct{1879};
t3591 = ct{1880};
t3593 = ct{1881};
t3594 = ct{1882};
t3595 = ct{1883};
t3596 = ct{1884};
t3597 = ct{1885};
t3598 = ct{1886};
t3599 = ct{1887};
t3600 = ct{1888};
t3601 = ct{1889};
t3602 = ct{1890};
t3603 = ct{1891};
t3604 = ct{1892};
t3605 = ct{1893};
t3606 = ct{1894};
t3607 = ct{1895};
t3608 = ct{1896};
t3609 = ct{1897};
t3610 = ct{1898};
t3611 = ct{1899};
t3613 = ct{1900};
t3614 = ct{1901};
t3615 = ct{1902};
t3616 = ct{1903};
t3617 = ct{1904};
t3618 = ct{1905};
t3619 = ct{1906};
t3620 = ct{1907};
t3621 = ct{1908};
t3622 = ct{1909};
t3623 = ct{1910};
t3624 = ct{1911};
t3625 = ct{1912};
t3626 = ct{1913};
t3627 = ct{1914};
t3629 = ct{1915};
t3630 = ct{1916};
t3631 = ct{1917};
t3632 = ct{1918};
t3634 = ct{1919};
t3635 = ct{1920};
t3636 = ct{1921};
t3637 = ct{1922};
t3638 = ct{1923};
t3639 = ct{1924};
t3640 = ct{1925};
t3641 = ct{1926};
t3643 = ct{1927};
t3644 = ct{1928};
t3645 = ct{1929};
t3646 = ct{1930};
t3647 = ct{1931};
t3648 = ct{1932};
t3649 = ct{1933};
t3651 = ct{1934};
t3652 = ct{1935};
t3653 = ct{1936};
t3654 = ct{1937};
t3655 = ct{1938};
t3656 = ct{1939};
t3657 = ct{1940};
t3658 = ct{1941};
t3659 = ct{1942};
t3660 = ct{1943};
t3661 = ct{1944};
t3664 = ct{1945};
t3665 = ct{1946};
t3666 = ct{1947};
t3667 = ct{1948};
t3668 = ct{1949};
t3669 = ct{1950};
t3671 = ct{1951};
t3672 = ct{1952};
t3673 = ct{1953};
t3674 = ct{1954};
t3675 = ct{1955};
t3676 = ct{1956};
t3677 = ct{1957};
t3678 = ct{1958};
t3679 = ct{1959};
t3680 = ct{1960};
t3681 = ct{1961};
t3682 = ct{1962};
t3683 = ct{1963};
t3684 = ct{1964};
t3685 = ct{1965};
t3686 = ct{1966};
t3687 = ct{1967};
t3688 = ct{1968};
t3689 = ct{1969};
t3691 = ct{1970};
t3692 = ct{1971};
t3693 = ct{1972};
t3695 = ct{1973};
t3697 = ct{1974};
t3698 = ct{1975};
t3699 = ct{1976};
t3700 = ct{1977};
t3701 = ct{1978};
t3702 = ct{1979};
t3704 = ct{1980};
t3708 = ct{1981};
t3709 = ct{1982};
t3710 = ct{1983};
t3711 = ct{1984};
t3712 = ct{1985};
t3713 = ct{1986};
t3716 = ct{1987};
t3717 = ct{1988};
t3719 = ct{1989};
t3720 = ct{1990};
t3721 = ct{1991};
t3722 = ct{1992};
t3723 = ct{1993};
t3724 = ct{1994};
t3725 = ct{1995};
t3726 = ct{1996};
t3729 = ct{1997};
t3730 = ct{1998};
t3732 = ct{1999};
t3733 = ct{2000};
t3735 = ct{2001};
t3736 = ct{2002};
t3737 = ct{2003};
t3739 = ct{2004};
t3741 = ct{2005};
t3742 = ct{2006};
t3744 = ct{2007};
t3745 = ct{2008};
t3746 = ct{2009};
t3747 = ct{2010};
t3749 = ct{2011};
t3750 = ct{2012};
t3751 = ct{2013};
t3752 = ct{2014};
t3753 = ct{2015};
t3754 = ct{2016};
t3756 = ct{2017};
t3757 = ct{2018};
t3759 = ct{2019};
t376 = ct{2020};
t3760 = ct{2021};
t3761 = ct{2022};
t3762 = ct{2023};
t3763 = ct{2024};
t3764 = ct{2025};
t3765 = ct{2026};
t3767 = ct{2027};
t3768 = ct{2028};
t3769 = ct{2029};
t377 = ct{2030};
t3770 = ct{2031};
t3771 = ct{2032};
t3772 = ct{2033};
t3773 = ct{2034};
t3774 = ct{2035};
t3775 = ct{2036};
t3776 = ct{2037};
t3777 = ct{2038};
t3778 = ct{2039};
t3779 = ct{2040};
t3780 = ct{2041};
t3783 = ct{2042};
t3784 = ct{2043};
t3785 = ct{2044};
t3786 = ct{2045};
t3787 = ct{2046};
t3789 = ct{2047};
t3790 = ct{2048};
t3791 = ct{2049};
t3792 = ct{2050};
t3793 = ct{2051};
t3794 = ct{2052};
t3795 = ct{2053};
t3796 = ct{2054};
t3799 = ct{2055};
t38 = ct{2056};
t3802 = ct{2057};
t3803 = ct{2058};
t3804 = ct{2059};
t3805 = ct{2060};
t3806 = ct{2061};
t3807 = ct{2062};
t3808 = ct{2063};
t3809 = ct{2064};
t381 = ct{2065};
t3810 = ct{2066};
t3811 = ct{2067};
t3812 = ct{2068};
t3813 = ct{2069};
t3814 = ct{2070};
t3815 = ct{2071};
t3817 = ct{2072};
t3818 = ct{2073};
t3819 = ct{2074};
t382 = ct{2075};
t3820 = ct{2076};
t3823 = ct{2077};
t3826 = ct{2078};
t3828 = ct{2079};
t3829 = ct{2080};
t383 = ct{2081};
t3831 = ct{2082};
t3832 = ct{2083};
t3833 = ct{2084};
t3834 = ct{2085};
t3836 = ct{2086};
t3837 = ct{2087};
t3838 = ct{2088};
t3840 = ct{2089};
t3841 = ct{2090};
t3842 = ct{2091};
t3843 = ct{2092};
t3844 = ct{2093};
t3845 = ct{2094};
t3846 = ct{2095};
t3847 = ct{2096};
t3848 = ct{2097};
t3849 = ct{2098};
t3850 = ct{2099};
t3851 = ct{2100};
t3854 = ct{2101};
t3855 = ct{2102};
t3856 = ct{2103};
t3857 = ct{2104};
t3858 = ct{2105};
t3859 = ct{2106};
t3862 = ct{2107};
t3864 = ct{2108};
t3865 = ct{2109};
t3866 = ct{2110};
t3867 = ct{2111};
t3868 = ct{2112};
t3870 = ct{2113};
t3871 = ct{2114};
t3872 = ct{2115};
t3873 = ct{2116};
t3879 = ct{2117};
t3880 = ct{2118};
t3882 = ct{2119};
t3883 = ct{2120};
t3884 = ct{2121};
t3886 = ct{2122};
t3887 = ct{2123};
t3888 = ct{2124};
t3889 = ct{2125};
t3890 = ct{2126};
t3894 = ct{2127};
t3896 = ct{2128};
t3897 = ct{2129};
t3898 = ct{2130};
t3899 = ct{2131};
t390 = ct{2132};
t3900 = ct{2133};
t3901 = ct{2134};
t3902 = ct{2135};
t3903 = ct{2136};
t3906 = ct{2137};
t3907 = ct{2138};
t3908 = ct{2139};
t3909 = ct{2140};
t3910 = ct{2141};
t3911 = ct{2142};
t3913 = ct{2143};
t3914 = ct{2144};
t3915 = ct{2145};
t3916 = ct{2146};
t3918 = ct{2147};
t3919 = ct{2148};
t3921 = ct{2149};
t3922 = ct{2150};
t3923 = ct{2151};
t3926 = ct{2152};
t3928 = ct{2153};
t3929 = ct{2154};
t3930 = ct{2155};
t3931 = ct{2156};
t3932 = ct{2157};
t3933 = ct{2158};
t3934 = ct{2159};
t3935 = ct{2160};
t3936 = ct{2161};
t3937 = ct{2162};
t3938 = ct{2163};
t3939 = ct{2164};
t394 = ct{2165};
t3940 = ct{2166};
t3941 = ct{2167};
t3942 = ct{2168};
t3944 = ct{2169};
t3946 = ct{2170};
t3947 = ct{2171};
t3948 = ct{2172};
t3949 = ct{2173};
t3950 = ct{2174};
t3951 = ct{2175};
t3952 = ct{2176};
t3953 = ct{2177};
t3954 = ct{2178};
t3955 = ct{2179};
t3956 = ct{2180};
t3957 = ct{2181};
t3958 = ct{2182};
t3959 = ct{2183};
t3960 = ct{2184};
t3961 = ct{2185};
t3962 = ct{2186};
t3964 = ct{2187};
t3965 = ct{2188};
t3966 = ct{2189};
t3967 = ct{2190};
t3969 = ct{2191};
t3970 = ct{2192};
t3971 = ct{2193};
t3974 = ct{2194};
t3975 = ct{2195};
t3976 = ct{2196};
t3978 = ct{2197};
t3979 = ct{2198};
t3980 = ct{2199};
t3981 = ct{2200};
t3982 = ct{2201};
t3983 = ct{2202};
t3984 = ct{2203};
t3985 = ct{2204};
t3986 = ct{2205};
t3987 = ct{2206};
t3991 = ct{2207};
t3992 = ct{2208};
t3993 = ct{2209};
t3994 = ct{2210};
t3995 = ct{2211};
t3996 = ct{2212};
t3997 = ct{2213};
t3998 = ct{2214};
t4 = ct{2215};
t4000 = ct{2216};
t4001 = ct{2217};
t4003 = ct{2218};
t4005 = ct{2219};
t4007 = ct{2220};
t4008 = ct{2221};
t4009 = ct{2222};
t4010 = ct{2223};
t4011 = ct{2224};
t4012 = ct{2225};
t4013 = ct{2226};
t4014 = ct{2227};
t4015 = ct{2228};
t4019 = ct{2229};
t4020 = ct{2230};
t4021 = ct{2231};
t4022 = ct{2232};
t4023 = ct{2233};
t4024 = ct{2234};
t4025 = ct{2235};
t4026 = ct{2236};
t4027 = ct{2237};
t4028 = ct{2238};
t4029 = ct{2239};
t4030 = ct{2240};
t4031 = ct{2241};
t4032 = ct{2242};
t4033 = ct{2243};
t4034 = ct{2244};
t4035 = ct{2245};
t4036 = ct{2246};
t4038 = ct{2247};
t4040 = ct{2248};
t4041 = ct{2249};
t4042 = ct{2250};
t4043 = ct{2251};
t4046 = ct{2252};
t4047 = ct{2253};
t4048 = ct{2254};
t4050 = ct{2255};
t4051 = ct{2256};
t4052 = ct{2257};
t4053 = ct{2258};
t4054 = ct{2259};
t4056 = ct{2260};
t4058 = ct{2261};
t4059 = ct{2262};
t4061 = ct{2263};
t4063 = ct{2264};
t4064 = ct{2265};
t4065 = ct{2266};
t4066 = ct{2267};
t4068 = ct{2268};
t4070 = ct{2269};
t4071 = ct{2270};
t4072 = ct{2271};
t4073 = ct{2272};
t4074 = ct{2273};
t4077 = ct{2274};
t4078 = ct{2275};
t4081 = ct{2276};
t4083 = ct{2277};
t4084 = ct{2278};
t4085 = ct{2279};
t4086 = ct{2280};
t4087 = ct{2281};
t4089 = ct{2282};
t4090 = ct{2283};
t4092 = ct{2284};
t4093 = ct{2285};
t4094 = ct{2286};
t4095 = ct{2287};
t4096 = ct{2288};
t4097 = ct{2289};
t4098 = ct{2290};
t4099 = ct{2291};
t41 = ct{2292};
t410 = ct{2293};
t4100 = ct{2294};
t4101 = ct{2295};
t4104 = ct{2296};
t4105 = ct{2297};
t4108 = ct{2298};
t4109 = ct{2299};
t411 = ct{2300};
t4111 = ct{2301};
t4112 = ct{2302};
t4115 = ct{2303};
t4116 = ct{2304};
t4117 = ct{2305};
t4119 = ct{2306};
t412 = ct{2307};
t4120 = ct{2308};
t4121 = ct{2309};
t4122 = ct{2310};
t4123 = ct{2311};
t4126 = ct{2312};
t4128 = ct{2313};
t4129 = ct{2314};
t413 = ct{2315};
t4130 = ct{2316};
t4131 = ct{2317};
t4132 = ct{2318};
t4133 = ct{2319};
t4135 = ct{2320};
t4137 = ct{2321};
t4138 = ct{2322};
t4139 = ct{2323};
t414 = ct{2324};
t4140 = ct{2325};
t4141 = ct{2326};
t4143 = ct{2327};
t4144 = ct{2328};
t4145 = ct{2329};
t4146 = ct{2330};
t4147 = ct{2331};
t415 = ct{2332};
t4151 = ct{2333};
t4152 = ct{2334};
t4153 = ct{2335};
t4155 = ct{2336};
t4156 = ct{2337};
t4157 = ct{2338};
t4158 = ct{2339};
t4159 = ct{2340};
t4160 = ct{2341};
t4162 = ct{2342};
t4164 = ct{2343};
t4165 = ct{2344};
t4166 = ct{2345};
t4168 = ct{2346};
t4169 = ct{2347};
t4171 = ct{2348};
t4173 = ct{2349};
t4174 = ct{2350};
t4176 = ct{2351};
t4177 = ct{2352};
t4178 = ct{2353};
t4179 = ct{2354};
t4182 = ct{2355};
t4184 = ct{2356};
t4187 = ct{2357};
t4188 = ct{2358};
t4189 = ct{2359};
t4190 = ct{2360};
t4191 = ct{2361};
t4192 = ct{2362};
t4193 = ct{2363};
t4194 = ct{2364};
t4196 = ct{2365};
t4197 = ct{2366};
t4199 = ct{2367};
t420 = ct{2368};
t4201 = ct{2369};
t4203 = ct{2370};
t4204 = ct{2371};
t4206 = ct{2372};
t421 = ct{2373};
t4210 = ct{2374};
t4211 = ct{2375};
t4212 = ct{2376};
t4213 = ct{2377};
t4214 = ct{2378};
t4215 = ct{2379};
t4216 = ct{2380};
t4217 = ct{2381};
t4218 = ct{2382};
t4220 = ct{2383};
t4221 = ct{2384};
t4222 = ct{2385};
t4223 = ct{2386};
t4224 = ct{2387};
t4225 = ct{2388};
t4226 = ct{2389};
t4227 = ct{2390};
t4228 = ct{2391};
t4229 = ct{2392};
t4230 = ct{2393};
t4231 = ct{2394};
t4232 = ct{2395};
t4233 = ct{2396};
t4234 = ct{2397};
t4236 = ct{2398};
t4237 = ct{2399};
t4239 = ct{2400};
t4240 = ct{2401};
t4241 = ct{2402};
t4244 = ct{2403};
t4245 = ct{2404};
t4246 = ct{2405};
t4247 = ct{2406};
t4248 = ct{2407};
t4249 = ct{2408};
t425 = ct{2409};
t4250 = ct{2410};
t4252 = ct{2411};
t4253 = ct{2412};
t4255 = ct{2413};
t4256 = ct{2414};
t4258 = ct{2415};
t4259 = ct{2416};
t4261 = ct{2417};
t4262 = ct{2418};
t4263 = ct{2419};
t4264 = ct{2420};
t4267 = ct{2421};
t4268 = ct{2422};
t4269 = ct{2423};
t4272 = ct{2424};
t4273 = ct{2425};
t4274 = ct{2426};
t4276 = ct{2427};
t4277 = ct{2428};
t4278 = ct{2429};
t4280 = ct{2430};
t4281 = ct{2431};
t4282 = ct{2432};
t4286 = ct{2433};
t4290 = ct{2434};
t4295 = ct{2435};
t4298 = ct{2436};
t4299 = ct{2437};
t430 = ct{2438};
t4300 = ct{2439};
t4301 = ct{2440};
t4304 = ct{2441};
t4305 = ct{2442};
t4306 = ct{2443};
t4307 = ct{2444};
t4308 = ct{2445};
t431 = ct{2446};
t4311 = ct{2447};
t4312 = ct{2448};
t4316 = ct{2449};
t4320 = ct{2450};
t4323 = ct{2451};
t4324 = ct{2452};
t4326 = ct{2453};
t433 = ct{2454};
t4330 = ct{2455};
t4332 = ct{2456};
t4333 = ct{2457};
t4334 = ct{2458};
t4339 = ct{2459};
t4342 = ct{2460};
t4344 = ct{2461};
t4345 = ct{2462};
t4346 = ct{2463};
t4348 = ct{2464};
t4349 = ct{2465};
t4351 = ct{2466};
t4354 = ct{2467};
t4355 = ct{2468};
t4356 = ct{2469};
t4358 = ct{2470};
t436 = ct{2471};
t4360 = ct{2472};
t4361 = ct{2473};
t4364 = ct{2474};
t4365 = ct{2475};
t4367 = ct{2476};
t4368 = ct{2477};
t4371 = ct{2478};
t4372 = ct{2479};
t4375 = ct{2480};
t4382 = ct{2481};
t4393 = ct{2482};
t4395 = ct{2483};
t4399 = ct{2484};
t44 = ct{2485};
t4402 = ct{2486};
t4406 = ct{2487};
t4408 = ct{2488};
t4414 = ct{2489};
t4416 = ct{2490};
t4418 = ct{2491};
t4420 = ct{2492};
t4421 = ct{2493};
t4422 = ct{2494};
t4423 = ct{2495};
t4424 = ct{2496};
t4425 = ct{2497};
t4427 = ct{2498};
t4428 = ct{2499};
t4432 = ct{2500};
t4436 = ct{2501};
t4437 = ct{2502};
t4438 = ct{2503};
t4440 = ct{2504};
t4441 = ct{2505};
t4449 = ct{2506};
t445 = ct{2507};
t4453 = ct{2508};
t4454 = ct{2509};
t4457 = ct{2510};
t4458 = ct{2511};
t4461 = ct{2512};
t4467 = ct{2513};
t4468 = ct{2514};
t4469 = ct{2515};
t4472 = ct{2516};
t4475 = ct{2517};
t4476 = ct{2518};
t4477 = ct{2519};
t4478 = ct{2520};
t4479 = ct{2521};
t4481 = ct{2522};
t4486 = ct{2523};
t4487 = ct{2524};
t4488 = ct{2525};
t4490 = ct{2526};
t4492 = ct{2527};
t4494 = ct{2528};
t4495 = ct{2529};
t4496 = ct{2530};
t4497 = ct{2531};
t4506 = ct{2532};
t451 = ct{2533};
t4512 = ct{2534};
t4514 = ct{2535};
t4516 = ct{2536};
t4525 = ct{2537};
t4529 = ct{2538};
t4538 = ct{2539};
t4545 = ct{2540};
t4549 = ct{2541};
t4551 = ct{2542};
t4552 = ct{2543};
t4558 = ct{2544};
t4561 = ct{2545};
t4569 = ct{2546};
t4571 = ct{2547};
t4575 = ct{2548};
t4581 = ct{2549};
t4583 = ct{2550};
t459 = ct{2551};
t4597 = ct{2552};
t4598 = ct{2553};
t4602 = ct{2554};
t4603 = ct{2555};
t4611 = ct{2556};
t4616 = ct{2557};
t4628 = ct{2558};
t4641 = ct{2559};
t4646 = ct{2560};
t4649 = ct{2561};
t465 = ct{2562};
t4655 = ct{2563};
t4659 = ct{2564};
t4665 = ct{2565};
t4686 = ct{2566};
t4695 = ct{2567};
t4707 = ct{2568};
t4709 = ct{2569};
t4711 = ct{2570};
t4713 = ct{2571};
t4722 = ct{2572};
t4723 = ct{2573};
t4724 = ct{2574};
t4732 = ct{2575};
t4733 = ct{2576};
t4735 = ct{2577};
t4736 = ct{2578};
t4740 = ct{2579};
t4745 = ct{2580};
t4746 = ct{2581};
t4752 = ct{2582};
t4762 = ct{2583};
t4772 = ct{2584};
t4776 = ct{2585};
t4784 = ct{2586};
t4789 = ct{2587};
t4796 = ct{2588};
t48 = ct{2589};
t4802 = ct{2590};
t4809 = ct{2591};
t4821 = ct{2592};
t4823 = ct{2593};
t483 = ct{2594};
t4848 = ct{2595};
t4849 = ct{2596};
t485 = ct{2597};
t4866 = ct{2598};
t487 = ct{2599};
t4873 = ct{2600};
t4878 = ct{2601};
t488 = ct{2602};
t4889 = ct{2603};
t4895 = ct{2604};
t49 = ct{2605};
t4909 = ct{2606};
t491 = ct{2607};
t4913 = ct{2608};
t4922 = ct{2609};
t4923 = ct{2610};
t4925 = ct{2611};
t4931 = ct{2612};
t4932 = ct{2613};
t4933 = ct{2614};
t4936 = ct{2615};
t4938 = ct{2616};
t4942 = ct{2617};
t4944 = ct{2618};
t4945 = ct{2619};
t4946 = ct{2620};
t4953 = ct{2621};
t4954 = ct{2622};
t496 = ct{2623};
t4964 = ct{2624};
t4966 = ct{2625};
t4967 = ct{2626};
t4975 = ct{2627};
t4976 = ct{2628};
t4986 = ct{2629};
t4987 = ct{2630};
t4988 = ct{2631};
t4993 = ct{2632};
t4995 = ct{2633};
t5 = ct{2634};
t50 = ct{2635};
t501 = ct{2636};
t502 = ct{2637};
t5021 = ct{2638};
t5032 = ct{2639};
t5036 = ct{2640};
t504 = ct{2641};
t5042 = ct{2642};
t5046 = ct{2643};
t5051 = ct{2644};
t5053 = ct{2645};
t5054 = ct{2646};
t5058 = ct{2647};
t5059 = ct{2648};
t5066 = ct{2649};
t5067 = ct{2650};
t5072 = ct{2651};
t5078 = ct{2652};
t5080 = ct{2653};
t5083 = ct{2654};
t5092 = ct{2655};
t51 = ct{2656};
t5103 = ct{2657};
t5109 = ct{2658};
t5153 = ct{2659};
t5179 = ct{2660};
t519 = ct{2661};
t5198 = ct{2662};
t5202 = ct{2663};
t5206 = ct{2664};
t5208 = ct{2665};
t5227 = ct{2666};
t523 = ct{2667};
t524 = ct{2668};
t5265 = ct{2669};
t527 = ct{2670};
t5275 = ct{2671};
t530 = ct{2672};
t5300 = ct{2673};
t5317 = ct{2674};
t534 = ct{2675};
t5351 = ct{2676};
t5358 = ct{2677};
t5363 = ct{2678};
t537 = ct{2679};
t539 = ct{2680};
t5399 = ct{2681};
t54 = ct{2682};
t541 = ct{2683};
t542 = ct{2684};
t5420 = ct{2685};
t5424 = ct{2686};
t5427 = ct{2687};
t5431 = ct{2688};
t5433 = ct{2689};
t5438 = ct{2690};
t544 = ct{2691};
t5448 = ct{2692};
t5453 = ct{2693};
t546 = ct{2694};
t5476 = ct{2695};
t5488 = ct{2696};
t5498 = ct{2697};
t55 = ct{2698};
t550 = ct{2699};
t553 = ct{2700};
t5530 = ct{2701};
t5539 = ct{2702};
t5547 = ct{2703};
t5565 = ct{2704};
t557 = ct{2705};
t5576 = ct{2706};
t558 = ct{2707};
t5582 = ct{2708};
t5598 = ct{2709};
t56 = ct{2710};
t5674 = ct{2711};
t5690 = ct{2712};
t5705 = ct{2713};
t5706 = ct{2714};
t5716 = ct{2715};
t573 = ct{2716};
t574 = ct{2717};
t575 = ct{2718};
t5788 = ct{2719};
t5791 = ct{2720};
t5800 = ct{2721};
t5869 = ct{2722};
t587 = ct{2723};
t59 = ct{2724};
t595 = ct{2725};
t603 = ct{2726};
t61 = ct{2727};
t614 = ct{2728};
t628 = ct{2729};
t629 = ct{2730};
t634 = ct{2731};
t641 = ct{2732};
t65 = ct{2733};
t650 = ct{2734};
t651 = ct{2735};
t655 = ct{2736};
t6554 = ct{2737};
t6556 = ct{2738};
t657 = ct{2739};
t6599 = ct{2740};
t6627 = ct{2741};
t6629 = ct{2742};
t664 = ct{2743};
t665 = ct{2744};
t666 = ct{2745};
t667 = ct{2746};
t668 = ct{2747};
t669 = ct{2748};
t675 = ct{2749};
t68 = ct{2750};
t693 = ct{2751};
t7 = ct{2752};
t71 = ct{2753};
t721 = ct{2754};
t724 = ct{2755};
t73 = ct{2756};
t731 = ct{2757};
t732 = ct{2758};
t736 = ct{2759};
t741 = ct{2760};
t744 = ct{2761};
t753 = ct{2762};
t754 = ct{2763};
t755 = ct{2764};
t756 = ct{2765};
t757 = ct{2766};
t759 = ct{2767};
t760 = ct{2768};
t761 = ct{2769};
t762 = ct{2770};
t764 = ct{2771};
t765 = ct{2772};
t769 = ct{2773};
t772 = ct{2774};
t774 = ct{2775};
t776 = ct{2776};
t778 = ct{2777};
t792 = ct{2778};
t795 = ct{2779};
t797 = ct{2780};
t799 = ct{2781};
t8 = ct{2782};
t802 = ct{2783};
t803 = ct{2784};
t806 = ct{2785};
t817 = ct{2786};
t818 = ct{2787};
t820 = ct{2788};
t824 = ct{2789};
t828 = ct{2790};
t831 = ct{2791};
t834 = ct{2792};
t837 = ct{2793};
t838 = ct{2794};
t841 = ct{2795};
t842 = ct{2796};
t843 = ct{2797};
t844 = ct{2798};
t846 = ct{2799};
t847 = ct{2800};
t848 = ct{2801};
t850 = ct{2802};
t851 = ct{2803};
t852 = ct{2804};
t853 = ct{2805};
t855 = ct{2806};
t865 = ct{2807};
t867 = ct{2808};
t868 = ct{2809};
t870 = ct{2810};
t871 = ct{2811};
t872 = ct{2812};
t874 = ct{2813};
t875 = ct{2814};
t876 = ct{2815};
t877 = ct{2816};
t885 = ct{2817};
t886 = ct{2818};
t888 = ct{2819};
t890 = ct{2820};
t891 = ct{2821};
t892 = ct{2822};
t896 = ct{2823};
t898 = ct{2824};
t9 = ct{2825};
t901 = ct{2826};
t902 = ct{2827};
t903 = ct{2828};
t904 = ct{2829};
t906 = ct{2830};
t907 = ct{2831};
t909 = ct{2832};
t914 = ct{2833};
t915 = ct{2834};
t916 = ct{2835};
t924 = ct{2836};
t925 = ct{2837};
t926 = ct{2838};
t928 = ct{2839};
t947 = ct{2840};
t949 = ct{2841};
t950 = ct{2842};
t952 = ct{2843};
t954 = ct{2844};
t955 = ct{2845};
t957 = ct{2846};
t964 = ct{2847};
t965 = ct{2848};
t972 = ct{2849};
t977 = ct{2850};
t979 = ct{2851};
t983 = ct{2852};
t987 = ct{2853};
t991 = ct{2854};
t992 = ct{2855};
t993 = ct{2856};
t994 = ct{2857};
t995 = ct{2858};
t4289 = t724+t778+t1296+t1299+t1339;
t4296 = t1144+t2039+t2041;
t4302 = Mb.*t1622.*t3836;
t4309 = t4096.*3.36554e-3;
t4313 = t1329+t1995+t2019;
t4315 = -t4305;
t4317 = -t4307;
t4318 = t4105.*3.36554e-3;
t4319 = Mb.*t2527.*t3139;
t4322 = t4111.*3.36554e-3;
t4327 = Mb.*t2527.*t3206;
t4329 = -t4320;
t4336 = Mb.*t2627.*t3206;
t4337 = t4111.*3.367829185e-3;
t4341 = t4111.*8.56645e-6;
t4343 = t1407+t2080+t2160;
t4352 = t1430.*t4063;
t4353 = dpsi1.*t4344;
t4357 = t41+t431+t483+t792+t909+t1394+t1623;
t4366 = Mt.*t4.*t10.*t4344;
t4373 = Mt.*t2319.*t3770;
t4374 = t903.*t4264;
t4376 = Mt.*t5.*t30.*t4344;
t4378 = Mt.*t5.*t34.*t4344;
t4392 = t3123+t3195;
t4396 = t1331+t2381+t2448;
t4401 = Mt.*t1528.*t4132;
t4403 = t4272.*3.36554e-3;
t4405 = Mt.*t381.*t4344;
t4410 = t1383+t2417+t2496;
t4413 = Mt.*t421.*t4344;
t4415 = t979+t1051+t1224+t1497+t1575;
t4426 = t1412+t2459+t2606;
t4431 = Mt.*t1734.*t4132;
t4433 = dphi1.*t4423;
t4434 = dth2.*t4423;
t4435 = t965+t1042+t1341+t1498+t1574;
t4442 = -t4428;
t4444 = -t4436;
t4445 = t1440+t2484+t2573;
t4447 = t1615+t2371+t2548;
t4450 = -t4441;
t4452 = t1523+t2511+t2602;
t4455 = -t4449;
t4465 = Mb.*t3139.*t3836;
t4470 = Mt.*t2174.*t4132;
t4471 = t1687+t2644+t2675;
t4480 = t1430.*t4299;
t4482 = dth2.*t4468;
t4483 = t496.*t4422;
t4485 = t11.*t420.*t4422;
t4489 = -Mt.*t4132.*(t451-t831+T_cg_H.*(t214-t541));
t4493 = Mt.*t2319.*t4115;
t4500 = t3564+t3669;
t4501 = Mt.*t2319.*t4132;
t4502 = -t4488;
t4503 = Mt.*t4132.*(t451-t831+T_cg_H.*(t214-t541));
t4505 = t3640+t3641;
t4508 = t1438+t2868+t2935;
t4513 = t4399.*(-3.36554e-3);
t4515 = t4399.*3.36554e-3;
t4517 = t3656+t3754;
t4518 = t3725+t3726;
t4519 = t817.*t4422;
t4521 = -t4516;
t4522 = t1594+t2866+t2934;
t4523 = -t4422.*(t105-t465);
t4526 = Mt.*t1381.*t4344;
t4528 = t903.*t4437;
t4532 = Mt.*t2730.*t4132;
t4533 = t4422.*(t105-t465).*(-1.0./2.0);
t4539 = t1166+t1168+t2532+t2575;
t4542 = t964.*t4437;
t4546 = Mt.*t2914.*t4132;
t4550 = t1031.*t4437;
t4553 = Mt.*t4132.*(-t130+t436+t523-t657+t769);
t4555 = t1985+t2793+t2852;
t4557 = Mt.*t1727.*t4344;
t4563 = -t4437.*(t534-t546);
t4564 = Mt.*t3770.*t3940;
t4566 = -t4561;
t4573 = t1654+t3192+t3197;
t4574 = dth2.*t4569;
t4576 = t1430.*t4422;
t4589 = t1505.*t4437;
t4591 = t1510.*t4437;
t4592 = t1815+t1824+t1991+t2124;
t4604 = Mt.*t2325.*t4344;
t4610 = Mt.*t3679.*t4132;
t4613 = Mt.*t3770.*t4112;
t4615 = t4422.*(t105-t465).*(-3.36554e-3);
t4617 = t1881+t1887+t2070+t2169;
t4618 = t1937+t1955+t1990+t2001;
t4621 = -t4611;
t4622 = -Mt.*t4344.*(t431+t909+T_cg_H.*(t195-t634));
t4625 = -t4616;
t4630 = Mt.*t4344.*(t431+t909+T_cg_H.*(t195-t634));
t4636 = t4422.*(t105-t465).*(-3.372786875e-3);
t4637 = t4422.*(t105-t465).*(-9.53094055e-4);
t4638 = t1891+t1989+t2085+t2122;
t4643 = t1750+t1817+t2369+t2370;
t4645 = t1756+t1826+t2313+t2455;
t4651 = Mt.*t2763.*t4344;
t4660 = Mt.*t2915.*t4344;
t4661 = -t4655;
t4662 = Mt.*t3940.*t4115;
t4663 = Mt.*t3940.*t4132;
t4664 = Mt.*t4344.*(-t120+t425+t519-t651+t765);
t4668 = t2209+t3348+t3353;
t4669 = t4437.*(t534-t546).*(-3.36554e-3);
t4671 = Mt.*t3969.*t4132;
t4672 = t950+t1054+t1488+t1582+t1749+t1822;
t4676 = t1414+t1565+t2922+t3039;
t4677 = t1483+t1491+t2969+t2986;
t4692 = t1065+t1123+t1506+t1641+t1763+t1774;
t4699 = t874+t1060+t1435+t1517+t1932+t2088;
t4701 = t2611+t3421+t3452;
t4708 = ITail.*t4072.*t4173;
t4715 = t875+t1118+t1466+t1550+t2032+t2247;
t4718 = t2423+t3569+t3667;
t4721 = t1123+t1182+t1694+t1755+t1763+t1774;
t4725 = Mt.*t3770.*t4344;
t4734 = t915+t1120+t1646+t1705+t2002+t2006;
t4737 = t2658+t3636+t3733;
t4738 = t1052+t1261+t1509+t1579+t2083+t2111;
t4741 = t2621+t3688+t3786;
t4744 = t2649+t3713+t3773;
t4747 = -t4745;
t4748 = t744+t1171+t1236+t1642+t2583+t2654;
t4751 = ITail.*t4173.*t4227;
t4756 = -dx.*(-t754+t1167-t1635+t2574+Mt.*t9.*t10.*(t433-t828+T_cg_H.*(t197-t537))+B_cg_H.*Mb.*t9.*t10.*(t197-t537));
t4758 = Mt.*t3971.*t4344;
t4760 = t892+t1119+t1791+t1855+t2035+t2076;
t4763 = t2536+t2537+t2541+t2542;
t4766 = dth2.*t4762;
t4770 = t1311+t1332+t1567+t1591+t2084+t2112;
t4771 = ITail.*t4173.*t4286;
t4775 = t2955+t3796+t3803;
t4778 = t837+t1197+t1275+t1671+t2672+t2731;
t4782 = t842+t1202+t1285+t1677+t2674+t2732;
t4787 = t2748+t3843+t3864;
t4794 = t2647+t3868+t3899;
t4795 = t2645+t2684+t2685+t2691;
t4800 = -ITail.*t3961.*(t1352-t2496+(t1430.*(t105-t465))./2.0);
t4801 = Mt.*t4115.*t4344;
t4805 = ITail.*t3961.*(t1352-t2496+(t1430.*(t105-t465))./2.0);
t4807 = -ITail.*t4072.*(t1332+t2368+t1512.*(t105-t465));
t4818 = t1261+t1312+t1830+t1862+t2083+t2111;
t4828 = t1129+t1184+t2078+t2082+t2193+t2199;
t4830 = t2771+t2901+t2904+t2906;
t4834 = t1379+t1450+t1871+t1921+t2101+t2115;
t4837 = t841+t1422+t1496+t1684+t2907+t2999;
t4839 = -ITail.*t4173.*(t1352-t2496+(t1430.*(t105-t465))./2.0);
t4842 = t834+t1418+t1484+t1668+t2895+t2987;
t4846 = ITail.*t4173.*(t1352-t2496+(t1430.*(t105-t465))./2.0);
t4847 = ITail.*(t1352-t2496+(t1430.*(t105-t465))./2.0).*(-t1262+t1701+t9.*t868.*(t105-t465));
t4854 = -ITail.*t4227.*(t1332+t2368+t1512.*(t105-t465));
t4859 = t891+t1413+t1489+t1729+t2921+t2967;
t4860 = t898+t1421+t1500+t1743+t2937+t2975;
t4862 = -ITail.*t4173.*(-t1412+t2419+(t1510.*(t103-t544))./2.0);
t4864 = ITail.*t4227.*(t1332+t2368+t1512.*(t105-t465));
t4870 = -dz.*(t838-t1413+t1672-t2921+Mt.*t420.*(t433-t828+T_cg_H.*(t197-t537))+B_cg_H.*Mb.*t420.*(t197-t537));
t4871 = -dphi2.*(t843-t1421+t1685-t2937+Mt.*t420.*(t451-t831+T_cg_H.*(t214-t541))+B_cg_H.*Mb.*t420.*(t214-t541));
t4872 = -dth2.*(t843-t1421+t1685-t2937+Mt.*t420.*(t451-t831+T_cg_H.*(t214-t541))+B_cg_H.*Mb.*t420.*(t214-t541));
t4874 = t1195+t1256+t2125+t2129+t2232+t2233;
t4877 = dth2.*t4866;
t4880 = dth2.*(t843-t1421+t1685-t2937+Mt.*t420.*(t451-t831+T_cg_H.*(t214-t541))+B_cg_H.*Mb.*t420.*(t214-t541));
t4882 = t1402+t1555+t1880+t1911+t2194+t2236;
t4883 = t2271+t4096+t4123;
t4890 = ITail.*(t1352-t2496+(t1430.*(t105-t465))./2.0).*(-t947+t1240.*(t105-t465)+t903.*(t534-t546));
t4892 = -ITail.*t4286.*(t1332+t2368+t1512.*(t105-t465));
t4897 = t1319+t1448+t2103+t2120+t2170+t2270;
t4898 = -ITail.*t4255.*(-t1412+t2419+(t1510.*(t103-t544))./2.0);
t4904 = ITail.*t4255.*(-t1412+t2419+(t1510.*(t103-t544))./2.0);
t4908 = t1190+t1602+t1885+t1894+t2454+t2595;
t4912 = ITail.*t4173.*t4490;
t4921 = -ITail.*t4311.*(-t1412+t2419+(t1510.*(t103-t544))./2.0);
t4927 = ITail.*t4311.*(-t1412+t2419+(t1510.*(t103-t544))./2.0);
t4930 = -ITail.*t4173.*(-t993+t1535+t1540-t1552+(t3.*t496.*(t105-t465))./2.0);
t4934 = ITail.*t4173.*(-t993+t1535+t1540-t1552+(t3.*t496.*(t105-t465))./2.0);
t4939 = ITail.*t4071.*t4575;
t4941 = t4173.*t4549;
t4949 = t3124+t3133+t3281+t3365;
t4950 = -t4945;
t4960 = t1548+t1601+t2304+t2330+t2333+t2355;
t4961 = t1690+t1745+t1968+t1980+t2457+t2498;
t4968 = t885+t1658+t1726+t1758+t3398+t3468;
t4969 = -t4964;
t4978 = -ITail.*t4408.*(t1368-t2524+t1430.*(t197-t537));
t4979 = t928+t1657+t1725+t1831+t3397+t3467;
t4990 = -ITail.*t3961.*(t1846+t2413+(t964.*(t105-t465))./2.0+(t1430.*(t103-t544))./2.0);
t4991 = dphi2.*t4986;
t4992 = dphi2.*t4987;
t4997 = ITail.*t3961.*(t1846+t2413+(t964.*(t105-t465))./2.0+(t1430.*(t103-t544))./2.0);
t4998 = t4173.*t4602;
t5004 = -ITail.*t4575.*(-t1355+t1789+(t9.*t868.*(t105-t465))./2.0);
t5015 = t1237+t1366+t2538+t2539+t2830+t2899;
t5017 = -ITail.*t4490.*(t1332+t2368+t1512.*(t105-t465));
t5020 = ITail.*t4408.*t4461;
t5024 = -ITail.*t4173.*(t994-t1742+t1790+(t3.*t818.*(t105-t465))./2.0+(t3.*t872.*(t103-t544))./2.0);
t5029 = ITail.*t4173.*t4646;
t5030 = t4173.*t4649;
t5031 = ITail.*t4173.*(t994-t1742+t1790+(t3.*t818.*(t105-t465))./2.0+(t3.*t872.*(t103-t544))./2.0);
t5033 = ITail.*t4071.*t4686;
t5038 = -ITail.*t4408.*(t1365-t2831+t1505.*(t534-t546));
t5041 = -ITail.*t4575.*(-t1017+(t1240.*(t105-t465))./2.0+(t903.*(t534-t546))./2.0);
t5048 = -ITail.*t4476.*(t1368-t2524+t1430.*(t197-t537));
t5055 = ITail.*(t1332+t2368+t1512.*(t105-t465)).*(-t993+t1535+t1540-t1552+(t3.*t496.*(t105-t465))./2.0);
t5061 = -ITail.*t3961.*(t853+t1084-t1466-t2032-t2247+(t11.*t542.*(t105-t465))./2.0);
t5063 = -t3961.*(t2387-t3667+t1430.*(t105-t465).*9.53094055e-4);
t5065 = t3509+t3537+t3544+t3545;
t5074 = t3961.*(t2387-t3667+t1430.*(t105-t465).*9.53094055e-4);
t5076 = ITail.*t3961.*t4722;
t5082 = -t4549.*(t1332+t2368+t1512.*(t105-t465));
t5088 = ITail.*(-t1262+t1701+t9.*t868.*(t105-t465)).*(t1846+t2413+(t964.*(t105-t465))./2.0+(t1430.*(t103-t544))./2.0);
t5096 = t3509+t3537+t3631+t3632;
t5097 = t3544+t3545+t3607+t3645;
t5098 = ITail.*t3961.*t4735;
t5099 = ITail.*t4461.*t4476;
t5114 = ITail.*(-t947+t1240.*(t105-t465)+t903.*(t534-t546)).*(t1846+t2413+(t964.*(t105-t465))./2.0+(t1430.*(t103-t544))./2.0);
t5119 = -ITail.*t4476.*(t1365-t2831+t1505.*(t534-t546));
t5126 = -ITail.*t4686.*(-t1355+t1789+(t9.*t868.*(t105-t465))./2.0);
t5128 = ITail.*t4476.*(t1365-t2831+t1505.*(t534-t546));
t5131 = -ITail.*t3961.*(t865+t1086-t1855-t2076+(t1181.*(t105-t465))./2.0+(t11.*t381.*(t534-t546))./2.0);
t5143 = -ITail.*t4173.*(t853+t1084-t1466-t2032-t2247+(t11.*t542.*(t105-t465))./2.0);
t5147 = -t4173.*(t2387-t3667+t1430.*(t105-t465).*9.53094055e-4);
t5150 = ITail.*(-t1262+t1701+t9.*t868.*(t105-t465)).*(t853+t1084-t1466-t2032-t2247+(t11.*t542.*(t105-t465))./2.0);
t5152 = (t2387-t3667+t1430.*(t105-t465).*9.53094055e-4).*(-t1262+t1701+t9.*t868.*(t105-t465));
t5156 = ITail.*t4173.*t4722;
t5159 = -t4602.*(t1332+t2368+t1512.*(t105-t465));
t5161 = t4173.*(t2387-t3667+t1430.*(t105-t465).*9.53094055e-4);
t5165 = t4602.*(t1332+t2368+t1512.*(t105-t465));
t5177 = -ITail.*t3938.*(t2582-t2684+(t1510.*(t197-t537))./2.0+(t1505.*(t214-t541))./2.0);
t5184 = ITail.*t4173.*t4735;
t5189 = t3753+t3777+t3778+t3783;
t5191 = -t4173.*(-t2621+t3659+t1510.*(t103-t544).*8.56645e-6);
t5194 = ITail.*(t1332+t2368+t1512.*(t105-t465)).*(t994-t1742+t1790+(t3.*t818.*(t105-t465))./2.0+(t3.*t872.*(t103-t544))./2.0);
t5197 = (-t947+t1240.*(t105-t465)+t903.*(t534-t546)).*(t2387-t3667+t1430.*(t105-t465).*9.53094055e-4);
t5201 = -ITail.*t4646.*(t1332+t2368+t1512.*(t105-t465));
t5203 = -t4649.*(t1332+t2368+t1512.*(t105-t465));
t5205 = -ITail.*t4722.*(-t947+t1240.*(t105-t465)+t903.*(t534-t546));
t5207 = ITail.*t4646.*(t1332+t2368+t1512.*(t105-t465));
t5214 = -ITail.*t4173.*(t865+t1086-t1855-t2076+(t1181.*(t105-t465))./2.0+(t11.*t381.*(t534-t546))./2.0);
t5219 = -ITail.*t4735.*(-t947+t1240.*(t105-t465)+t903.*(t534-t546));
t5223 = ITail.*(-t1262+t1701+t9.*t868.*(t105-t465)).*(t865+t1086-t1855-t2076+(t1181.*(t105-t465))./2.0+(t11.*t381.*(t534-t546))./2.0);
t5230 = -t4255.*(-t2621+t3659+t1510.*(t103-t544).*8.56645e-6);
t5232 = ITail.*t4735.*(-t947+t1240.*(t105-t465)+t903.*(t534-t546));
t5240 = ITail.*(t1332+t2368+t1512.*(t105-t465)).*(t1846+t2413+(t964.*(t105-t465))./2.0+(t1430.*(t103-t544))./2.0);
t5241 = t4255.*(-t2621+t3659+t1510.*(t103-t544).*8.56645e-6);
t5283 = -t4311.*(-t2621+t3659+t1510.*(t103-t544).*8.56645e-6);
t5287 = t4311.*(-t2621+t3659+t1510.*(t103-t544).*8.56645e-6);
t5291 = t4551.*t4575;
t5293 = ITail.*(-t1412+t2419+(t1510.*(t103-t544))./2.0).*(t995+t1064-t1506+t1598-t1763-t1774);
t5308 = ITail.*(t1332+t2368+t1512.*(t105-t465)).*(t853+t1084-t1466-t2032-t2247+(t11.*t542.*(t105-t465))./2.0);
t5310 = -t5300;
t5319 = -ITail.*t3938.*(-t1189+t1195-t2210+t2241+t2248+(t8.*t872.*(t534-t546))./2.0);
t5323 = t1839+t2096+t2605+t2717+t3289+t3438;
t5324 = -ITail.*t4722.*(t1332+t2368+t1512.*(t105-t465));
t5328 = ITail.*t4722.*(t1332+t2368+t1512.*(t105-t465));
t5344 = -ITail.*t4735.*(t1332+t2368+t1512.*(t105-t465));
t5354 = ITail.*(-t1412+t2419+(t1510.*(t103-t544))./2.0).*(t1064+t1137-t1694+t1698-t1763-t1774);
t5372 = ITail.*(-t1412+t2419+(t1510.*(t103-t544))./2.0).*(t867+t1059-t1646-t1705+t1938-t2002);
t5374 = ITail.*(t1332+t2368+t1512.*(t105-t465)).*(t865+t1086-t1855-t2076+(t1181.*(t105-t465))./2.0+(t11.*t381.*(t534-t546))./2.0);
t5379 = -t4408.*(t2591-t3773+t1430.*(t197-t537).*1.90524867e-3);
t5380 = -t4575.*(-t2388+t3008+t9.*t868.*(t105-t465).*9.53094055e-4);
t5390 = t1814+t2097+t3010+t3080+t3287+t3291;
t5412 = t4551.*t4686;
t5417 = -t4575.*(-t1974+t1240.*(t105-t465).*9.53094055e-4+t903.*(t534-t546).*9.53094055e-4);
t5445 = -t5433;
t5452 = -t4408.*(t2587-t3868+t1505.*(t534-t546).*1.90524867e-3);
t5456 = -ITail.*t4408.*(t2582-t2684+(t1510.*(t197-t537))./2.0+(t1505.*(t214-t541))./2.0);
t5460 = -t4476.*(t2591-t3773+t1430.*(t197-t537).*1.90524867e-3);
t5490 = -t3961.*(t3070+t3563+t964.*(t105-t465).*9.53094055e-4+t1430.*(t103-t544).*9.53094055e-4);
t5492 = t4173.*t4936;
t5493 = -t4686.*(-t2388+t3008+t9.*t868.*(t105-t465).*9.53094055e-4);
t5494 = t3961.*(t3070+t3563+t964.*(t105-t465).*9.53094055e-4+t1430.*(t103-t544).*9.53094055e-4);
t5518 = -t4476.*(t2587-t3868+t1505.*(t534-t546).*1.90524867e-3);
t5523 = -ITail.*t4476.*(t2582-t2684+(t1510.*(t197-t537))./2.0+(t1505.*(t214-t541))./2.0);
t5524 = t4476.*(t2587-t3868+t1505.*(t534-t546).*1.90524867e-3);
t5529 = -t4173.*(-t2058+t2688+t2700-t2718+t3.*t496.*(t105-t465).*9.53094055e-4);
t5538 = t4173.*(-t2058+t2688+t2700-t2718+t3.*t496.*(t105-t465).*9.53094055e-4);
t5548 = t2053+t2469+t3072+t3077+t3606+t3695;
t5552 = -t3938.*(t2449.*3.36554e-3+t3490+t3556+t3557);
t5556 = t2215+t2303+t3356+t3366+t3450+t3453;
t5566 = t2505+t2714+t3114+t3165+t3400+t3462;
t5569 = -ITail.*t3938.*(t1255-t1465+t2578+t2579-t2997+(t1430.*(t539+t641))./2.0);
t5588 = (-t1262+t1701+t9.*t868.*(t105-t465)).*(t3070+t3563+t964.*(t105-t465).*9.53094055e-4+t1430.*(t103-t544).*9.53094055e-4);
t5607 = t2238+t2755+t3119+t3130+t3599+t3729;
t5620 = (-t947+t1240.*(t105-t465)+t903.*(t534-t546)).*(t3070+t3563+t964.*(t105-t465).*9.53094055e-4+t1430.*(t103-t544).*9.53094055e-4);
t5652 = -dth1.*(-t754+t1167-t1635+t2574+t4628+Mt.*t9.*t10.*(t433-t828+T_cg_H.*(t197-t537))+B_cg_H.*Mb.*t9.*t10.*(t197-t537));
t5657 = -t4936.*(t1332+t2368+t1512.*(t105-t465));
t5660 = dphi1.*(t834+t1484+t1668+t2987-t4468-Mt.*t382.*(t433-t828+T_cg_H.*(t197-t537))-B_cg_H.*Mb.*t382.*(t197-t537));
t5662 = dth1.*(-t754+t1167-t1635+t2574+t4628+Mt.*t9.*t10.*(t433-t828+T_cg_H.*(t197-t537))+B_cg_H.*Mb.*t9.*t10.*(t197-t537));
t5664 = -t4173.*(t2059-t2952+t3009+t3.*t818.*(t105-t465).*9.53094055e-4+t3.*t872.*(t103-t544).*9.53094055e-4);
t5668 = -ITail.*t4476.*(-t1189+t1195-t2210+t2241+t2248+(t8.*t872.*(t534-t546))./2.0);
t5672 = t4173.*(t2059-t2952+t3009+t3.*t818.*(t105-t465).*9.53094055e-4+t3.*t872.*(t103-t544).*9.53094055e-4);
t5685 = -t3938.*(t3716-t3777+t1510.*(t197-t537).*9.52624335e-4+t1505.*(t214-t541).*9.52624335e-4);
t5696 = (-t2621+t3659+t1510.*(t103-t544).*8.56645e-6).*(t995+t1064-t1506+t1598-t1763-t1774);
t5697 = (t1332+t2368+t1512.*(t105-t465)).*(-t2058+t2688+t2700-t2718+t3.*t496.*(t105-t465).*9.53094055e-4);
t5702 = t2883+t2956+t3220+t3238+t3602+t3661;
t5703 = t2706+t2754+t3512+t3528+t3534+t3552;
t5713 = -t5705;
t5724 = -t5716;
t5730 = (t1332+t2368+t1512.*(t105-t465)).*(t3070+t3563+t964.*(t105-t465).*9.53094055e-4+t1430.*(t103-t544).*9.53094055e-4);
t5738 = (-t2621+t3659+t1510.*(t103-t544).*8.56645e-6).*(t1064+t1137-t1694+t1698-t1763-t1774);
t5749 = (-t2621+t3659+t1510.*(t103-t544).*8.56645e-6).*(t867+t1059-t1646-t1705+t1938-t2002);
t5757 = t4173.*t5208;
t5779 = t3961.*(-t1806+t2096+t2605+t2717+t3289+t3438);
t5785 = (t1332+t2368+t1512.*(t105-t465)).*(t2059-t2952+t3009+t3.*t818.*(t105-t465).*9.53094055e-4+t3.*t872.*(t103-t544).*9.53094055e-4);
t5790 = -t4408.*(t2449.*3.36554e-3+t3490+t3556+t3557);
t5795 = t4408.*(t2449.*3.36554e-3+t3490+t3556+t3557);
t5798 = (t1332+t2368+t1512.*(t105-t465)).*(t2449.*3.36554e-3+t3490-t3632+t1510.*(t105-t465).*3.372786875e-3);
t5806 = (-t1331+t2317+t1510.*(t103-t544)).*(t2449.*3.367829185e-3+t3556+t3557+t3576);
t5808 = -ITail.*t4408.*(t1255-t1465+t2578+t2579-t2997+(t1430.*(t539+t641))./2.0);
t5809 = t3961.*t5351;
t5815 = ITail.*t4408.*(t1255-t1465+t2578+t2579-t2997+(t1430.*(t539+t641))./2.0);
t5832 = -t3961.*(t1784+t2057-t3080-t3287+t1181.*(t105-t465).*9.53094055e-4+t11.*t381.*(t534-t546).*9.53094055e-4);
t5837 = t4173.*(-t1806+t2096+t2605+t2717+t3289+t3438);
t5840 = -(-t1262+t1701+t9.*t868.*(t105-t465)).*(-t1806+t2096+t2605+t2717+t3289+t3438);
t5842 = -t4476.*(t2449.*3.36554e-3+t3490+t3556+t3557);
t5843 = t4173.*(t2135-t2468+t2699+t2738+t2950+t3105);
t5846 = t4476.*(t2449.*3.36554e-3+t3490+t3556+t3557);
t5857 = t4173.*t5351;
t5866 = -t5208.*(t1332+t2368+t1512.*(t105-t465));
t5867 = -t4408.*(t3716-t3777+t1510.*(t197-t537).*9.52624335e-4+t1505.*(t214-t541).*9.52624335e-4);
t5870 = t5208.*(t1332+t2368+t1512.*(t105-t465));
t5874 = -t4173.*(t1784+t2057-t3080-t3287+t1181.*(t105-t465).*9.53094055e-4+t11.*t381.*(t534-t546).*9.53094055e-4);
t5878 = -t5351.*(-t947+t1240.*(t105-t465)+t903.*(t534-t546));
t5880 = (-t1262+t1701+t9.*t868.*(t105-t465)).*(t1784+t2057-t3080-t3287+t1181.*(t105-t465).*9.53094055e-4+t11.*t381.*(t534-t546).*9.53094055e-4);
t5887 = t5351.*(-t947+t1240.*(t105-t465)+t903.*(t534-t546));
t5905 = -t4476.*(t3716-t3777+t1510.*(t197-t537).*9.52624335e-4+t1505.*(t214-t541).*9.52624335e-4);
t5907 = t1978+t2008+t3922+t3942+t4105+t4159;
t5926 = -(t1332+t2368+t1512.*(t105-t465)).*(-t1806+t2096+t2605+t2717+t3289+t3438);
t5932 = -t3938.*(t2215-t2237+t3424+t3427-t3439+t8.*t872.*(t534-t546).*9.52624335e-4);
t5933 = (t1332+t2368+t1512.*(t105-t465)).*(-t1806+t2096+t2605+t2717+t3289+t3438);
t5936 = -(t1332+t2368+t1512.*(t105-t465)).*(t2135-t2468+t2699+t2738+t2950+t3105);
t5939 = (t1332+t2368+t1512.*(t105-t465)).*(t2135-t2468+t2699+t2738+t2950+t3105);
t5949 = -t5351.*(t1332+t2368+t1512.*(t105-t465));
t5963 = (t1332+t2368+t1512.*(t105-t465)).*(t1784+t2057-t3080-t3287+t1181.*(t105-t465).*9.53094055e-4+t11.*t381.*(t534-t546).*9.53094055e-4);
t5971 = -t3938.*(-t2503+t2754+t3433-t3460+t3506+t4.*t871.*(t534-t546).*9.52624335e-4);
t5984 = t3938.*(t2883+t2956-t3186-t3199+t3602+t3661);
t5985 = t3938.*(t2706-t2712+t3512+t3528+t3534+t3552);
t6049 = -t4408.*(-t2503+t2754+t3433-t3460+t3506+t4.*t871.*(t534-t546).*9.52624335e-4);
t6051 = -t4476.*(t2215-t2237+t3424+t3427-t3439+t8.*t872.*(t534-t546).*9.52624335e-4);
t6052 = t4408.*(-t2503+t2754+t3433-t3460+t3506+t4.*t871.*(t534-t546).*9.52624335e-4);
t6066 = t4408.*(t2706-t2712+t3512+t3528+t3534+t3552);
t6067 = t4408.*(t2883+t2956-t3186-t3199+t3602+t3661);
t6074 = -t4476.*(-t2503+t2754+t3433-t3460+t3506+t4.*t871.*(t534-t546).*9.52624335e-4);
t6083 = t4476.*(t2883+t2956-t3186-t3199+t3602+t3661);
t6099 = t1906+t2323+t2403+t2924+t2929+t3518+t3551+t3593+t3608;
t6117 = t1906+t2323+t2656+t2924+t2929+t3518+t3593+t3717+t3776;
t6129 = t2043+t2403+t2464+t3066+t3074+t3551+t3604+t3608+t3737;
t6555 = dphi1.*t6554;
t6557 = dphi1.*t6556;
t6626 = t1067+t1074+t1206+t1247+t1459+t1566+t2219+t2296+t2849+t2878+t3175+t3282+t3692+t3768+t4052+t4058+t4101+t4146;
t6628 = dth1.*t6627;
t1650 = -t1611;
t2086 = -t2038;
t2089 = -t2040;
t2557 = -t2501;
t2655 = -t2601;
t2659 = -t2609;
t2808 = -t2780;
t2973 = -t2939;
t3040 = Mb.*t15.*t2905;
t3190 = -t3155;
t3193 = -t3161;
t3257 = -t3219;
t3328 = -t3292;
t3329 = -t3293;
t3335 = -t3299;
t3336 = -t3302;
t3344 = -t3313;
t3402 = -t3347;
t3411 = -t3382;
t3473 = -t3404;
t3482 = -t3443;
t3540 = -t3491;
t3555 = -t3538;
t3670 = -t3634;
t3690 = -t3665;
t3738 = -t3691;
t3748 = -t3712;
t3755 = -t3719;
t3758 = -t3681;
t3766 = -t3732;
t3797 = -t3756;
t3798 = -t3757;
t3800 = dphi2.*t3774;
t3824 = -t3810;
t3825 = -t3813;
t3860 = Mt.*t4.*t10.*t3774;
t3861 = Mt.*t5.*t9.*t3774;
t3876 = dpsi1.*t3848;
t3885 = -t3865;
t3891 = Mt.*t5.*t30.*t3774;
t3892 = -t3857;
t3893 = Mt.*t5.*t34.*t3774;
t3925 = Mb.*t9.*t10.*t3848;
t3943 = Mb.*t5.*t33.*t3848;
t3945 = Mb.*t5.*t38.*t3848;
t3977 = -t3947;
t3988 = Mt.*t381.*t3774;
t3989 = Mt.*t382.*t3774;
t4006 = -t3975;
t4016 = Mt.*t420.*t3774;
t4017 = Mt.*t421.*t3774;
t4037 = -t4009;
t4044 = Mb.*t382.*t3848;
t4062 = Mb.*t420.*t3848;
t4091 = B_cg_H.*Mb.*t11.*t542.*t3848;
t4107 = B_cg_H.*Mb.*t721.*t3848;
t4148 = -t4138;
t4154 = -t4139;
t4170 = B_cg_H.*Mb.*t925.*t3848;
t4186 = -B_cg_H.*Mb.*t3848.*(t214-t541);
t4195 = -t4178;
t4200 = -t4184;
t4202 = B_cg_H.*Mb.*t1047.*t3848;
t4205 = B_cg_H.*Mb.*t3848.*(t214-t541);
t4208 = -t4199;
t4209 = -t4192;
t4238 = B_cg_H.*Mb.*t1178.*t3848;
t4243 = Mt.*t1381.*t3774;
t4260 = -t4244;
t4265 = -t4258;
t4266 = -t4259;
t4271 = -t4267;
t4285 = Mb.*t1487.*t3848;
t4303 = Mt.*t1727.*t3774;
t4310 = t1146+t2040+t2177;
t4321 = Mb.*t1676.*t3848;
t4340 = -t4336;
t4347 = -t4341;
t4350 = t1410+t2132+t2162;
t4359 = -t4353;
t4362 = dpsi1.*t4357;
t4370 = -Mt.*t3774.*(t433-t828+T_cg_H.*(t197-t537));
t4377 = Mt.*t9.*t10.*t4357;
t4379 = Mt.*t2325.*t3774;
t4380 = -t4366;
t4383 = t1263+t2380+t2450;
t4384 = -t4373;
t4385 = Mt.*t5.*t33.*t4357;
t4386 = Mt.*t5.*t38.*t4357;
t4387 = -t4374;
t4388 = -t4376;
t4389 = -t4378;
t4394 = -Mt.*t3774.*(t431+t909+T_cg_H.*(t195-t634));
t4400 = Mt.*t3774.*(t431+t909+T_cg_H.*(t195-t634));
t4404 = t4281.*(-3.36554e-3);
t4407 = t4281.*3.36554e-3;
t4409 = t3234+t3288;
t4411 = Mt.*t382.*t4357;
t4412 = Mt.*t2763.*t3774;
t4419 = Mt.*t420.*t4357;
t4429 = Mb.*t2627.*t3848;
t4439 = Mt.*t2915.*t3774;
t4451 = Mt.*t3774.*(-t120+t425+t519-t651+t765);
t4459 = t1689+t2506+t2651;
t4460 = Mb.*t3082.*t3848;
t4462 = t4352.*3.36554e-3;
t4473 = -t4465;
t4484 = t11.*t381.*t4435;
t4498 = t487.*t4435;
t4499 = -t4485;
t4504 = t4374.*3.36554e-3;
t4507 = -t4493;
t4511 = -t4501;
t4520 = -t4415.*(t105-t465);
t4524 = -t4519;
t4530 = -t4415.*(t197-t537);
t4531 = t903.*t4435;
t4534 = -t4435.*(t103-t544);
t4536 = t1044.*t4415;
t4537 = -t4532;
t4541 = Mt.*t1528.*t4357;
t4547 = dth2.*t4539;
t4548 = dx.*t4539;
t4556 = t1240.*t4415;
t4559 = Mt.*t1734.*t4357;
t4560 = -t4557;
t4562 = Mt.*t3774.*t3937;
t4567 = Mt.*t3774.*t3971;
t4570 = -t4564;
t4572 = t1430.*t4415;
t4577 = t1512.*t4415;
t4578 = t1688+t3198+t3227;
t4580 = -t4576;
t4584 = t4480.*3.36554e-3;
t4585 = t4483.*3.36554e-3;
t4587 = t4485.*3.36554e-3;
t4588 = t1505.*t4435;
t4600 = t4589./2.0;
t4601 = Mt.*t2174.*t4357;
t4605 = t4519.*3.36554e-3;
t4606 = t4415.*(t105-t465).*(-3.36554e-3);
t4608 = -Mt.*t4357.*(t451-t831+T_cg_H.*(t214-t541));
t4614 = -t4604;
t4619 = Mt.*t4357.*(t451-t831+T_cg_H.*(t214-t541));
C = ft_10({B_cg_H,ITail,Mb,Mm,Mt,T_cg_H,dphi1,dphi2,dpsi1,dth1,dth2,dx,dy,dz,t10,t1003,t1005,t1006,t1007,t1008,t1009,t1013,t1014,t1015,t1016,t1017,t1018,t1019,t1020,t1023,t1029,t103,t1037,t1047,t105,t1050,t1053,t1059,t1060,t1064,t1068,t1071,t1072,t1073,t1075,t1076,t1077,t1078,t1079,t1082,t1084,t1086,t1088,t1097,t1099,t11,t1102,t1108,t1113,t1115,t1116,t1117,t1121,t1122,t1124,t1129,t1132,t1133,t1134,t1135,t1136,t1137,t1138,t1139,t1140,t1141,t1142,t1143,t1147,t1149,t1153,t1155,t1156,t1157,t1159,t1160,t1161,t1162,t1163,t1164,t1167,t1169,t1170,t1173,t1174,t1176,t1178,t1179,t1181,t1183,t1185,t1186,t1187,t1188,t1189,t1191,t1192,t1193,t1194,t1195,t1196,t120,t1200,t1201,t1203,t1205,t1206,t1211,t1212,t1213,t1214,t1215,t1220,t1221,t1223,t1224,t1225,t1228,t1229,t1230,t1234,t1240,t1242,t1243,t1244,t1245,t1246,t1247,t1248,t1250,t1251,t1252,t1253,t1255,t1260,t1261,t1262,t1264,t1265,t1268,t1271,t1280,t1283,t1291,t130,t1301,t1302,t1303,t1304,t1305,t1306,t1307,t1309,t1313,t1322,t1328,t1331,t1332,t1334,t1337,t1338,t134,t1343,t1344,t1345,t1348,t1349,t1352,t1354,t1355,t1356,t1357,t1358,t1360,t1361,t1362,t1365,t1366,t1368,t1370,t1371,t1373,t1374,t1378,t1380,t1381,t1382,t1384,t1386,t1388,t1389,t1391,t1393,t1394,t1395,t1396,t1397,t1399,t1403,t1405,t1406,t1412,t1413,t1415,t1416,t1421,t1423,t1426,t1427,t1430,t1431,t1433,t1435,t144,t1441,t1443,t1444,t1446,t1453,t1455,t1456,t1457,t1458,t1460,t1463,t1465,t1466,t1467,t1468,t1469,t1470,t1473,t1476,t1477,t1478,t1479,t1480,t1481,t1486,t1487,t1495,t15,t1505,t1506,t1508,t1510,t1512,t1513,t1516,t1518,t1521,t1525,t1526,t1528,t1529,t1531,t1535,t1540,t1543,t1544,t1546,t1549,t1551,t1552,t1553,t1555,t1558,t1562,t1563,t1568,t1575,t1578,t1581,t1585,t1586,t1587,t1589,t1590,t1593,t1595,t1596,t1597,t1598,t1599,t1605,t1606,t1609,t161,t1610,t1612,t1614,t1617,t1618,t1619,t162,t1620,t1621,t1624,t1627,t1628,t1630,t1631,t1632,t1633,t1634,t1635,t1636,t1637,t1639,t1640,t1643,t1644,t1645,t1646,t1649,t1650,t1651,t1652,t1653,t1654,t1655,t1656,t1657,t1659,t1660,t1661,t1663,t1664,t1665,t1667,t1669,t1672,t1674,t1675,t1676,t1678,t1679,t1680,t1681,t1682,t1683,t1685,t1686,t1691,t1692,t1693,t1694,t1695,t1696,t1698,t1699,t1700,t1701,t1702,t1703,t1705,t1706,t1711,t1716,t1718,t1719,t1720,t1721,t1722,t1723,t1725,t1727,t1730,t1731,t1734,t1735,t1736,t1737,t1739,t1740,t1741,t1742,t1744,t1746,t1747,t1748,t1751,t1752,t1753,t1759,t1761,t1762,t1763,t1764,t1765,t1770,t1771,t1774,t1777,t1778,t1779,t1780,t1781,t1782,t1783,t1784,t1785,t1786,t1787,t1788,t1789,t1790,t1792,t1798,t1799,t1800,t1801,t1802,t1806,t1809,t1810,t1813,t1820,t1821,t1823,t1828,t1829,t1832,t1836,t1840,t1841,t1843,t1844,t1845,t1846,t1847,t1849,t1851,t1852,t1853,t1855,t1857,t1858,t1859,t1860,t1863,t1864,t1865,t1866,t1867,t1869,t1870,t1872,t1874,t1875,t1878,t1882,t1883,t1884,t1888,t1890,t1893,t1895,t1896,t1898,t1899,t1900,t1902,t1904,t1905,t1907,t1908,t1909,t1910,t1912,t1914,t1915,t1916,t1917,t1918,t1922,t1924,t1928,t1929,t1930,t1931,t1932,t1938,t1939,t1940,t1941,t1942,t1943,t1945,t1946,t1947,t1948,t1949,t195,t1950,t1951,t1952,t1956,t1957,t1959,t1960,t1961,t1962,t1963,t1964,t1965,t1966,t1967,t1969,t197,t1970,t1971,t1973,t1974,t1975,t1976,t1977,t1979,t1981,t1982,t1983,t1986,t1993,t1997,t1998,t1999,t2,t2000,t2002,t2003,t2004,t2005,t2007,t2008,t2009,t2010,t2011,t2012,t2013,t2015,t2016,t2017,t2018,t2020,t2023,t2024,t2025,t2026,t2032,t2033,t2037,t2038,t2042,t2045,t2046,t2047,t2048,t2049,t2050,t2057,t2058,t2059,t2061,t2062,t2064,t2065,t2066,t2067,t2068,t2069,t2072,t2073,t2074,t2075,t2076,t2079,t2081,t2082,t2083,t2086,t2087,t2088,t2089,t2090,t2091,t2093,t2094,t2095,t2096,t2102,t2104,t2106,t2107,t2108,t2109,t2110,t2111,t2113,t2117,t2118,t2119,t2123,t2127,t2128,t2130,t2131,t2134,t2135,t2137,t2138,t2139,t214,t2141,t2143,t2144,t2147,t2148,t2150,t2151,t2152,t2153,t2154,t2155,t2156,t2157,t2158,t2161,t2165,t2171,t2172,t2173,t2174,t2175,t2176,t2178,t2179,t2181,t2182,t2183,t2186,t2188,t2189,t2190,t2191,t2192,t2195,t2196,t2197,t2198,t2200,t2201,t2202,t2203,t2205,t2206,t2208,t2210,t2211,t2212,t2213,t2214,t2215,t2216,t2217,t2218,t2220,t2221,t2222,t2223,t2224,t2225,t2227,t2229,t2230,t2234,t2235,t2237,t2240,t2241,t2242,t2243,t2244,t2245,t2246,t2247,t2248,t2249,t2250,t2251,t2252,t2253,t2254,t2255,t2257,t2258,t2259,t2260,t2262,t2263,t2268,t2269,t2271,t2274,t2276,t2277,t2279,t2281,t2282,t2284,t2285,t2286,t2287,t2288,t2289,t2290,t2293,t2294,t2298,t2299,t2305,t2307,t2308,t2312,t2316,t2317,t2318,t2319,t2320,t2321,t2322,t2324,t2325,t2329,t2332,t2334,t2335,t2336,t2338,t2339,t2340,t2341,t2342,t2343,t2345,t2346,t2347,t2348,t2349,t2350,t2351,t2352,t2354,t2356,t2358,t2360,t2361,t2362,t2363,t2364,t2368,t2376,t2382,t2385,t2386,t2387,t2388,t2389,t2390,t2391,t2392,t2397,t2399,t24,t2400,t2401,t2404,t2406,t2407,t2408,t2409,t2410,t2411,t2412,t2413,t2416,t2419,t2420,t2422,t2425,t2426,t2427,t2428,t2429,t2430,t2431,t2433,t2434,t2435,t2436,t2437,t2438,t2439,t2445,t2447,t2449,t2451,t2453,t2458,t2460,t2461,t2462,t2463,t2465,t2467,t2468,t2470,t2471,t2472,t2474,t2476,t2479,t2480,t2483,t2485,t2486,t2487,t2488,t2489,t2492,t2495,t2496,t25,t2501,t2502,t2503,t2504,t2512,t2513,t2514,t2515,t2516,t2518,t2519,t2521,t2522,t2523,t2524,t2525,t2526,t2527,t2528,t2529,t2530,t2531,t2533,t2534,t2535,t2536,t2543,t2544,t2545,t2546,t2547,t2549,t2550,t2551,t2552,t2554,t2555,t2557,t2558,t2559,t2560,t2561,t2562,t2563,t2564,t2565,t2566,t2567,t2568,t2569,t2570,t2571,t2573,t2574,t2576,t2577,t2578,t2579,t2581,t2582,t2584,t2585,t2587,t2588,t2589,t259,t2590,t2591,t2597,t2598,t2599,t26,t260,t2600,t2605,t2607,t2610,t2613,t2615,t2616,t2617,t2619,t2620,t2621,t2623,t2624,t2627,t2629,t2630,t2632,t2634,t2635,t2636,t2637,t2638,t2639,t2640,t2641,t2646,t2648,t2650,t2652,t2655,t2657,t2659,t2660,t2661,t2662,t2663,t2665,t2666,t2667,t2668,t2669,t2671,t2673,t2676,t2677,t2678,t2679,t2682,t2684,t2688,t2689,t2692,t2696,t2698,t2699,t27,t2700,t2705,t2706,t2707,t2708,t2710,t2712,t2714,t2715,t2717,t2718,t2722,t2723,t2725,t2726,t2727,t2728,t2730,t2733,t2734,t2735,t2736,t2737,t2738,t2740,t2741,t2742,t2743,t2744,t2746,t2749,t2750,t2751,t2752,t2754,t2756,t2758,t2759,t276,t2760,t2761,t2763,t2764,t2765,t2766,t2767,t2768,t2769,t277,t2772,t2774,t2775,t2776,t2778,t2779,t2781,t2782,t2783,t2785,t2786,t2787,t2788,t2790,t2791,t2792,t2794,t2796,t2797,t2798,t2799,t2800,t2802,t2803,t2804,t2805,t2806,t2807,t2808,t2811,t2813,t2814,t2816,t2817,t2818,t2819,t2821,t2823,t2824,t2825,t2828,t2829,t283,t2831,t2832,t2833,t2834,t2835,t2836,t2837,t2838,t2839,t284,t2841,t2842,t2843,t2844,t2845,t2846,t2847,t2848,t2849,t285,t2853,t2857,t2858,t2859,t286,t2860,t2861,t2864,t2865,t2867,t2868,t287,t2870,t2871,t2872,t2874,t2875,t2876,t2877,t2878,t2879,t288,t2880,t2882,t2883,t2884,t2886,t2887,t2889,t289,t2890,t2892,t2893,t2896,t2897,t2898,t2899,t290,t2902,t2903,t2905,t2909,t291,t2912,t2913,t2914,t2915,t2916,t2917,t2918,t2919,t292,t2920,t2921,t2926,t2927,t2928,t293,t2930,t2932,t2936,t2937,t2938,t294,t2940,t2941,t2942,t2943,t2944,t2945,t2946,t2949,t2950,t2952,t2954,t2956,t2957,t2959,t2960,t2961,t2962,t2963,t2964,t2965,t2966,t2970,t2971,t2972,t2973,t2976,t2977,t2978,t2979,t2981,t2982,t2985,t2988,t2989,t2992,t2994,t2995,t2996,t2997,t2998,t3,t3000,t3003,t3004,t3006,t3007,t3008,t3009,t3011,t3012,t3016,t3017,t3019,t3022,t3027,t3030,t3031,t3032,t3033,t3034,t3035,t3037,t3038,t304,t3040,t3041,t3042,t3043,t3047,t3049,t3050,t3051,t3054,t3059,t3060,t3061,t3062,t3063,t3064,t3065,t3069,t3070,t3075,t3076,t3078,t3080,t3082,t3083,t3084,t3085,t3086,t3087,t3089,t3090,t3091,t3092,t3093,t3094,t3096,t3097,t3098,t3099,t3100,t3102,t3103,t3104,t3105,t3106,t3107,t3108,t3109,t3110,t3112,t3113,t3115,t3117,t3121,t3122,t3127,t3128,t3131,t3132,t3134,t3135,t3136,t3138,t3139,t3145,t3146,t3147,t3149,t3151,t3153,t3155,t3156,t3157,t3158,t3160,t3161,t3162,t3163,t3164,t3166,t3167,t3168,t3169,t3170,t3171,t3173,t3174,t3176,t3177,t3178,t3179,t3180,t3181,t3183,t3184,t3185,t3186,t3187,t3189,t3190,t3192,t3193,t3196,t3199,t3200,t3203,t3204,t3206,t3207,t3210,t3212,t3213,t3214,t3215,t3216,t3217,t3218,t3221,t3222,t3223,t3224,t3226,t3230,t3231,t3232,t3233,t3235,t3236,t3239,t3240,t3241,t3243,t3244,t3245,t3247,t3248,t3250,t3251,t3252,t3254,t3256,t3257,t3258,t3260,t3261,t3262,t3263,t3265,t3266,t3267,t3270,t3271,t3272,t3273,t3276,t3277,t3278,t3279,t3280,t3284,t3285,t3286,t3287,t3289,t3290,t3296,t3299,t3300,t3301,t3302,t3303,t3304,t3305,t3306,t3307,t3308,t3311,t3312,t3313,t3314,t3315,t3316,t3317,t3319,t3320,t3321,t3322,t3323,t3324,t3325,t3326,t3327,t3328,t3329,t3330,t3331,t3332,t3333,t3334,t3335,t3336,t3337,t3338,t3339,t3340,t3341,t3342,t3343,t3344,t3347,t3349,t3351,t3352,t3354,t3355,t3357,t3359,t3360,t3361,t3367,t3368,t3370,t3372,t3373,t3375,t3376,t3377,t3378,t3379,t3380,t3381,t3384,t3385,t3386,t3387,t3388,t3390,t3391,t3392,t3393,t3396,t3397,t3399,t3401,t3402,t3403,t3404,t3405,t3406,t3407,t3408,t3409,t3410,t3411,t3412,t3413,t3414,t3415,t3416,t3419,t3420,t3423,t3424,t3425,t3426,t3427,t3429,t3430,t3431,t3432,t3433,t3434,t3437,t3438,t3439,t3440,t3441,t3442,t3443,t3444,t3445,t3446,t3447,t3448,t3449,t3454,t3455,t3456,t3457,t3458,t3459,t3460,t3463,t3464,t3465,t3466,t3467,t3469,t3470,t3471,t3472,t3473,t3474,t3475,t3476,t3477,t3478,t3479,t3480,t3481,t3482,t3483,t3484,t3485,t3486,t3487,t3488,t3489,t3490,t3491,t3492,t3494,t3495,t3496,t3497,t3499,t3500,t3501,t3502,t3504,t3506,t3508,t3509,t3510,t3511,t3512,t3513,t3515,t3516,t3517,t3521,t3522,t3523,t3524,t3526,t3528,t3529,t3530,t3531,t3532,t3533,t3534,t3535,t3536,t3537,t3538,t3539,t3540,t3541,t3542,t3543,t3544,t3545,t3547,t3548,t3550,t3552,t3553,t3554,t3555,t3556,t3557,t3558,t3559,t3562,t3563,t3565,t3570,t3571,t3575,t3576,t3578,t3579,t3581,t3582,t3583,t3584,t3587,t3588,t3591,t3594,t3595,t3596,t3597,t3598,t3600,t3601,t3602,t3603,t3605,t3609,t3610,t3611,t3613,t3614,t3615,t3616,t3617,t3618,t3619,t3620,t3621,t3622,t3623,t3624,t3625,t3626,t3627,t3629,t3630,t3632,t3634,t3635,t3637,t3638,t3639,t3643,t3644,t3646,t3647,t3648,t3649,t3651,t3652,t3653,t3654,t3655,t3657,t3658,t3659,t3660,t3661,t3664,t3666,t3667,t3668,t3670,t3671,t3672,t3673,t3674,t3675,t3676,t3677,t3678,t3679,t3680,t3681,t3682,t3683,t3684,t3685,t3686,t3687,t3689,t3690,t3693,t3697,t3698,t3699,t3700,t3701,t3702,t3704,t3708,t3709,t3710,t3711,t3716,t3719,t3720,t3721,t3722,t3723,t3724,t3730,t3735,t3736,t3738,t3739,t3741,t3742,t3744,t3745,t3746,t3747,t3748,t3749,t3750,t3751,t3752,t3755,t3756,t3757,t3758,t3759,t376,t3760,t3761,t3762,t3763,t3764,t3765,t3766,t3767,t3769,t377,t3770,t3771,t3772,t3773,t3774,t3775,t3777,t3779,t3780,t3784,t3785,t3787,t3789,t3790,t3791,t3792,t3793,t3794,t3795,t3797,t3798,t3799,t3800,t3802,t3804,t3805,t3806,t3807,t3808,t3809,t381,t3811,t3812,t3814,t3815,t3817,t3818,t3819,t382,t3820,t3823,t3824,t3825,t3826,t3828,t3829,t383,t3831,t3832,t3833,t3834,t3836,t3837,t3838,t3840,t3841,t3842,t3844,t3845,t3846,t3847,t3848,t3849,t3850,t3851,t3854,t3855,t3856,t3858,t3859,t3860,t3861,t3862,t3866,t3867,t3868,t3870,t3871,t3872,t3873,t3876,t3879,t3880,t3882,t3883,t3884,t3885,t3886,t3887,t3888,t3889,t3890,t3891,t3892,t3893,t3894,t3896,t3897,t3898,t390,t3900,t3901,t3902,t3903,t3906,t3907,t3908,t3909,t3910,t3911,t3913,t3914,t3915,t3916,t3918,t3919,t3921,t3923,t3925,t3926,t3928,t3929,t3930,t3931,t3932,t3933,t3934,t3935,t3936,t3937,t3938,t3939,t394,t3940,t3941,t3943,t3944,t3945,t3946,t3947,t3948,t3949,t3950,t3951,t3952,t3953,t3954,t3955,t3956,t3957,t3958,t3959,t3960,t3961,t3962,t3964,t3965,t3966,t3967,t3969,t3970,t3971,t3974,t3975,t3976,t3977,t3978,t3979,t3980,t3981,t3982,t3983,t3984,t3985,t3986,t3987,t3988,t3989,t3991,t3992,t3993,t3994,t3995,t3996,t3997,t3998,t4,t4000,t4001,t4003,t4005,t4006,t4007,t4008,t4009,t4010,t4011,t4012,t4013,t4014,t4015,t4016,t4017,t4019,t4020,t4021,t4022,t4023,t4024,t4025,t4026,t4027,t4028,t4029,t4030,t4031,t4032,t4033,t4034,t4035,t4036,t4037,t4038,t4040,t4041,t4042,t4043,t4044,t4046,t4047,t4048,t4050,t4051,t4052,t4053,t4054,t4056,t4058,t4059,t4061,t4062,t4064,t4065,t4066,t4068,t4070,t4071,t4072,t4073,t4074,t4077,t4078,t4081,t4083,t4084,t4085,t4086,t4087,t4089,t4090,t4091,t4092,t4093,t4094,t4095,t4096,t4097,t4098,t4099,t410,t4100,t4104,t4105,t4107,t4108,t4109,t411,t4111,t4112,t4115,t4116,t4117,t4119,t412,t4120,t4121,t4122,t4126,t4128,t4129,t413,t4130,t4131,t4132,t4133,t4135,t4137,t4138,t4139,t414,t4140,t4141,t4143,t4144,t4145,t4147,t4148,t415,t4151,t4152,t4153,t4154,t4155,t4156,t4157,t4158,t4160,t4162,t4164,t4165,t4166,t4168,t4169,t4170,t4171,t4173,t4174,t4176,t4177,t4178,t4179,t4182,t4184,t4186,t4187,t4188,t4189,t4190,t4191,t4192,t4193,t4194,t4195,t4196,t4197,t420,t4200,t4201,t4202,t4203,t4204,t4205,t4206,t4208,t4209,t421,t4210,t4211,t4212,t4213,t4214,t4215,t4216,t4217,t4218,t4220,t4221,t4222,t4223,t4224,t4225,t4226,t4227,t4228,t4229,t4230,t4231,t4232,t4233,t4234,t4236,t4237,t4238,t4239,t4240,t4241,t4243,t4244,t4245,t4246,t4247,t4248,t4249,t425,t4250,t4252,t4253,t4255,t4256,t4258,t4259,t4260,t4261,t4262,t4263,t4265,t4266,t4268,t4269,t4271,t4272,t4273,t4274,t4276,t4277,t4278,t4280,t4281,t4282,t4285,t4286,t4290,t4295,t4296,t4298,t430,t4300,t4301,t4302,t4303,t4304,t4305,t4306,t4307,t4308,t4309,t431,t4310,t4311,t4312,t4313,t4315,t4316,t4317,t4318,t4319,t4320,t4321,t4322,t4323,t4324,t4326,t4327,t4329,t433,t4330,t4332,t4333,t4334,t4337,t4339,t4340,t4341,t4342,t4343,t4344,t4345,t4346,t4347,t4348,t4349,t4350,t4351,t4352,t4354,t4355,t4356,t4357,t4358,t4359,t436,t4360,t4361,t4362,t4364,t4365,t4367,t4368,t4370,t4371,t4372,t4373,t4374,t4375,t4376,t4377,t4378,t4379,t4380,t4382,t4383,t4384,t4385,t4386,t4387,t4388,t4389,t4392,t4393,t4394,t4395,t4396,t4399,t44,t4400,t4401,t4402,t4403,t4404,t4405,t4406,t4407,t4408,t4409,t4411,t4412,t4413,t4414,t4415,t4416,t4418,t4419,t4420,t4421,t4422,t4424,t4425,t4426,t4427,t4428,t4429,t4431,t4432,t4433,t4434,t4435,t4437,t4438,t4439,t4440,t4442,t4444,t4447,t4449,t445,t4450,t4451,t4452,t4453,t4454,t4455,t4457,t4458,t4459,t4460,t4461,t4462,t4465,t4467,t4469,t4470,t4471,t4472,t4473,t4475,t4476,t4477,t4478,t4479,t4480,t4481,t4482,t4483,t4484,t4485,t4486,t4487,t4488,t4489,t4490,t4492,t4493,t4494,t4495,t4496,t4497,t4498,t4499,t4500,t4501,t4502,t4503,t4504,t4505,t4506,t4507,t451,t4511,t4512,t4514,t4515,t4517,t4518,t4519,t4520,t4521,t4522,t4523,t4524,t4525,t4526,t4528,t4529,t4530,t4531,t4532,t4533,t4534,t4536,t4537,t4538,t4541,t4542,t4545,t4546,t4547,t4548,t4549,t4550,t4551,t4552,t4553,t4555,t4556,t4557,t4558,t4559,t4560,t4561,t4562,t4563,t4566,t4567,t4569,t4570,t4571,t4572,t4573,t4574,t4575,t4576,t4577,t4578,t4580,t4581,t4583,t4584,t4585,t4587,t4588,t4589,t459,t4591,t4592,t4597,t4598,t4600,t4601,t4602,t4603,t4604,t4605,t4606,t4608,t4610,t4613,t4614,t4615,t4616,t4617,t4618,t4619,t4621,t4622,t4625,t4630,t4636,t4637,t4638,t4641,t4645,t4646,t4649,t465,t4651,t4655,t4659,t4660,t4661,t4662,t4663,t4664,t4665,t4668,t4669,t4671,t4672,t4676,t4677,t4686,t4695,t4701,t4707,t4708,t4709,t4711,t4713,t4722,t4723,t4724,t4725,t4732,t4733,t4735,t4736,t4737,t4738,t4740,t4746,t4747,t4748,t4751,t4752,t4756,t4758,t4766,t4770,t4771,t4772,t4775,t4776,t4778,t4782,t4784,t4787,t4789,t4796,t48,t4800,t4801,t4802,t4805,t4807,t4809,t4821,t4823,t4830,t4834,t4837,t4842,t4846,t4847,t4848,t4849,t485,t4859,t4862,t4864,t4870,t4871,t4873,t4874,t4877,t4878,t488,t4880,t4882,t4883,t4889,t4890,t4892,t4895,t4897,t49,t4904,t4908,t4909,t491,t4912,t4913,t4922,t4923,t4925,t4927,t4931,t4932,t4933,t4934,t4936,t4938,t4939,t4941,t4942,t4944,t4945,t4946,t4949,t4950,t4953,t4954,t496,t4960,t4961,t4964,t4966,t4967,t4968,t4969,t4975,t4976,t4978,t4979,t4986,t4987,t4988,t4990,t4991,t4992,t4993,t4995,t4997,t4998,t5,t50,t5004,t501,t5017,t502,t5020,t5021,t5024,t5029,t5030,t5031,t5032,t5033,t5036,t5038,t504,t5041,t5042,t5046,t5048,t5051,t5053,t5054,t5055,t5058,t5059,t5061,t5063,t5066,t5067,t5072,t5074,t5076,t5078,t5080,t5082,t5083,t5088,t5092,t5098,t5099,t51,t5103,t5109,t5114,t5126,t5128,t5131,t5143,t5150,t5152,t5153,t5156,t5161,t5165,t5177,t5179,t5184,t519,t5191,t5194,t5197,t5198,t5202,t5203,t5205,t5206,t5207,t5208,t5214,t5223,t5227,t523,t5232,t524,t5240,t5241,t5265,t527,t5275,t5287,t5291,t5293,t530,t5300,t5308,t5310,t5317,t5319,t5324,t5328,t534,t5344,t5351,t5354,t5358,t5363,t537,t5372,t5374,t5379,t5380,t539,t5399,t54,t541,t5412,t5417,t542,t5420,t5424,t5427,t5431,t5438,t544,t5445,t5448,t5452,t5453,t5456,t546,t5460,t5476,t5488,t5490,t5492,t5493,t5494,t5498,t55,t550,t5523,t5524,t553,t5530,t5538,t5539,t5547,t5548,t5552,t5556,t5565,t5566,t5569,t557,t5576,t558,t5582,t5588,t5598,t56,t5607,t5620,t5657,t5660,t5662,t5664,t5668,t5672,t5674,t5685,t5690,t5696,t5697,t5705,t5706,t5713,t5724,t573,t5730,t5738,t574,t5749,t575,t5757,t5779,t5785,t5788,t5791,t5795,t5798,t5800,t5806,t5808,t5809,t5815,t5832,t5837,t5840,t5843,t5846,t5857,t5867,t5869,t587,t5870,t5874,t5880,t5887,t59,t5905,t5926,t5932,t5933,t5936,t5939,t5949,t595,t5963,t5971,t5984,t5985,t603,t6049,t6051,t6052,t6066,t6067,t6074,t6083,t6099,t61,t6117,t6129,t614,t628,t629,t634,t641,t65,t650,t651,t655,t6555,t6557,t657,t6599,t6628,t6629,t664,t665,t666,t667,t668,t669,t675,t68,t693,t7,t71,t721,t724,t73,t731,t732,t736,t741,t753,t754,t755,t756,t757,t759,t760,t761,t762,t764,t765,t769,t772,t774,t776,t778,t795,t797,t799,t8,t802,t803,t806,t817,t818,t820,t824,t828,t831,t838,t843,t844,t846,t847,t848,t850,t851,t852,t853,t855,t865,t867,t868,t870,t871,t872,t876,t877,t886,t888,t890,t896,t9,t901,t902,t903,t904,t906,t907,t909,t914,t916,t924,t925,t926,t947,t949,t952,t954,t955,t957,t964,t972,t977,t983,t987,t991,t992,t993,t994,t995});
end
function C = ft_10(ct)
B_cg_H = ct{1};
ITail = ct{2};
Mb = ct{3};
Mm = ct{4};
Mt = ct{5};
T_cg_H = ct{6};
dphi1 = ct{7};
dphi2 = ct{8};
dpsi1 = ct{9};
dth1 = ct{10};
dth2 = ct{11};
dx = ct{12};
dy = ct{13};
dz = ct{14};
t10 = ct{15};
t1003 = ct{16};
t1005 = ct{17};
t1006 = ct{18};
t1007 = ct{19};
t1008 = ct{20};
t1009 = ct{21};
t1013 = ct{22};
t1014 = ct{23};
t1015 = ct{24};
t1016 = ct{25};
t1017 = ct{26};
t1018 = ct{27};
t1019 = ct{28};
t1020 = ct{29};
t1023 = ct{30};
t1029 = ct{31};
t103 = ct{32};
t1037 = ct{33};
t1047 = ct{34};
t105 = ct{35};
t1050 = ct{36};
t1053 = ct{37};
t1059 = ct{38};
t1060 = ct{39};
t1064 = ct{40};
t1068 = ct{41};
t1071 = ct{42};
t1072 = ct{43};
t1073 = ct{44};
t1075 = ct{45};
t1076 = ct{46};
t1077 = ct{47};
t1078 = ct{48};
t1079 = ct{49};
t1082 = ct{50};
t1084 = ct{51};
t1086 = ct{52};
t1088 = ct{53};
t1097 = ct{54};
t1099 = ct{55};
t11 = ct{56};
t1102 = ct{57};
t1108 = ct{58};
t1113 = ct{59};
t1115 = ct{60};
t1116 = ct{61};
t1117 = ct{62};
t1121 = ct{63};
t1122 = ct{64};
t1124 = ct{65};
t1129 = ct{66};
t1132 = ct{67};
t1133 = ct{68};
t1134 = ct{69};
t1135 = ct{70};
t1136 = ct{71};
t1137 = ct{72};
t1138 = ct{73};
t1139 = ct{74};
t1140 = ct{75};
t1141 = ct{76};
t1142 = ct{77};
t1143 = ct{78};
t1147 = ct{79};
t1149 = ct{80};
t1153 = ct{81};
t1155 = ct{82};
t1156 = ct{83};
t1157 = ct{84};
t1159 = ct{85};
t1160 = ct{86};
t1161 = ct{87};
t1162 = ct{88};
t1163 = ct{89};
t1164 = ct{90};
t1167 = ct{91};
t1169 = ct{92};
t1170 = ct{93};
t1173 = ct{94};
t1174 = ct{95};
t1176 = ct{96};
t1178 = ct{97};
t1179 = ct{98};
t1181 = ct{99};
t1183 = ct{100};
t1185 = ct{101};
t1186 = ct{102};
t1187 = ct{103};
t1188 = ct{104};
t1189 = ct{105};
t1191 = ct{106};
t1192 = ct{107};
t1193 = ct{108};
t1194 = ct{109};
t1195 = ct{110};
t1196 = ct{111};
t120 = ct{112};
t1200 = ct{113};
t1201 = ct{114};
t1203 = ct{115};
t1205 = ct{116};
t1206 = ct{117};
t1211 = ct{118};
t1212 = ct{119};
t1213 = ct{120};
t1214 = ct{121};
t1215 = ct{122};
t1220 = ct{123};
t1221 = ct{124};
t1223 = ct{125};
t1224 = ct{126};
t1225 = ct{127};
t1228 = ct{128};
t1229 = ct{129};
t1230 = ct{130};
t1234 = ct{131};
t1240 = ct{132};
t1242 = ct{133};
t1243 = ct{134};
t1244 = ct{135};
t1245 = ct{136};
t1246 = ct{137};
t1247 = ct{138};
t1248 = ct{139};
t1250 = ct{140};
t1251 = ct{141};
t1252 = ct{142};
t1253 = ct{143};
t1255 = ct{144};
t1260 = ct{145};
t1261 = ct{146};
t1262 = ct{147};
t1264 = ct{148};
t1265 = ct{149};
t1268 = ct{150};
t1271 = ct{151};
t1280 = ct{152};
t1283 = ct{153};
t1291 = ct{154};
t130 = ct{155};
t1301 = ct{156};
t1302 = ct{157};
t1303 = ct{158};
t1304 = ct{159};
t1305 = ct{160};
t1306 = ct{161};
t1307 = ct{162};
t1309 = ct{163};
t1313 = ct{164};
t1322 = ct{165};
t1328 = ct{166};
t1331 = ct{167};
t1332 = ct{168};
t1334 = ct{169};
t1337 = ct{170};
t1338 = ct{171};
t134 = ct{172};
t1343 = ct{173};
t1344 = ct{174};
t1345 = ct{175};
t1348 = ct{176};
t1349 = ct{177};
t1352 = ct{178};
t1354 = ct{179};
t1355 = ct{180};
t1356 = ct{181};
t1357 = ct{182};
t1358 = ct{183};
t1360 = ct{184};
t1361 = ct{185};
t1362 = ct{186};
t1365 = ct{187};
t1366 = ct{188};
t1368 = ct{189};
t1370 = ct{190};
t1371 = ct{191};
t1373 = ct{192};
t1374 = ct{193};
t1378 = ct{194};
t1380 = ct{195};
t1381 = ct{196};
t1382 = ct{197};
t1384 = ct{198};
t1386 = ct{199};
t1388 = ct{200};
t1389 = ct{201};
t1391 = ct{202};
t1393 = ct{203};
t1394 = ct{204};
t1395 = ct{205};
t1396 = ct{206};
t1397 = ct{207};
t1399 = ct{208};
t1403 = ct{209};
t1405 = ct{210};
t1406 = ct{211};
t1412 = ct{212};
t1413 = ct{213};
t1415 = ct{214};
t1416 = ct{215};
t1421 = ct{216};
t1423 = ct{217};
t1426 = ct{218};
t1427 = ct{219};
t1430 = ct{220};
t1431 = ct{221};
t1433 = ct{222};
t1435 = ct{223};
t144 = ct{224};
t1441 = ct{225};
t1443 = ct{226};
t1444 = ct{227};
t1446 = ct{228};
t1453 = ct{229};
t1455 = ct{230};
t1456 = ct{231};
t1457 = ct{232};
t1458 = ct{233};
t1460 = ct{234};
t1463 = ct{235};
t1465 = ct{236};
t1466 = ct{237};
t1467 = ct{238};
t1468 = ct{239};
t1469 = ct{240};
t1470 = ct{241};
t1473 = ct{242};
t1476 = ct{243};
t1477 = ct{244};
t1478 = ct{245};
t1479 = ct{246};
t1480 = ct{247};
t1481 = ct{248};
t1486 = ct{249};
t1487 = ct{250};
t1495 = ct{251};
t15 = ct{252};
t1505 = ct{253};
t1506 = ct{254};
t1508 = ct{255};
t1510 = ct{256};
t1512 = ct{257};
t1513 = ct{258};
t1516 = ct{259};
t1518 = ct{260};
t1521 = ct{261};
t1525 = ct{262};
t1526 = ct{263};
t1528 = ct{264};
t1529 = ct{265};
t1531 = ct{266};
t1535 = ct{267};
t1540 = ct{268};
t1543 = ct{269};
t1544 = ct{270};
t1546 = ct{271};
t1549 = ct{272};
t1551 = ct{273};
t1552 = ct{274};
t1553 = ct{275};
t1555 = ct{276};
t1558 = ct{277};
t1562 = ct{278};
t1563 = ct{279};
t1568 = ct{280};
t1575 = ct{281};
t1578 = ct{282};
t1581 = ct{283};
t1585 = ct{284};
t1586 = ct{285};
t1587 = ct{286};
t1589 = ct{287};
t1590 = ct{288};
t1593 = ct{289};
t1595 = ct{290};
t1596 = ct{291};
t1597 = ct{292};
t1598 = ct{293};
t1599 = ct{294};
t1605 = ct{295};
t1606 = ct{296};
t1609 = ct{297};
t161 = ct{298};
t1610 = ct{299};
t1612 = ct{300};
t1614 = ct{301};
t1617 = ct{302};
t1618 = ct{303};
t1619 = ct{304};
t162 = ct{305};
t1620 = ct{306};
t1621 = ct{307};
t1624 = ct{308};
t1627 = ct{309};
t1628 = ct{310};
t1630 = ct{311};
t1631 = ct{312};
t1632 = ct{313};
t1633 = ct{314};
t1634 = ct{315};
t1635 = ct{316};
t1636 = ct{317};
t1637 = ct{318};
t1639 = ct{319};
t1640 = ct{320};
t1643 = ct{321};
t1644 = ct{322};
t1645 = ct{323};
t1646 = ct{324};
t1649 = ct{325};
t1650 = ct{326};
t1651 = ct{327};
t1652 = ct{328};
t1653 = ct{329};
t1654 = ct{330};
t1655 = ct{331};
t1656 = ct{332};
t1657 = ct{333};
t1659 = ct{334};
t1660 = ct{335};
t1661 = ct{336};
t1663 = ct{337};
t1664 = ct{338};
t1665 = ct{339};
t1667 = ct{340};
t1669 = ct{341};
t1672 = ct{342};
t1674 = ct{343};
t1675 = ct{344};
t1676 = ct{345};
t1678 = ct{346};
t1679 = ct{347};
t1680 = ct{348};
t1681 = ct{349};
t1682 = ct{350};
t1683 = ct{351};
t1685 = ct{352};
t1686 = ct{353};
t1691 = ct{354};
t1692 = ct{355};
t1693 = ct{356};
t1694 = ct{357};
t1695 = ct{358};
t1696 = ct{359};
t1698 = ct{360};
t1699 = ct{361};
t1700 = ct{362};
t1701 = ct{363};
t1702 = ct{364};
t1703 = ct{365};
t1705 = ct{366};
t1706 = ct{367};
t1711 = ct{368};
t1716 = ct{369};
t1718 = ct{370};
t1719 = ct{371};
t1720 = ct{372};
t1721 = ct{373};
t1722 = ct{374};
t1723 = ct{375};
t1725 = ct{376};
t1727 = ct{377};
t1730 = ct{378};
t1731 = ct{379};
t1734 = ct{380};
t1735 = ct{381};
t1736 = ct{382};
t1737 = ct{383};
t1739 = ct{384};
t1740 = ct{385};
t1741 = ct{386};
t1742 = ct{387};
t1744 = ct{388};
t1746 = ct{389};
t1747 = ct{390};
t1748 = ct{391};
t1751 = ct{392};
t1752 = ct{393};
t1753 = ct{394};
t1759 = ct{395};
t1761 = ct{396};
t1762 = ct{397};
t1763 = ct{398};
t1764 = ct{399};
t1765 = ct{400};
t1770 = ct{401};
t1771 = ct{402};
t1774 = ct{403};
t1777 = ct{404};
t1778 = ct{405};
t1779 = ct{406};
t1780 = ct{407};
t1781 = ct{408};
t1782 = ct{409};
t1783 = ct{410};
t1784 = ct{411};
t1785 = ct{412};
t1786 = ct{413};
t1787 = ct{414};
t1788 = ct{415};
t1789 = ct{416};
t1790 = ct{417};
t1792 = ct{418};
t1798 = ct{419};
t1799 = ct{420};
t1800 = ct{421};
t1801 = ct{422};
t1802 = ct{423};
t1806 = ct{424};
t1809 = ct{425};
t1810 = ct{426};
t1813 = ct{427};
t1820 = ct{428};
t1821 = ct{429};
t1823 = ct{430};
t1828 = ct{431};
t1829 = ct{432};
t1832 = ct{433};
t1836 = ct{434};
t1840 = ct{435};
t1841 = ct{436};
t1843 = ct{437};
t1844 = ct{438};
t1845 = ct{439};
t1846 = ct{440};
t1847 = ct{441};
t1849 = ct{442};
t1851 = ct{443};
t1852 = ct{444};
t1853 = ct{445};
t1855 = ct{446};
t1857 = ct{447};
t1858 = ct{448};
t1859 = ct{449};
t1860 = ct{450};
t1863 = ct{451};
t1864 = ct{452};
t1865 = ct{453};
t1866 = ct{454};
t1867 = ct{455};
t1869 = ct{456};
t1870 = ct{457};
t1872 = ct{458};
t1874 = ct{459};
t1875 = ct{460};
t1878 = ct{461};
t1882 = ct{462};
t1883 = ct{463};
t1884 = ct{464};
t1888 = ct{465};
t1890 = ct{466};
t1893 = ct{467};
t1895 = ct{468};
t1896 = ct{469};
t1898 = ct{470};
t1899 = ct{471};
t1900 = ct{472};
t1902 = ct{473};
t1904 = ct{474};
t1905 = ct{475};
t1907 = ct{476};
t1908 = ct{477};
t1909 = ct{478};
t1910 = ct{479};
t1912 = ct{480};
t1914 = ct{481};
t1915 = ct{482};
t1916 = ct{483};
t1917 = ct{484};
t1918 = ct{485};
t1922 = ct{486};
t1924 = ct{487};
t1928 = ct{488};
t1929 = ct{489};
t1930 = ct{490};
t1931 = ct{491};
t1932 = ct{492};
t1938 = ct{493};
t1939 = ct{494};
t1940 = ct{495};
t1941 = ct{496};
t1942 = ct{497};
t1943 = ct{498};
t1945 = ct{499};
t1946 = ct{500};
t1947 = ct{501};
t1948 = ct{502};
t1949 = ct{503};
t195 = ct{504};
t1950 = ct{505};
t1951 = ct{506};
t1952 = ct{507};
t1956 = ct{508};
t1957 = ct{509};
t1959 = ct{510};
t1960 = ct{511};
t1961 = ct{512};
t1962 = ct{513};
t1963 = ct{514};
t1964 = ct{515};
t1965 = ct{516};
t1966 = ct{517};
t1967 = ct{518};
t1969 = ct{519};
t197 = ct{520};
t1970 = ct{521};
t1971 = ct{522};
t1973 = ct{523};
t1974 = ct{524};
t1975 = ct{525};
t1976 = ct{526};
t1977 = ct{527};
t1979 = ct{528};
t1981 = ct{529};
t1982 = ct{530};
t1983 = ct{531};
t1986 = ct{532};
t1993 = ct{533};
t1997 = ct{534};
t1998 = ct{535};
t1999 = ct{536};
t2 = ct{537};
t2000 = ct{538};
t2002 = ct{539};
t2003 = ct{540};
t2004 = ct{541};
t2005 = ct{542};
t2007 = ct{543};
t2008 = ct{544};
t2009 = ct{545};
t2010 = ct{546};
t2011 = ct{547};
t2012 = ct{548};
t2013 = ct{549};
t2015 = ct{550};
t2016 = ct{551};
t2017 = ct{552};
t2018 = ct{553};
t2020 = ct{554};
t2023 = ct{555};
t2024 = ct{556};
t2025 = ct{557};
t2026 = ct{558};
t2032 = ct{559};
t2033 = ct{560};
t2037 = ct{561};
t2038 = ct{562};
t2042 = ct{563};
t2045 = ct{564};
t2046 = ct{565};
t2047 = ct{566};
t2048 = ct{567};
t2049 = ct{568};
t2050 = ct{569};
t2057 = ct{570};
t2058 = ct{571};
t2059 = ct{572};
t2061 = ct{573};
t2062 = ct{574};
t2064 = ct{575};
t2065 = ct{576};
t2066 = ct{577};
t2067 = ct{578};
t2068 = ct{579};
t2069 = ct{580};
t2072 = ct{581};
t2073 = ct{582};
t2074 = ct{583};
t2075 = ct{584};
t2076 = ct{585};
t2079 = ct{586};
t2081 = ct{587};
t2082 = ct{588};
t2083 = ct{589};
t2086 = ct{590};
t2087 = ct{591};
t2088 = ct{592};
t2089 = ct{593};
t2090 = ct{594};
t2091 = ct{595};
t2093 = ct{596};
t2094 = ct{597};
t2095 = ct{598};
t2096 = ct{599};
t2102 = ct{600};
t2104 = ct{601};
t2106 = ct{602};
t2107 = ct{603};
t2108 = ct{604};
t2109 = ct{605};
t2110 = ct{606};
t2111 = ct{607};
t2113 = ct{608};
t2117 = ct{609};
t2118 = ct{610};
t2119 = ct{611};
t2123 = ct{612};
t2127 = ct{613};
t2128 = ct{614};
t2130 = ct{615};
t2131 = ct{616};
t2134 = ct{617};
t2135 = ct{618};
t2137 = ct{619};
t2138 = ct{620};
t2139 = ct{621};
t214 = ct{622};
t2141 = ct{623};
t2143 = ct{624};
t2144 = ct{625};
t2147 = ct{626};
t2148 = ct{627};
t2150 = ct{628};
t2151 = ct{629};
t2152 = ct{630};
t2153 = ct{631};
t2154 = ct{632};
t2155 = ct{633};
t2156 = ct{634};
t2157 = ct{635};
t2158 = ct{636};
t2161 = ct{637};
t2165 = ct{638};
t2171 = ct{639};
t2172 = ct{640};
t2173 = ct{641};
t2174 = ct{642};
t2175 = ct{643};
t2176 = ct{644};
t2178 = ct{645};
t2179 = ct{646};
t2181 = ct{647};
t2182 = ct{648};
t2183 = ct{649};
t2186 = ct{650};
t2188 = ct{651};
t2189 = ct{652};
t2190 = ct{653};
t2191 = ct{654};
t2192 = ct{655};
t2195 = ct{656};
t2196 = ct{657};
t2197 = ct{658};
t2198 = ct{659};
t2200 = ct{660};
t2201 = ct{661};
t2202 = ct{662};
t2203 = ct{663};
t2205 = ct{664};
t2206 = ct{665};
t2208 = ct{666};
t2210 = ct{667};
t2211 = ct{668};
t2212 = ct{669};
t2213 = ct{670};
t2214 = ct{671};
t2215 = ct{672};
t2216 = ct{673};
t2217 = ct{674};
t2218 = ct{675};
t2220 = ct{676};
t2221 = ct{677};
t2222 = ct{678};
t2223 = ct{679};
t2224 = ct{680};
t2225 = ct{681};
t2227 = ct{682};
t2229 = ct{683};
t2230 = ct{684};
t2234 = ct{685};
t2235 = ct{686};
t2237 = ct{687};
t2240 = ct{688};
t2241 = ct{689};
t2242 = ct{690};
t2243 = ct{691};
t2244 = ct{692};
t2245 = ct{693};
t2246 = ct{694};
t2247 = ct{695};
t2248 = ct{696};
t2249 = ct{697};
t2250 = ct{698};
t2251 = ct{699};
t2252 = ct{700};
t2253 = ct{701};
t2254 = ct{702};
t2255 = ct{703};
t2257 = ct{704};
t2258 = ct{705};
t2259 = ct{706};
t2260 = ct{707};
t2262 = ct{708};
t2263 = ct{709};
t2268 = ct{710};
t2269 = ct{711};
t2271 = ct{712};
t2274 = ct{713};
t2276 = ct{714};
t2277 = ct{715};
t2279 = ct{716};
t2281 = ct{717};
t2282 = ct{718};
t2284 = ct{719};
t2285 = ct{720};
t2286 = ct{721};
t2287 = ct{722};
t2288 = ct{723};
t2289 = ct{724};
t2290 = ct{725};
t2293 = ct{726};
t2294 = ct{727};
t2298 = ct{728};
t2299 = ct{729};
t2305 = ct{730};
t2307 = ct{731};
t2308 = ct{732};
t2312 = ct{733};
t2316 = ct{734};
t2317 = ct{735};
t2318 = ct{736};
t2319 = ct{737};
t2320 = ct{738};
t2321 = ct{739};
t2322 = ct{740};
t2324 = ct{741};
t2325 = ct{742};
t2329 = ct{743};
t2332 = ct{744};
t2334 = ct{745};
t2335 = ct{746};
t2336 = ct{747};
t2338 = ct{748};
t2339 = ct{749};
t2340 = ct{750};
t2341 = ct{751};
t2342 = ct{752};
t2343 = ct{753};
t2345 = ct{754};
t2346 = ct{755};
t2347 = ct{756};
t2348 = ct{757};
t2349 = ct{758};
t2350 = ct{759};
t2351 = ct{760};
t2352 = ct{761};
t2354 = ct{762};
t2356 = ct{763};
t2358 = ct{764};
t2360 = ct{765};
t2361 = ct{766};
t2362 = ct{767};
t2363 = ct{768};
t2364 = ct{769};
t2368 = ct{770};
t2376 = ct{771};
t2382 = ct{772};
t2385 = ct{773};
t2386 = ct{774};
t2387 = ct{775};
t2388 = ct{776};
t2389 = ct{777};
t2390 = ct{778};
t2391 = ct{779};
t2392 = ct{780};
t2397 = ct{781};
t2399 = ct{782};
t24 = ct{783};
t2400 = ct{784};
t2401 = ct{785};
t2404 = ct{786};
t2406 = ct{787};
t2407 = ct{788};
t2408 = ct{789};
t2409 = ct{790};
t2410 = ct{791};
t2411 = ct{792};
t2412 = ct{793};
t2413 = ct{794};
t2416 = ct{795};
t2419 = ct{796};
t2420 = ct{797};
t2422 = ct{798};
t2425 = ct{799};
t2426 = ct{800};
t2427 = ct{801};
t2428 = ct{802};
t2429 = ct{803};
t2430 = ct{804};
t2431 = ct{805};
t2433 = ct{806};
t2434 = ct{807};
t2435 = ct{808};
t2436 = ct{809};
t2437 = ct{810};
t2438 = ct{811};
t2439 = ct{812};
t2445 = ct{813};
t2447 = ct{814};
t2449 = ct{815};
t2451 = ct{816};
t2453 = ct{817};
t2458 = ct{818};
t2460 = ct{819};
t2461 = ct{820};
t2462 = ct{821};
t2463 = ct{822};
t2465 = ct{823};
t2467 = ct{824};
t2468 = ct{825};
t2470 = ct{826};
t2471 = ct{827};
t2472 = ct{828};
t2474 = ct{829};
t2476 = ct{830};
t2479 = ct{831};
t2480 = ct{832};
t2483 = ct{833};
t2485 = ct{834};
t2486 = ct{835};
t2487 = ct{836};
t2488 = ct{837};
t2489 = ct{838};
t2492 = ct{839};
t2495 = ct{840};
t2496 = ct{841};
t25 = ct{842};
t2501 = ct{843};
t2502 = ct{844};
t2503 = ct{845};
t2504 = ct{846};
t2512 = ct{847};
t2513 = ct{848};
t2514 = ct{849};
t2515 = ct{850};
t2516 = ct{851};
t2518 = ct{852};
t2519 = ct{853};
t2521 = ct{854};
t2522 = ct{855};
t2523 = ct{856};
t2524 = ct{857};
t2525 = ct{858};
t2526 = ct{859};
t2527 = ct{860};
t2528 = ct{861};
t2529 = ct{862};
t2530 = ct{863};
t2531 = ct{864};
t2533 = ct{865};
t2534 = ct{866};
t2535 = ct{867};
t2536 = ct{868};
t2543 = ct{869};
t2544 = ct{870};
t2545 = ct{871};
t2546 = ct{872};
t2547 = ct{873};
t2549 = ct{874};
t2550 = ct{875};
t2551 = ct{876};
t2552 = ct{877};
t2554 = ct{878};
t2555 = ct{879};
t2557 = ct{880};
t2558 = ct{881};
t2559 = ct{882};
t2560 = ct{883};
t2561 = ct{884};
t2562 = ct{885};
t2563 = ct{886};
t2564 = ct{887};
t2565 = ct{888};
t2566 = ct{889};
t2567 = ct{890};
t2568 = ct{891};
t2569 = ct{892};
t2570 = ct{893};
t2571 = ct{894};
t2573 = ct{895};
t2574 = ct{896};
t2576 = ct{897};
t2577 = ct{898};
t2578 = ct{899};
t2579 = ct{900};
t2581 = ct{901};
t2582 = ct{902};
t2584 = ct{903};
t2585 = ct{904};
t2587 = ct{905};
t2588 = ct{906};
t2589 = ct{907};
t259 = ct{908};
t2590 = ct{909};
t2591 = ct{910};
t2597 = ct{911};
t2598 = ct{912};
t2599 = ct{913};
t26 = ct{914};
t260 = ct{915};
t2600 = ct{916};
t2605 = ct{917};
t2607 = ct{918};
t2610 = ct{919};
t2613 = ct{920};
t2615 = ct{921};
t2616 = ct{922};
t2617 = ct{923};
t2619 = ct{924};
t2620 = ct{925};
t2621 = ct{926};
t2623 = ct{927};
t2624 = ct{928};
t2627 = ct{929};
t2629 = ct{930};
t2630 = ct{931};
t2632 = ct{932};
t2634 = ct{933};
t2635 = ct{934};
t2636 = ct{935};
t2637 = ct{936};
t2638 = ct{937};
t2639 = ct{938};
t2640 = ct{939};
t2641 = ct{940};
t2646 = ct{941};
t2648 = ct{942};
t2650 = ct{943};
t2652 = ct{944};
t2655 = ct{945};
t2657 = ct{946};
t2659 = ct{947};
t2660 = ct{948};
t2661 = ct{949};
t2662 = ct{950};
t2663 = ct{951};
t2665 = ct{952};
t2666 = ct{953};
t2667 = ct{954};
t2668 = ct{955};
t2669 = ct{956};
t2671 = ct{957};
t2673 = ct{958};
t2676 = ct{959};
t2677 = ct{960};
t2678 = ct{961};
t2679 = ct{962};
t2682 = ct{963};
t2684 = ct{964};
t2688 = ct{965};
t2689 = ct{966};
t2692 = ct{967};
t2696 = ct{968};
t2698 = ct{969};
t2699 = ct{970};
t27 = ct{971};
t2700 = ct{972};
t2705 = ct{973};
t2706 = ct{974};
t2707 = ct{975};
t2708 = ct{976};
t2710 = ct{977};
t2712 = ct{978};
t2714 = ct{979};
t2715 = ct{980};
t2717 = ct{981};
t2718 = ct{982};
t2722 = ct{983};
t2723 = ct{984};
t2725 = ct{985};
t2726 = ct{986};
t2727 = ct{987};
t2728 = ct{988};
t2730 = ct{989};
t2733 = ct{990};
t2734 = ct{991};
t2735 = ct{992};
t2736 = ct{993};
t2737 = ct{994};
t2738 = ct{995};
t2740 = ct{996};
t2741 = ct{997};
t2742 = ct{998};
t2743 = ct{999};
t2744 = ct{1000};
t2746 = ct{1001};
t2749 = ct{1002};
t2750 = ct{1003};
t2751 = ct{1004};
t2752 = ct{1005};
t2754 = ct{1006};
t2756 = ct{1007};
t2758 = ct{1008};
t2759 = ct{1009};
t276 = ct{1010};
t2760 = ct{1011};
t2761 = ct{1012};
t2763 = ct{1013};
t2764 = ct{1014};
t2765 = ct{1015};
t2766 = ct{1016};
t2767 = ct{1017};
t2768 = ct{1018};
t2769 = ct{1019};
t277 = ct{1020};
t2772 = ct{1021};
t2774 = ct{1022};
t2775 = ct{1023};
t2776 = ct{1024};
t2778 = ct{1025};
t2779 = ct{1026};
t2781 = ct{1027};
t2782 = ct{1028};
t2783 = ct{1029};
t2785 = ct{1030};
t2786 = ct{1031};
t2787 = ct{1032};
t2788 = ct{1033};
t2790 = ct{1034};
t2791 = ct{1035};
t2792 = ct{1036};
t2794 = ct{1037};
t2796 = ct{1038};
t2797 = ct{1039};
t2798 = ct{1040};
t2799 = ct{1041};
t2800 = ct{1042};
t2802 = ct{1043};
t2803 = ct{1044};
t2804 = ct{1045};
t2805 = ct{1046};
t2806 = ct{1047};
t2807 = ct{1048};
t2808 = ct{1049};
t2811 = ct{1050};
t2813 = ct{1051};
t2814 = ct{1052};
t2816 = ct{1053};
t2817 = ct{1054};
t2818 = ct{1055};
t2819 = ct{1056};
t2821 = ct{1057};
t2823 = ct{1058};
t2824 = ct{1059};
t2825 = ct{1060};
t2828 = ct{1061};
t2829 = ct{1062};
t283 = ct{1063};
t2831 = ct{1064};
t2832 = ct{1065};
t2833 = ct{1066};
t2834 = ct{1067};
t2835 = ct{1068};
t2836 = ct{1069};
t2837 = ct{1070};
t2838 = ct{1071};
t2839 = ct{1072};
t284 = ct{1073};
t2841 = ct{1074};
t2842 = ct{1075};
t2843 = ct{1076};
t2844 = ct{1077};
t2845 = ct{1078};
t2846 = ct{1079};
t2847 = ct{1080};
t2848 = ct{1081};
t2849 = ct{1082};
t285 = ct{1083};
t2853 = ct{1084};
t2857 = ct{1085};
t2858 = ct{1086};
t2859 = ct{1087};
t286 = ct{1088};
t2860 = ct{1089};
t2861 = ct{1090};
t2864 = ct{1091};
t2865 = ct{1092};
t2867 = ct{1093};
t2868 = ct{1094};
t287 = ct{1095};
t2870 = ct{1096};
t2871 = ct{1097};
t2872 = ct{1098};
t2874 = ct{1099};
t2875 = ct{1100};
t2876 = ct{1101};
t2877 = ct{1102};
t2878 = ct{1103};
t2879 = ct{1104};
t288 = ct{1105};
t2880 = ct{1106};
t2882 = ct{1107};
t2883 = ct{1108};
t2884 = ct{1109};
t2886 = ct{1110};
t2887 = ct{1111};
t2889 = ct{1112};
t289 = ct{1113};
t2890 = ct{1114};
t2892 = ct{1115};
t2893 = ct{1116};
t2896 = ct{1117};
t2897 = ct{1118};
t2898 = ct{1119};
t2899 = ct{1120};
t290 = ct{1121};
t2902 = ct{1122};
t2903 = ct{1123};
t2905 = ct{1124};
t2909 = ct{1125};
t291 = ct{1126};
t2912 = ct{1127};
t2913 = ct{1128};
t2914 = ct{1129};
t2915 = ct{1130};
t2916 = ct{1131};
t2917 = ct{1132};
t2918 = ct{1133};
t2919 = ct{1134};
t292 = ct{1135};
t2920 = ct{1136};
t2921 = ct{1137};
t2926 = ct{1138};
t2927 = ct{1139};
t2928 = ct{1140};
t293 = ct{1141};
t2930 = ct{1142};
t2932 = ct{1143};
t2936 = ct{1144};
t2937 = ct{1145};
t2938 = ct{1146};
t294 = ct{1147};
t2940 = ct{1148};
t2941 = ct{1149};
t2942 = ct{1150};
t2943 = ct{1151};
t2944 = ct{1152};
t2945 = ct{1153};
t2946 = ct{1154};
t2949 = ct{1155};
t2950 = ct{1156};
t2952 = ct{1157};
t2954 = ct{1158};
t2956 = ct{1159};
t2957 = ct{1160};
t2959 = ct{1161};
t2960 = ct{1162};
t2961 = ct{1163};
t2962 = ct{1164};
t2963 = ct{1165};
t2964 = ct{1166};
t2965 = ct{1167};
t2966 = ct{1168};
t2970 = ct{1169};
t2971 = ct{1170};
t2972 = ct{1171};
t2973 = ct{1172};
t2976 = ct{1173};
t2977 = ct{1174};
t2978 = ct{1175};
t2979 = ct{1176};
t2981 = ct{1177};
t2982 = ct{1178};
t2985 = ct{1179};
t2988 = ct{1180};
t2989 = ct{1181};
t2992 = ct{1182};
t2994 = ct{1183};
t2995 = ct{1184};
t2996 = ct{1185};
t2997 = ct{1186};
t2998 = ct{1187};
t3 = ct{1188};
t3000 = ct{1189};
t3003 = ct{1190};
t3004 = ct{1191};
t3006 = ct{1192};
t3007 = ct{1193};
t3008 = ct{1194};
t3009 = ct{1195};
t3011 = ct{1196};
t3012 = ct{1197};
t3016 = ct{1198};
t3017 = ct{1199};
t3019 = ct{1200};
t3022 = ct{1201};
t3027 = ct{1202};
t3030 = ct{1203};
t3031 = ct{1204};
t3032 = ct{1205};
t3033 = ct{1206};
t3034 = ct{1207};
t3035 = ct{1208};
t3037 = ct{1209};
t3038 = ct{1210};
t304 = ct{1211};
t3040 = ct{1212};
t3041 = ct{1213};
t3042 = ct{1214};
t3043 = ct{1215};
t3047 = ct{1216};
t3049 = ct{1217};
t3050 = ct{1218};
t3051 = ct{1219};
t3054 = ct{1220};
t3059 = ct{1221};
t3060 = ct{1222};
t3061 = ct{1223};
t3062 = ct{1224};
t3063 = ct{1225};
t3064 = ct{1226};
t3065 = ct{1227};
t3069 = ct{1228};
t3070 = ct{1229};
t3075 = ct{1230};
t3076 = ct{1231};
t3078 = ct{1232};
t3080 = ct{1233};
t3082 = ct{1234};
t3083 = ct{1235};
t3084 = ct{1236};
t3085 = ct{1237};
t3086 = ct{1238};
t3087 = ct{1239};
t3089 = ct{1240};
t3090 = ct{1241};
t3091 = ct{1242};
t3092 = ct{1243};
t3093 = ct{1244};
t3094 = ct{1245};
t3096 = ct{1246};
t3097 = ct{1247};
t3098 = ct{1248};
t3099 = ct{1249};
t3100 = ct{1250};
t3102 = ct{1251};
t3103 = ct{1252};
t3104 = ct{1253};
t3105 = ct{1254};
t3106 = ct{1255};
t3107 = ct{1256};
t3108 = ct{1257};
t3109 = ct{1258};
t3110 = ct{1259};
t3112 = ct{1260};
t3113 = ct{1261};
t3115 = ct{1262};
t3117 = ct{1263};
t3121 = ct{1264};
t3122 = ct{1265};
t3127 = ct{1266};
t3128 = ct{1267};
t3131 = ct{1268};
t3132 = ct{1269};
t3134 = ct{1270};
t3135 = ct{1271};
t3136 = ct{1272};
t3138 = ct{1273};
t3139 = ct{1274};
t3145 = ct{1275};
t3146 = ct{1276};
t3147 = ct{1277};
t3149 = ct{1278};
t3151 = ct{1279};
t3153 = ct{1280};
t3155 = ct{1281};
t3156 = ct{1282};
t3157 = ct{1283};
t3158 = ct{1284};
t3160 = ct{1285};
t3161 = ct{1286};
t3162 = ct{1287};
t3163 = ct{1288};
t3164 = ct{1289};
t3166 = ct{1290};
t3167 = ct{1291};
t3168 = ct{1292};
t3169 = ct{1293};
t3170 = ct{1294};
t3171 = ct{1295};
t3173 = ct{1296};
t3174 = ct{1297};
t3176 = ct{1298};
t3177 = ct{1299};
t3178 = ct{1300};
t3179 = ct{1301};
t3180 = ct{1302};
t3181 = ct{1303};
t3183 = ct{1304};
t3184 = ct{1305};
t3185 = ct{1306};
t3186 = ct{1307};
t3187 = ct{1308};
t3189 = ct{1309};
t3190 = ct{1310};
t3192 = ct{1311};
t3193 = ct{1312};
t3196 = ct{1313};
t3199 = ct{1314};
t3200 = ct{1315};
t3203 = ct{1316};
t3204 = ct{1317};
t3206 = ct{1318};
t3207 = ct{1319};
t3210 = ct{1320};
t3212 = ct{1321};
t3213 = ct{1322};
t3214 = ct{1323};
t3215 = ct{1324};
t3216 = ct{1325};
t3217 = ct{1326};
t3218 = ct{1327};
t3221 = ct{1328};
t3222 = ct{1329};
t3223 = ct{1330};
t3224 = ct{1331};
t3226 = ct{1332};
t3230 = ct{1333};
t3231 = ct{1334};
t3232 = ct{1335};
t3233 = ct{1336};
t3235 = ct{1337};
t3236 = ct{1338};
t3239 = ct{1339};
t3240 = ct{1340};
t3241 = ct{1341};
t3243 = ct{1342};
t3244 = ct{1343};
t3245 = ct{1344};
t3247 = ct{1345};
t3248 = ct{1346};
t3250 = ct{1347};
t3251 = ct{1348};
t3252 = ct{1349};
t3254 = ct{1350};
t3256 = ct{1351};
t3257 = ct{1352};
t3258 = ct{1353};
t3260 = ct{1354};
t3261 = ct{1355};
t3262 = ct{1356};
t3263 = ct{1357};
t3265 = ct{1358};
t3266 = ct{1359};
t3267 = ct{1360};
t3270 = ct{1361};
t3271 = ct{1362};
t3272 = ct{1363};
t3273 = ct{1364};
t3276 = ct{1365};
t3277 = ct{1366};
t3278 = ct{1367};
t3279 = ct{1368};
t3280 = ct{1369};
t3284 = ct{1370};
t3285 = ct{1371};
t3286 = ct{1372};
t3287 = ct{1373};
t3289 = ct{1374};
t3290 = ct{1375};
t3296 = ct{1376};
t3299 = ct{1377};
t3300 = ct{1378};
t3301 = ct{1379};
t3302 = ct{1380};
t3303 = ct{1381};
t3304 = ct{1382};
t3305 = ct{1383};
t3306 = ct{1384};
t3307 = ct{1385};
t3308 = ct{1386};
t3311 = ct{1387};
t3312 = ct{1388};
t3313 = ct{1389};
t3314 = ct{1390};
t3315 = ct{1391};
t3316 = ct{1392};
t3317 = ct{1393};
t3319 = ct{1394};
t3320 = ct{1395};
t3321 = ct{1396};
t3322 = ct{1397};
t3323 = ct{1398};
t3324 = ct{1399};
t3325 = ct{1400};
t3326 = ct{1401};
t3327 = ct{1402};
t3328 = ct{1403};
t3329 = ct{1404};
t3330 = ct{1405};
t3331 = ct{1406};
t3332 = ct{1407};
t3333 = ct{1408};
t3334 = ct{1409};
t3335 = ct{1410};
t3336 = ct{1411};
t3337 = ct{1412};
t3338 = ct{1413};
t3339 = ct{1414};
t3340 = ct{1415};
t3341 = ct{1416};
t3342 = ct{1417};
t3343 = ct{1418};
t3344 = ct{1419};
t3347 = ct{1420};
t3349 = ct{1421};
t3351 = ct{1422};
t3352 = ct{1423};
t3354 = ct{1424};
t3355 = ct{1425};
t3357 = ct{1426};
t3359 = ct{1427};
t3360 = ct{1428};
t3361 = ct{1429};
t3367 = ct{1430};
t3368 = ct{1431};
t3370 = ct{1432};
t3372 = ct{1433};
t3373 = ct{1434};
t3375 = ct{1435};
t3376 = ct{1436};
t3377 = ct{1437};
t3378 = ct{1438};
t3379 = ct{1439};
t3380 = ct{1440};
t3381 = ct{1441};
t3384 = ct{1442};
t3385 = ct{1443};
t3386 = ct{1444};
t3387 = ct{1445};
t3388 = ct{1446};
t3390 = ct{1447};
t3391 = ct{1448};
t3392 = ct{1449};
t3393 = ct{1450};
t3396 = ct{1451};
t3397 = ct{1452};
t3399 = ct{1453};
t3401 = ct{1454};
t3402 = ct{1455};
t3403 = ct{1456};
t3404 = ct{1457};
t3405 = ct{1458};
t3406 = ct{1459};
t3407 = ct{1460};
t3408 = ct{1461};
t3409 = ct{1462};
t3410 = ct{1463};
t3411 = ct{1464};
t3412 = ct{1465};
t3413 = ct{1466};
t3414 = ct{1467};
t3415 = ct{1468};
t3416 = ct{1469};
t3419 = ct{1470};
t3420 = ct{1471};
t3423 = ct{1472};
t3424 = ct{1473};
t3425 = ct{1474};
t3426 = ct{1475};
t3427 = ct{1476};
t3429 = ct{1477};
t3430 = ct{1478};
t3431 = ct{1479};
t3432 = ct{1480};
t3433 = ct{1481};
t3434 = ct{1482};
t3437 = ct{1483};
t3438 = ct{1484};
t3439 = ct{1485};
t3440 = ct{1486};
t3441 = ct{1487};
t3442 = ct{1488};
t3443 = ct{1489};
t3444 = ct{1490};
t3445 = ct{1491};
t3446 = ct{1492};
t3447 = ct{1493};
t3448 = ct{1494};
t3449 = ct{1495};
t3454 = ct{1496};
t3455 = ct{1497};
t3456 = ct{1498};
t3457 = ct{1499};
t3458 = ct{1500};
t3459 = ct{1501};
t3460 = ct{1502};
t3463 = ct{1503};
t3464 = ct{1504};
t3465 = ct{1505};
t3466 = ct{1506};
t3467 = ct{1507};
t3469 = ct{1508};
t3470 = ct{1509};
t3471 = ct{1510};
t3472 = ct{1511};
t3473 = ct{1512};
t3474 = ct{1513};
t3475 = ct{1514};
t3476 = ct{1515};
t3477 = ct{1516};
t3478 = ct{1517};
t3479 = ct{1518};
t3480 = ct{1519};
t3481 = ct{1520};
t3482 = ct{1521};
t3483 = ct{1522};
t3484 = ct{1523};
t3485 = ct{1524};
t3486 = ct{1525};
t3487 = ct{1526};
t3488 = ct{1527};
t3489 = ct{1528};
t3490 = ct{1529};
t3491 = ct{1530};
t3492 = ct{1531};
t3494 = ct{1532};
t3495 = ct{1533};
t3496 = ct{1534};
t3497 = ct{1535};
t3499 = ct{1536};
t3500 = ct{1537};
t3501 = ct{1538};
t3502 = ct{1539};
t3504 = ct{1540};
t3506 = ct{1541};
t3508 = ct{1542};
t3509 = ct{1543};
t3510 = ct{1544};
t3511 = ct{1545};
t3512 = ct{1546};
t3513 = ct{1547};
t3515 = ct{1548};
t3516 = ct{1549};
t3517 = ct{1550};
t3521 = ct{1551};
t3522 = ct{1552};
t3523 = ct{1553};
t3524 = ct{1554};
t3526 = ct{1555};
t3528 = ct{1556};
t3529 = ct{1557};
t3530 = ct{1558};
t3531 = ct{1559};
t3532 = ct{1560};
t3533 = ct{1561};
t3534 = ct{1562};
t3535 = ct{1563};
t3536 = ct{1564};
t3537 = ct{1565};
t3538 = ct{1566};
t3539 = ct{1567};
t3540 = ct{1568};
t3541 = ct{1569};
t3542 = ct{1570};
t3543 = ct{1571};
t3544 = ct{1572};
t3545 = ct{1573};
t3547 = ct{1574};
t3548 = ct{1575};
t3550 = ct{1576};
t3552 = ct{1577};
t3553 = ct{1578};
t3554 = ct{1579};
t3555 = ct{1580};
t3556 = ct{1581};
t3557 = ct{1582};
t3558 = ct{1583};
t3559 = ct{1584};
t3562 = ct{1585};
t3563 = ct{1586};
t3565 = ct{1587};
t3570 = ct{1588};
t3571 = ct{1589};
t3575 = ct{1590};
t3576 = ct{1591};
t3578 = ct{1592};
t3579 = ct{1593};
t3581 = ct{1594};
t3582 = ct{1595};
t3583 = ct{1596};
t3584 = ct{1597};
t3587 = ct{1598};
t3588 = ct{1599};
t3591 = ct{1600};
t3594 = ct{1601};
t3595 = ct{1602};
t3596 = ct{1603};
t3597 = ct{1604};
t3598 = ct{1605};
t3600 = ct{1606};
t3601 = ct{1607};
t3602 = ct{1608};
t3603 = ct{1609};
t3605 = ct{1610};
t3609 = ct{1611};
t3610 = ct{1612};
t3611 = ct{1613};
t3613 = ct{1614};
t3614 = ct{1615};
t3615 = ct{1616};
t3616 = ct{1617};
t3617 = ct{1618};
t3618 = ct{1619};
t3619 = ct{1620};
t3620 = ct{1621};
t3621 = ct{1622};
t3622 = ct{1623};
t3623 = ct{1624};
t3624 = ct{1625};
t3625 = ct{1626};
t3626 = ct{1627};
t3627 = ct{1628};
t3629 = ct{1629};
t3630 = ct{1630};
t3632 = ct{1631};
t3634 = ct{1632};
t3635 = ct{1633};
t3637 = ct{1634};
t3638 = ct{1635};
t3639 = ct{1636};
t3643 = ct{1637};
t3644 = ct{1638};
t3646 = ct{1639};
t3647 = ct{1640};
t3648 = ct{1641};
t3649 = ct{1642};
t3651 = ct{1643};
t3652 = ct{1644};
t3653 = ct{1645};
t3654 = ct{1646};
t3655 = ct{1647};
t3657 = ct{1648};
t3658 = ct{1649};
t3659 = ct{1650};
t3660 = ct{1651};
t3661 = ct{1652};
t3664 = ct{1653};
t3666 = ct{1654};
t3667 = ct{1655};
t3668 = ct{1656};
t3670 = ct{1657};
t3671 = ct{1658};
t3672 = ct{1659};
t3673 = ct{1660};
t3674 = ct{1661};
t3675 = ct{1662};
t3676 = ct{1663};
t3677 = ct{1664};
t3678 = ct{1665};
t3679 = ct{1666};
t3680 = ct{1667};
t3681 = ct{1668};
t3682 = ct{1669};
t3683 = ct{1670};
t3684 = ct{1671};
t3685 = ct{1672};
t3686 = ct{1673};
t3687 = ct{1674};
t3689 = ct{1675};
t3690 = ct{1676};
t3693 = ct{1677};
t3697 = ct{1678};
t3698 = ct{1679};
t3699 = ct{1680};
t3700 = ct{1681};
t3701 = ct{1682};
t3702 = ct{1683};
t3704 = ct{1684};
t3708 = ct{1685};
t3709 = ct{1686};
t3710 = ct{1687};
t3711 = ct{1688};
t3716 = ct{1689};
t3719 = ct{1690};
t3720 = ct{1691};
t3721 = ct{1692};
t3722 = ct{1693};
t3723 = ct{1694};
t3724 = ct{1695};
t3730 = ct{1696};
t3735 = ct{1697};
t3736 = ct{1698};
t3738 = ct{1699};
t3739 = ct{1700};
t3741 = ct{1701};
t3742 = ct{1702};
t3744 = ct{1703};
t3745 = ct{1704};
t3746 = ct{1705};
t3747 = ct{1706};
t3748 = ct{1707};
t3749 = ct{1708};
t3750 = ct{1709};
t3751 = ct{1710};
t3752 = ct{1711};
t3755 = ct{1712};
t3756 = ct{1713};
t3757 = ct{1714};
t3758 = ct{1715};
t3759 = ct{1716};
t376 = ct{1717};
t3760 = ct{1718};
t3761 = ct{1719};
t3762 = ct{1720};
t3763 = ct{1721};
t3764 = ct{1722};
t3765 = ct{1723};
t3766 = ct{1724};
t3767 = ct{1725};
t3769 = ct{1726};
t377 = ct{1727};
t3770 = ct{1728};
t3771 = ct{1729};
t3772 = ct{1730};
t3773 = ct{1731};
t3774 = ct{1732};
t3775 = ct{1733};
t3777 = ct{1734};
t3779 = ct{1735};
t3780 = ct{1736};
t3784 = ct{1737};
t3785 = ct{1738};
t3787 = ct{1739};
t3789 = ct{1740};
t3790 = ct{1741};
t3791 = ct{1742};
t3792 = ct{1743};
t3793 = ct{1744};
t3794 = ct{1745};
t3795 = ct{1746};
t3797 = ct{1747};
t3798 = ct{1748};
t3799 = ct{1749};
t3800 = ct{1750};
t3802 = ct{1751};
t3804 = ct{1752};
t3805 = ct{1753};
t3806 = ct{1754};
t3807 = ct{1755};
t3808 = ct{1756};
t3809 = ct{1757};
t381 = ct{1758};
t3811 = ct{1759};
t3812 = ct{1760};
t3814 = ct{1761};
t3815 = ct{1762};
t3817 = ct{1763};
t3818 = ct{1764};
t3819 = ct{1765};
t382 = ct{1766};
t3820 = ct{1767};
t3823 = ct{1768};
t3824 = ct{1769};
t3825 = ct{1770};
t3826 = ct{1771};
t3828 = ct{1772};
t3829 = ct{1773};
t383 = ct{1774};
t3831 = ct{1775};
t3832 = ct{1776};
t3833 = ct{1777};
t3834 = ct{1778};
t3836 = ct{1779};
t3837 = ct{1780};
t3838 = ct{1781};
t3840 = ct{1782};
t3841 = ct{1783};
t3842 = ct{1784};
t3844 = ct{1785};
t3845 = ct{1786};
t3846 = ct{1787};
t3847 = ct{1788};
t3848 = ct{1789};
t3849 = ct{1790};
t3850 = ct{1791};
t3851 = ct{1792};
t3854 = ct{1793};
t3855 = ct{1794};
t3856 = ct{1795};
t3858 = ct{1796};
t3859 = ct{1797};
t3860 = ct{1798};
t3861 = ct{1799};
t3862 = ct{1800};
t3866 = ct{1801};
t3867 = ct{1802};
t3868 = ct{1803};
t3870 = ct{1804};
t3871 = ct{1805};
t3872 = ct{1806};
t3873 = ct{1807};
t3876 = ct{1808};
t3879 = ct{1809};
t3880 = ct{1810};
t3882 = ct{1811};
t3883 = ct{1812};
t3884 = ct{1813};
t3885 = ct{1814};
t3886 = ct{1815};
t3887 = ct{1816};
t3888 = ct{1817};
t3889 = ct{1818};
t3890 = ct{1819};
t3891 = ct{1820};
t3892 = ct{1821};
t3893 = ct{1822};
t3894 = ct{1823};
t3896 = ct{1824};
t3897 = ct{1825};
t3898 = ct{1826};
t390 = ct{1827};
t3900 = ct{1828};
t3901 = ct{1829};
t3902 = ct{1830};
t3903 = ct{1831};
t3906 = ct{1832};
t3907 = ct{1833};
t3908 = ct{1834};
t3909 = ct{1835};
t3910 = ct{1836};
t3911 = ct{1837};
t3913 = ct{1838};
t3914 = ct{1839};
t3915 = ct{1840};
t3916 = ct{1841};
t3918 = ct{1842};
t3919 = ct{1843};
t3921 = ct{1844};
t3923 = ct{1845};
t3925 = ct{1846};
t3926 = ct{1847};
t3928 = ct{1848};
t3929 = ct{1849};
t3930 = ct{1850};
t3931 = ct{1851};
t3932 = ct{1852};
t3933 = ct{1853};
t3934 = ct{1854};
t3935 = ct{1855};
t3936 = ct{1856};
t3937 = ct{1857};
t3938 = ct{1858};
t3939 = ct{1859};
t394 = ct{1860};
t3940 = ct{1861};
t3941 = ct{1862};
t3943 = ct{1863};
t3944 = ct{1864};
t3945 = ct{1865};
t3946 = ct{1866};
t3947 = ct{1867};
t3948 = ct{1868};
t3949 = ct{1869};
t3950 = ct{1870};
t3951 = ct{1871};
t3952 = ct{1872};
t3953 = ct{1873};
t3954 = ct{1874};
t3955 = ct{1875};
t3956 = ct{1876};
t3957 = ct{1877};
t3958 = ct{1878};
t3959 = ct{1879};
t3960 = ct{1880};
t3961 = ct{1881};
t3962 = ct{1882};
t3964 = ct{1883};
t3965 = ct{1884};
t3966 = ct{1885};
t3967 = ct{1886};
t3969 = ct{1887};
t3970 = ct{1888};
t3971 = ct{1889};
t3974 = ct{1890};
t3975 = ct{1891};
t3976 = ct{1892};
t3977 = ct{1893};
t3978 = ct{1894};
t3979 = ct{1895};
t3980 = ct{1896};
t3981 = ct{1897};
t3982 = ct{1898};
t3983 = ct{1899};
t3984 = ct{1900};
t3985 = ct{1901};
t3986 = ct{1902};
t3987 = ct{1903};
t3988 = ct{1904};
t3989 = ct{1905};
t3991 = ct{1906};
t3992 = ct{1907};
t3993 = ct{1908};
t3994 = ct{1909};
t3995 = ct{1910};
t3996 = ct{1911};
t3997 = ct{1912};
t3998 = ct{1913};
t4 = ct{1914};
t4000 = ct{1915};
t4001 = ct{1916};
t4003 = ct{1917};
t4005 = ct{1918};
t4006 = ct{1919};
t4007 = ct{1920};
t4008 = ct{1921};
t4009 = ct{1922};
t4010 = ct{1923};
t4011 = ct{1924};
t4012 = ct{1925};
t4013 = ct{1926};
t4014 = ct{1927};
t4015 = ct{1928};
t4016 = ct{1929};
t4017 = ct{1930};
t4019 = ct{1931};
t4020 = ct{1932};
t4021 = ct{1933};
t4022 = ct{1934};
t4023 = ct{1935};
t4024 = ct{1936};
t4025 = ct{1937};
t4026 = ct{1938};
t4027 = ct{1939};
t4028 = ct{1940};
t4029 = ct{1941};
t4030 = ct{1942};
t4031 = ct{1943};
t4032 = ct{1944};
t4033 = ct{1945};
t4034 = ct{1946};
t4035 = ct{1947};
t4036 = ct{1948};
t4037 = ct{1949};
t4038 = ct{1950};
t4040 = ct{1951};
t4041 = ct{1952};
t4042 = ct{1953};
t4043 = ct{1954};
t4044 = ct{1955};
t4046 = ct{1956};
t4047 = ct{1957};
t4048 = ct{1958};
t4050 = ct{1959};
t4051 = ct{1960};
